simulink model "lagrange_model_v2"  (R2022a)
settings: Solver=VariableStepAuto  StartTime=0.0  StopTime=10.0  RelTol=1e-3
(part 2 of 3)

== matlab function lagrange_model_v2/MATLAB Function2 ==
  data: t input; q1 input; M_inverse output; q2 input; q3 input; q4 input; q5 input
function M_inverse = fcn(t, q1, q2, q3, q4, q5)

lb1 = 0.025; l1 = 0.110; l2 = 0.38; l3 = 0.38, l4 = 0.38; l5 = 0.04;
pi = 3.14159; beta1 = 0.3; beta2 = 0.1; beta3 = 0.1; beta4 = 0.1; beta5 = 0.1;
g = 9.81; 
m1 = 2.24036; m2 = 1.380584; m3 = 0.4927734;
m4 = 1.380584; m5 = 0.130378439395373;
% Inertia Tensor 1:
Ixx1 = 0.00602313752636761; Ixy1 = 2.1208125474502E-05; Ixz1 = 0;
Iyx1 = Ixy1; Iyy1 = 0.00579248437417585; Iyz1 = 0;
Izx1 = Ixz1; Izy1 = Iyz1; Izz1 = 0.0098329939500295;

% Inertia Tensor 2:
Ixx2 = 0.00248849839; Ixy2 = 0; Ixz2 = 0;
Iyx2 = Ixy2; Iyy2 = 0.043747624; Iyz2 = 0;
Izx2 = Ixz2; Izy2 = Iyz2; Izz = 0.0425687;

% Intertia Tensor 3:
Ixx3 = 0.000993126; Ixy3 = 0; Ixz3 = 0;
Iyx3 = Ixy3; Iyy3 = 0.0088282898; Iyz3 = 0;
Izx3 = Ixz3; Izy3 = Iyz3; Izz3 = 0.008576398866;

% Intertia Tensor 4:
Ixx4 = 0.00312638; Ixy4 = 0.00354785; Ixz4 = 0.0035964956;
Iyx4 = Ixy4; Iyy4 = 0.0434376808; Iyz4 = -0.00032350627;
Izx4 = Ixz4; Izy4 = Iyz4; Izz4 = 0.042240781;

% Intertia Tensor 5:
Ixx5 = 9.85693744749924E-05; Ixy5 = 0; Ixz5 = 0;
Iyx5 = Ixy5; Iyy5 = 0.00011697309; Iyz5 = 0;
Izx5 = Ixz5; Izy5 = Iyz5; Izz5 = 0.0001866513337855;

M11 = Izz2 + 0.49277*(5.0418e-7*cos(th1(t))*sin(th2(t)) - 0.19*cos(th3(t))*(cos(th2(t) - 1.5708)*(2.6536e-6*cos(th1(t)) + 1.0*sin(th1(t))) - 1.3268e-6*sin(th2(t) - 1.5708)*cos(th1(t))) - 0.38*cos(th2(t))*(2.6536e-6*cos(th1(t)) + 1.0*sin(th1(t))) + 0.19*sin(th3(t))*(sin(th2(t) - 1.5708)*(2.6536e-6*cos(th1(t)) + 1.0*sin(th1(t))) + 1.3268e-6*cos(th2(t) - 1.5708)*cos(th1(t))))^2 + 0.13038*(5.0418e-7*sin(th1(t))*sin(th2(t)) - 0.02*cos(th5(t))*(cos(th4(t) - 3.1416)*(cos(th3(t) - 1.5708)*(cos(th2(t) - 1.5708)*(1.0*cos(th1(t)) - 2.6536e-6*sin(th1(t))) + 1.3268e-6*sin(th2(t) - 1.5708)*sin(th1(t))) - sin(th3(t) - 1.5708)*(1.0*sin(th2(t) - 1.5708)*(1.0*cos(th1(t)) - 2.6536e-6*sin(th1(t))) - 1.3268e-6*cos(th2(t) - 1.5708)*sin(th1(t)))) + 1.0*sin(th4(t) - 3.1416)*(1.0*sin(th3(t) - 1.5708)*(cos(th2(t) - 1.5708)*(1.0*cos(th1(t)) - 2.6536e-6*sin(th1(t))) + 1.3268e-6*sin(th2(t) - 1.5708)*sin(th1(t))) + cos(th3(t) - 1.5708)*(1.0*sin(th2(t) - 1.5708)*(1.0*cos(th1(t)) - 2.6536e-6*sin(th1(t))) - 1.3268e-6*cos(th2(t) - 1.5708)*sin(th1(t))))) + 0.38*cos(th2(t))*(1.0*cos(th1(t)) - 2.6536e-6*sin(th1(t))) + 0.38*cos(th3(t))*(cos(th2(t) - 1.5708)*(1.0*cos(th1(t)) - 2.6536e-6*sin(th1(t))) + 1.3268e-6*sin(th2(t) - 1.5708)*sin(th1(t))) + 0.38*cos(th4(t))*(cos(th3(t) - 1.5708)*(cos(th2(t) - 1.5708)*(1.0*cos(th1(t)) - 2.6536e-6*sin(th1(t))) + 1.3268e-6*sin(th2(t) - 1.5708)*sin(th1(t))) - sin(th3(t) - 1.5708)*(1.0*sin(th2(t) - 1.5708)*(1.0*cos(th1(t)) - 2.6536e-6*sin(th1(t))) - 1.3268e-6*cos(th2(t) - 1.5708)*sin(th1(t)))) - 0.38*sin(th3(t))*(1.0*sin(th2(t) - 1.5708)*(1.0*cos(th1(t)) - 2.6536e-6*sin(th1(t))) - 1.3268e-6*cos(th2(t) - 1.5708)*sin(th1(t))) - 0.38*sin(th4(t))*(1.0*sin(th3(t) - 1.5708)*(cos(th2(t) - 1.5708)*(1.0*cos(th1(t)) - 2.6536e-6*sin(th1(t))) + 1.3268e-6*sin(th2(t) - 1.5708)*sin(th1(t))) + cos(th3(t) - 1.5708)*(1.0*sin(th2(t) - 1.5708)*(1.0*cos(th1(t)) - 2.6536e-6*sin(th1(t))) - 1.3268e-6*cos(th2(t) - 1.5708)*sin(th1(t)))) - 0.02*sin(th5(t))*(sin(th4(t) - 3.1416)*(cos(th3(t) - 1.5708)*(cos(th2(t) - 1.5708)*(1.0*cos(th1(t)) - 2.6536e-6*sin(th1(t))) + 1.3268e-6*sin(th2(t) - 1.5708)*sin(th1(t))) - sin(th3(t) - 1.5708)*(1.0*sin(th2(t) - 1.5708)*(1.0*cos(th1(t)) - 2.6536e-6*sin(th1(t))) - 1.3268e-6*cos(th2(t) - 1.5708)*sin(th1(t)))) - cos(th4(t) - 3.1416)*(1.0*sin(th3(t) - 1.5708)*(cos(th2(t) - 1.5708)*(1.0*cos(th1(t)) - 2.6536e-6*sin(th1(t))) + 1.3268e-6*sin(th2(t) - 1.5708)*sin(th1(t))) + cos(th3(t) - 1.5708)*(1.0*sin(th2(t) - 1.5708)*(1.0*cos(th1(t)) - 2.6536e-6*sin(th1(t))) - 1.3268e-6*cos(th2(t) - 1.5708)*sin(th1(t))))))^2 + 1.3806*(5.0418e-7*cos(th1(t))*sin(th2(t)) + 0.19*sin(th4(t))*(cos(th3(t) - 1.5708)*(sin(th2(t) - 1.5708)*(2.6536e-6*cos(th1(t)) + 1.0*sin(th1(t))) + 1.3268e-6*cos(th2(t) - 1.5708)*cos(th1(t))) + sin(th3(t) - 1.5708)*(cos(th2(t) - 1.5708)*(2.6536e-6*cos(th1(t)) + 1.0*sin(th1(t))) - 1.3268e-6*sin(th2(t) - 1.5708)*cos(th1(t)))) - 0.38*cos(th3(t))*(cos(th2(t) - 1.5708)*(2.6536e-6*cos(th1(t)) + 1.0*sin(th1(t))) - 1.3268e-6*sin(th2(t) - 1.5708)*cos(th1(t))) - 0.38*cos(th2(t))*(2.6536e-6*cos(th1(t)) + 1.0*sin(th1(t))) + 0.38*sin(th3(t))*(sin(th2(t) - 1.5708)*(2.6536e-6*cos(th1(t)) + 1.0*sin(th1(t))) + 1.3268e-6*cos(th2(t) - 1.5708)*cos(th1(t))) - 0.19*cos(th4(t))*(cos(th3(t) - 1.5708)*(cos(th2(t) - 1.5708)*(2.6536e-6*cos(th1(t)) + 1.0*sin(th1(t))) - 1.3268e-6*sin(th2(t) - 1.5708)*cos(th1(t))) - 1.0*sin(th3(t) - 1.5708)*(sin(th2(t) - 1.5708)*(2.6536e-6*cos(th1(t)) + 1.0*sin(th1(t))) + 1.3268e-6*cos(th2(t) - 1.5708)*cos(th1(t)))))^2 + 0.49277*(5.0418e-7*sin(th1(t))*sin(th2(t)) + 0.38*cos(th2(t))*(1.0*cos(th1(t)) - 2.6536e-6*sin(th1(t))) + 0.19*cos(th3(t))*(cos(th2(t) - 1.5708)*(1.0*cos(th1(t)) - 2.6536e-6*sin(th1(t))) + 1.3268e-6*sin(th2(t) - 1.5708)*sin(th1(t))) - 0.19*sin(th3(t))*(1.0*sin(th2(t) - 1.5708)*(1.0*cos(th1(t)) - 2.6536e-6*sin(th1(t))) - 1.3268e-6*cos(th2(t) - 1.5708)*sin(th1(t))))^2 + 0.13038*(5.0418e-7*cos(th1(t))*sin(th2(t)) + 0.02*cos(th5(t))*(cos(th4(t) - 3.1416)*(cos(th3(t) - 1.5708)*(cos(th2(t) - 1.5708)*(2.6536e-6*cos(th1(t)) + 1.0*sin(th1(t))) - 1.3268e-6*sin(th2(t) - 1.5708)*cos(th1(t))) - 1.0*sin(th3(t) - 1.5708)*(sin(th2(t) - 1.5708)*(2.6536e-6*cos(th1(t)) + 1.0*sin(th1(t))) + 1.3268e-6*cos(th2(t) - 1.5708)*cos(th1(t)))) + sin(th4(t) - 3.1416)*(cos(th3(t) - 1.5708)*(sin(th2(t) - 1.5708)*(2.6536e-6*cos(th1(t)) + 1.0*sin(th1(t))) + 1.3268e-6*cos(th2(t) - 1.5708)*cos(th1(t))) + sin(th3(t) - 1.5708)*(cos(th2(t) - 1.5708)*(2.6536e-6*cos(th1(t)) + 1.0*sin(th1(t))) - 1.3268e-6*sin(th2(t) - 1.5708)*cos(th1(t))))) + 0.38*sin(th4(t))*(cos(th3(t) - 1.5708)*(sin(th2(t) - 1.5708)*(2.6536e-6*cos(th1(t)) + 1.0*sin(th1(t))) + 1.3268e-6*cos(th2(t) - 1.5708)*cos(th1(t))) + sin(th3(t) - 1.5708)*(cos(th2(t) - 1.5708)*(2.6536e-6*cos(th1(t)) + 1.0*sin(th1(t))) - 1.3268e-6*sin(th2(t) - 1.5708)*cos(th1(t)))) - 0.38*cos(th3(t))*(cos(th2(t) - 1.5708)*(2.6536e-6*cos(th1(t)) + 1.0*sin(th1(t))) - 1.3268e-6*sin(th2(t) - 1.5708)*cos(th1(t))) - 0.38*cos(th2(t))*(2.6536e-6*cos(th1(t)) + 1.0*sin(th1(t))) + 0.38*sin(th3(t))*(sin(th2(t) - 1.5708)*(2.6536e-6*cos(th1(t)) + 1.0*sin(th1(t))) + 1.3268e-6*cos(th2(t) - 1.5708)*cos(th1(t))) - 0.38*cos(th4(t))*(cos(th3(t) - 1.5708)*(cos(th2(t) - 1.5708)*(2.6536e-6*cos(th1(t)) + 1.0*sin(th1(t))) - 1.3268e-6*sin(th2(t) - 1.5708)*cos(th1(t))) - 1.0*sin(th3(t) - 1.5708)*(sin(th2(t) - 1.5708)*(2.6536e-6*cos(th1(t)) + 1.0*sin(th1(t))) + 1.3268e-6*cos(th2(t) - 1.5708)*cos(th1(t)))) + 0.02*sin(th5(t))*(1.0*sin(th4(t) - 3.1416)*(cos(th3(t) - 1.5708)*(cos(th2(t) - 1.5708)*(2.6536e-6*cos(th1(t)) + 1.0*sin(th1(t))) - 1.3268e-6*sin(th2(t) - 1.5708)*cos(th1(t))) - 1.0*sin(th3(t) - 1.5708)*(sin(th2(t) - 1.5708)*(2.6536e-6*cos(th1(t)) + 1.0*sin(th1(t))) + 1.3268e-6*cos(th2(t) - 1.5708)*cos(th1(t)))) - cos(th4(t) - 3.1416)*(cos(th3(t) - 1.5708)*(sin(th2(t) - 1.5708)*(2.6536e-6*cos(th1(t)) + 1.0*sin(th1(t))) + 1.3268e-6*cos(th2(t) - 1.5708)*cos(th1(t))) + sin(th3(t) - 1.5708)*(cos(th2(t) - 1.5708)*(2.6536e-6*cos(th1(t)) + 1.0*sin(th1(t))) - 1.3268e-6*sin(th2(t) - 1.5708)*cos(th1(t))))))^2 + 1.3806*(5.0418e-7*sin(th1(t))*sin(th2(t)) + 0.38*cos(th2(t))*(1.0*cos(th1(t)) - 2.6536e-6*sin(th1(t))) + 0.38*cos(th3(t))*(cos(th2(t) - 1.5708)*(1.0*cos(th1(t)) - 2.6536e-6*sin(th1(t))) + 1.3268e-6*sin(th2(t) - 1.5708)*sin(th1(t))) + 0.19*cos(th4(t))*(cos(th3(t) - 1.5708)*(cos(th2(t) - 1.5708)*(1.0*cos(th1(t)) - 2.6536e-6*sin(th1(t))) + 1.3268e-6*sin(th2(t) - 1.5708)*sin(th1(t))) - sin(th3(t) - 1.5708)*(1.0*sin(th2(t) - 1.5708)*(1.0*cos(th1(t)) - 2.6536e-6*sin(th1(t))) - 1.3268e-6*cos(th2(t) - 1.5708)*sin(th1(t)))) - 0.38*sin(th3(t))*(1.0*sin(th2(t) - 1.5708)*(1.0*cos(th1(t)) - 2.6536e-6*sin(th1(t))) - 1.3268e-6*cos(th2(t) - 1.5708)*sin(th1(t))) - 0.19*sin(th4(t))*(1.0*sin(th3(t) - 1.5708)*(cos(th2(t) - 1.5708)*(1.0*cos(th1(t)) - 2.6536e-6*sin(th1(t))) + 1.3268e-6*sin(th2(t) - 1.5708)*sin(th1(t))) + cos(th3(t) - 1.5708)*(1.0*sin(th2(t) - 1.5708)*(1.0*cos(th1(t)) - 2.6536e-6*sin(th1(t))) - 1.3268e-6*cos(th2(t) - 1.5708)*sin(th1(t)))))^2 + 1.3806*(2.5209e-7*cos(th1(t))*sin(th2(t)) - 0.19*cos(th2(t))*(2.6536e-6*cos(th1(t)) + 1.0*sin(th1(t))))^2 + 1.3806*(2.5209e-7*sin(th1(t))*sin(th2(t)) + 0.19*cos(th2(t))*(1.0*cos(th1(t)) - 2.6536e-6*sin(th1(t))))^2 + 0.060837;
M12 = Izz2 - 0.13038*(5.0418e-7*sin(th1(t))*sin(th2(t)) - 0.02*cos(th5(t))*(cos(th4(t) - 3.1416)*(cos(th3(t) - 1.5708)*(cos(th2(t) - 1.5708)*(1.0*cos(th1(t)) - 2.6536e-6*sin(th1(t))) + 1.3268e-6*sin(th2(t) - 1.5708)*sin(th1(t))) - sin(th3(t) - 1.5708)*(1.0*sin(th2(t) - 1.5708)*(1.0*cos(th1(t)) - 2.6536e-6*sin(th1(t))) - 1.3268e-6*cos(th2(t) - 1.5708)*sin(th1(t)))) + 1.0*sin(th4(t) - 3.1416)*(1.0*sin(th3(t) - 1.5708)*(cos(th2(t) - 1.5708)*(1.0*cos(th1(t)) - 2.6536e-6*sin(th1(t))) + 1.3268e-6*sin(th2(t) - 1.5708)*sin(th1(t))) + cos(th3(t) - 1.5708)*(1.0*sin(th2(t) - 1.5708)*(1.0*cos(th1(t)) - 2.6536e-6*sin(th1(t))) - 1.3268e-6*cos(th2(t) - 1.5708)*sin(th1(t))))) + 0.38*cos(th2(t))*(1.0*cos(th1(t)) - 2.6536e-6*sin(th1(t))) + 0.38*cos(th3(t))*(cos(th2(t) - 1.5708)*(1.0*cos(th1(t)) - 2.6536e-6*sin(th1(t))) + 1.3268e-6*sin(th2(t) - 1.5708)*sin(th1(t))) + 0.38*cos(th4(t))*(cos(th3(t) - 1.5708)*(cos(th2(t) - 1.5708)*(1.0*cos(th1(t)) - 2.6536e-6*sin(th1(t))) + 1.3268e-6*sin(th2(t) - 1.5708)*sin(th1(t))) - sin(th3(t) - 1.5708)*(1.0*sin(th2(t) - 1.5708)*(1.0*cos(th1(t)) - 2.6536e-6*sin(th1(t))) - 1.3268e-6*cos(th2(t) - 1.5708)*sin(th1(t)))) - 0.38*sin(th3(t))*(1.0*sin(th2(t) - 1.5708)*(1.0*cos(th1(t)) - 2.6536e-6*sin(th1(t))) - 1.3268e-6*cos(th2(t) - 1.5708)*sin(th1(t))) - 0.38*sin(th4(t))*(1.0*sin(th3(t) - 1.5708)*(cos(th2(t) - 1.5708)*(1.0*cos(th1(t)) - 2.6536e-6*sin(th1(t))) + 1.3268e-6*sin(th2(t) - 1.5708)*sin(th1(t))) + cos(th3(t) - 1.5708)*(1.0*sin(th2(t) - 1.5708)*(1.0*cos(th1(t)) - 2.6536e-6*sin(th1(t))) - 1.3268e-6*cos(th2(t) - 1.5708)*sin(th1(t)))) - 0.02*sin(th5(t))*(sin(th4(t) - 3.1416)*(cos(th3(t) - 1.5708)*(cos(th2(t) - 1.5708)*(1.0*cos(th1(t)) - 2.6536e-6*sin(th1(t))) + 1.3268e-6*sin(th2(t) - 1.5708)*sin(th1(t))) - sin(th3(t) - 1.5708)*(1.0*sin(th2(t) - 1.5708)*(1.0*cos(th1(t)) - 2.6536e-6*sin(th1(t))) - 1.3268e-6*cos(th2(t) - 1.5708)*sin(th1(t)))) - cos(th4(t) - 3.1416)*(1.0*sin(th3(t) - 1.5708)*(cos(th2(t) - 1.5708)*(1.0*cos(th1(t)) - 2.6536e-6*sin(th1(t))) + 1.3268e-6*sin(th2(t) - 1.5708)*sin(th1(t))) + cos(th3(t) - 1.5708)*(1.0*sin(th2(t) - 1.5708)*(1.0*cos(th1(t)) - 2.6536e-6*sin(th1(t))) - 1.3268e-6*cos(th2(t) - 1.5708)*sin(th1(t))))))*(0.38*cos(th3(t))*(sin(th2(t) - 1.5708)*(2.6536e-6*cos(th1(t)) + 1.0*sin(th1(t))) + 1.3268e-6*cos(th2(t) - 1.5708)*cos(th1(t))) + 0.38*sin(th2(t))*(2.6536e-6*cos(th1(t)) + 1.0*sin(th1(t))) - 0.38*sin(th4(t))*(sin(th3(t) - 1.5708)*(sin(th2(t) - 1.5708)*(2.6536e-6*cos(th1(t)) + 1.0*sin(th1(t))) + 1.3268e-6*cos(th2(t) - 1.5708)*cos(th1(t))) - cos(th3(t) - 1.5708)*(1.0*cos(th2(t) - 1.5708)*(2.6536e-6*cos(th1(t)) + 1.0*sin(th1(t))) - 1.3268e-6*sin(th2(t) - 1.5708)*cos(th1(t)))) + 0.38*sin(th3(t))*(1.0*cos(th2(t) - 1.5708)*(2.6536e-6*cos(th1(t)) + 1.0*sin(th1(t))) - 1.3268e-6*sin(th2(t) - 1.5708)*cos(th1(t))) - 0.02*cos(th5(t))*(sin(th4(t) - 3.1416)*(sin(th3(t) - 1.5708)*(sin(th2(t) - 1.5708)*(2.6536e-6*cos(th1(t)) + 1.0*sin(th1(t))) + 1.3268e-6*cos(th2(t) - 1.5708)*cos(th1(t))) - cos(th3(t) - 1.5708)*(1.0*cos(th2(t) - 1.5708)*(2.6536e-6*cos(th1(t)) + 1.0*sin(th1(t))) - 1.3268e-6*sin(th2(t) - 1.5708)*cos(th1(t)))) + cos(th4(t) - 3.1416)*(cos(th3(t) - 1.5708)*(sin(th2(t) - 1.5708)*(2.6536e-6*cos(th1(t)) + 1.0*sin(th1(t))) + 1.3268e-6*cos(th2(t) - 1.5708)*cos(th1(t))) + 1.0*sin(th3(t) - 1.5708)*(1.0*cos(th2(t) - 1.5708)*(2.6536e-6*cos(th1(t)) + 1.0*sin(th1(t))) - 1.3268e-6*sin(th2(t) - 1.5708)*cos(th1(t))))) + 0.38*cos(th4(t))*(cos(th3(t) - 1.5708)*(sin(th2(t) - 1.5708)*(2.6536e-6*cos(th1(t)) + 1.0*sin(th1(t))) + 1.3268e-6*cos(th2(t) - 1.5708)*cos(th1(t))) + 1.0*sin(th3(t) - 1.5708)*(1.0*cos(th2(t) - 1.5708)*(2.6536e-6*cos(th1(t)) + 1.0*sin(th1(t))) - 1.3268e-6*sin(th2(t) - 1.5708)*cos(th1(t)))) + 0.02*sin(th5(t))*(cos(th4(t) - 3.1416)*(sin(th3(t) - 1.5708)*(sin(th2(t) - 1.5708)*(2.6536e-6*cos(th1(t)) + 1.0*sin(th1(t))) + 1.3268e-6*cos(th2(t) - 1.5708)*cos(th1(t))) - cos(th3(t) - 1.5708)*(1.0*cos(th2(t) - 1.5708)*(2.6536e-6*cos(th1(t)) + 1.0*sin(th1(t))) - 1.3268e-6*sin(th2(t) - 1.5708)*cos(th1(t)))) - 1.0*sin(th4(t) - 3.1416)*(cos(th3(t) - 1.5708)*(sin(th2(t) - 1.5708)*(2.6536e-6*cos(th1(t)) + 1.0*sin(th1(t))) + 1.3268e-6*cos(th2(t) - 1.5708)*cos(th1(t))) + 1.0*sin(th3(t) - 1.5708)*(1.0*cos(th2(t) - 1.5708)*(2.6536e-6*cos(th1(t)) + 1.0*sin(th1(t))) - 1.3268e-6*sin(th2(t) - 1.5708)*cos(th1(t))))) + 5.0418e-7*cos(th1(t))*cos(th2(t))) + 1.3806*(2.5209e-7*cos(th1(t))*sin(th2(t)) - 0.19*cos(th2(t))*(2.6536e-6*cos(th1(t)) + 1.0*sin(th1(t))))*(2.5209e-7*cos(th2(t))*sin(th1(t)) - 0.19*sin(th2(t))*(1.0*cos(th1(t)) - 2.6536e-6*sin(th1(t)))) - 1.3806*(0.19*sin(th2(t))*(2.6536e-6*cos(th1(t)) + 1.0*sin(th1(t))) + 2.5209e-7*cos(th1(t))*cos(th2(t)))*(2.5209e-7*sin(th1(t))*sin(th2(t)) + 0.19*cos(th2(t))*(1.0*cos(th1(t)) - 2.6536e-6*sin(th1(t)))) - 1.3806*(5.0418e-7*sin(th1(t))*sin(th2(t)) + 0.38*cos(th2(t))*(1.0*cos(th1(t)) - 2.6536e-6*sin(th1(t))) + 0.38*cos(th3(t))*(cos(th2(t) - 1.5708)*(1.0*cos(th1(t)) - 2.6536e-6*sin(th1(t))) + 1.3268e-6*sin(th2(t) - 1.5708)*sin(th1(t))) + 0.19*cos(th4(t))*(cos(th3(t) - 1.5708)*(cos(th2(t) - 1.5708)*(1.0*cos(th1(t)) - 2.6536e-6*sin(th1(t))) + 1.3268e-6*sin(th2(t) - 1.5708)*sin(th1(t))) - sin(th3(t) - 1.5708)*(1.0*sin(th2(t) - 1.5708)*(1.0*cos(th1(t)) - 2.6536e-6*sin(th1(t))) - 1.3268e-6*cos(th2(t) - 1.5708)*sin(th1(t)))) - 0.38*sin(th3(t))*(1.0*sin(th2(t) - 1.5708)*(1.0*cos(th1(t)) - 2.6536e-6*sin(th1(t))) - 1.3268e-6*cos(th2(t) - 1.5708)*sin(th1(t))) - 0.19*sin(th4(t))*(1.0*sin(th3(t) - 1.5708)*(cos(th2(t) - 1.5708)*(1.0*cos(th1(t)) - 2.6536e-6*sin(th1(t))) + 1.3268e-6*sin(th2(t) - 1.5708)*sin(th1(t))) + cos(th3(t) - 1.5708)*(1.0*sin(th2(t) - 1.5708)*(1.0*cos(th1(t)) - 2.6536e-6*sin(th1(t))) - 1.3268e-6*cos(th2(t) - 1.5708)*sin(th1(t)))))*(0.38*cos(th3(t))*(sin(th2(t) - 1.5708)*(2.6536e-6*cos(th1(t)) + 1.0*sin(th1(t))) + 1.3268e-6*cos(th2(t) - 1.5708)*cos(th1(t))) + 0.38*sin(th2(t))*(2.6536e-6*cos(th1(t)) + 1.0*sin(th1(t))) - 0.19*sin(th4(t))*(sin(th3(t) - 1.5708)*(sin(th2(t) - 1.5708)*(2.6536e-6*cos(th1(t)) + 1.0*sin(th1(t))) + 1.3268e-6*cos(th2(t) - 1.5708)*cos(th1(t))) - cos(th3(t) - 1.5708)*(1.0*cos(th2(t) - 1.5708)*(2.6536e-6*cos(th1(t)) + 1.0*sin(th1(t))) - 1.3268e-6*sin(th2(t) - 1.5708)*cos(th1(t)))) + 0.38*sin(th3(t))*(1.0*cos(th2(t) - 1.5708)*(2.6536e-6*cos(th1(t)) + 1.0*sin(th1(t))) - 1.3268e-6*sin(th2(t) - 1.5708)*cos(th1(t))) + 0.19*cos(th4(t))*(cos(th3(t) - 1.5708)*(sin(th2(t) - 1.5708)*(2.6536e-6*cos(th1(t)) + 1.0*sin(th1(t))) + 1.3268e-6*cos(th2(t) - 1.5708)*cos(th1(t))) + 1.0*sin(th3(t) - 1.5708)*(1.0*cos(th2(t) - 1.5708)*(2.6536e-6*cos(th1(t)) + 1.0*sin(th1(t))) - 1.3268e-6*sin(th2(t) - 1.5708)*cos(th1(t)))) + 5.0418e-7*cos(th1(t))*cos(th2(t))) - 0.49277*(5.0418e-7*sin(th1(t))*sin(th2(t)) + 0.38*cos(th2(t))*(1.0*cos(th1(t)) - 2.6536e-6*sin(th1(t))) + 0.19*cos(th3(t))*(cos(th2(t) - 1.5708)*(1.0*cos(th1(t)) - 2.6536e-6*sin(th1(t))) + 1.3268e-6*sin(th2(t) - 1.5708)*sin(th1(t))) - 0.19*sin(th3(t))*(1.0*sin(th2(t) - 1.5708)*(1.0*cos(th1(t)) - 2.6536e-6*sin(th1(t))) - 1.3268e-6*cos(th2(t) - 1.5708)*sin(th1(t))))*(0.19*cos(th3(t))*(sin(th2(t) - 1.5708)*(2.6536e-6*cos(th1(t)) + 1.0*sin(th1(t))) + 1.3268e-6*cos(th2(t) - 1.5708)*cos(th1(t))) + 0.38*sin(th2(t))*(2.6536e-6*cos(th1(t)) + 1.0*sin(th1(t))) + 0.19*sin(th3(t))*(1.0*cos(th2(t) - 1.5708)*(2.6536e-6*cos(th1(t)) + 1.0*sin(th1(t))) - 1.3268e-6*sin(th2(t) - 1.5708)*cos(th1(t))) + 5.0418e-7*cos(th1(t))*cos(th2(t))) - 0.13038*(0.38*cos(th4(t))*(cos(th3(t) - 1.5708)*(sin(th2(t) - 1.5708)*(1.0*cos(th1(t)) - 2.6536e-6*sin(th1(t))) - 1.3268e-6*cos(th2(t) - 1.5708)*sin(th1(t))) + sin(th3(t) - 1.5708)*(cos(th2(t) - 1.5708)*(1.0*cos(th1(t)) - 2.6536e-6*sin(th1(t))) + 1.3268e-6*sin(th2(t) - 1.5708)*sin(th1(t)))) - 5.0418e-7*cos(th2(t))*sin(th1(t)) + 0.38*cos(th3(t))*(sin(th2(t) - 1.5708)*(1.0*cos(th1(t)) - 2.6536e-6*sin(th1(t))) - 1.3268e-6*cos(th2(t) - 1.5708)*sin(th1(t))) + 0.38*sin(th2(t))*(1.0*cos(th1(t)) - 2.6536e-6*sin(th1(t))) + 0.38*sin(th3(t))*(cos(th2(t) - 1.5708)*(1.0*cos(th1(t)) - 2.6536e-6*sin(th1(t))) + 1.3268e-6*sin(th2(t) - 1.5708)*sin(th1(t))) - 0.02*sin(th5(t))*(sin(th4(t) - 3.1416)*(cos(th3(t) - 1.5708)*(sin(th2(t) - 1.5708)*(1.0*cos(th1(t)) - 2.6536e-6*sin(th1(t))) - 1.3268e-6*cos(th2(t) - 1.5708)*sin(th1(t))) + sin(th3(t) - 1.5708)*(cos(th2(t) - 1.5708)*(1.0*cos(th1(t)) - 2.6536e-6*sin(th1(t))) + 1.3268e-6*sin(th2(t) - 1.5708)*sin(th1(t)))) + cos(th4(t) - 3.1416)*(cos(th3(t) - 1.5708)*(cos(th2(t) - 1.5708)*(1.0*cos(th1(t)) - 2.6536e-6*sin(th1(t))) + 1.3268e-6*sin(th2(t) - 1.5708)*sin(th1(t))) - 1.0*sin(th3(t) - 1.5708)*(sin(th2(t) - 1.5708)*(1.0*cos(th1(t)) - 2.6536e-6*sin(th1(t))) - 1.3268e-6*cos(th2(t) - 1.5708)*sin(th1(t))))) + 0.38*sin(th4(t))*(cos(th3(t) - 1.5708)*(cos(th2(t) - 1.5708)*(1.0*cos(th1(t)) - 2.6536e-6*sin(th1(t))) + 1.3268e-6*sin(th2(t) - 1.5708)*sin(th1(t))) - 1.0*sin(th3(t) - 1.5708)*(sin(th2(t) - 1.5708)*(1.0*cos(th1(t)) - 2.6536e-6*sin(th1(t))) - 1.3268e-6*cos(th2(t) - 1.5708)*sin(th1(t)))) - 0.02*cos(th5(t))*(cos(th4(t) - 3.1416)*(cos(th3(t) - 1.5708)*(sin(th2(t) - 1.5708)*(1.0*cos(th1(t)) - 2.6536e-6*sin(th1(t))) - 1.3268e-6*cos(th2(t) - 1.5708)*sin(th1(t))) + sin(th3(t) - 1.5708)*(cos(th2(t) - 1.5708)*(1.0*cos(th1(t)) - 2.6536e-6*sin(th1(t))) + 1.3268e-6*sin(th2(t) - 1.5708)*sin(th1(t)))) - 1.0*sin(th4(t) - 3.1416)*(cos(th3(t) - 1.5708)*(cos(th2(t) - 1.5708)*(1.0*cos(th1(t)) - 2.6536e-6*sin(th1(t))) + 1.3268e-6*sin(th2(t) - 1.5708)*sin(th1(t))) - 1.0*sin(th3(t) - 1.5708)*(sin(th2(t) - 1.5708)*(1.0*cos(th1(t)) - 2.6536e-6*sin(th1(t))) - 1.3268e-6*cos(th2(t) - 1.5708)*sin(th1(t))))))*(5.0418e-7*cos(th1(t))*sin(th2(t)) + 0.02*cos(th5(t))*(cos(th4(t) - 3.1416)*(cos(th3(t) - 1.5708)*(cos(th2(t) - 1.5708)*(2.6536e-6*cos(th1(t)) + 1.0*sin(th1(t))) - 1.3268e-6*sin(th2(t) - 1.5708)*cos(th1(t))) - 1.0*sin(th3(t) - 1.5708)*(sin(th2(t) - 1.5708)*(2.6536e-6*cos(th1(t)) + 1.0*sin(th1(t))) + 1.3268e-6*cos(th2(t) - 1.5708)*cos(th1(t)))) + sin(th4(t) - 3.1416)*(cos(th3(t) - 1.5708)*(sin(th2(t) - 1.5708)*(2.6536e-6*cos(th1(t)) + 1.0*sin(th1(t))) + 1.3268e-6*cos(th2(t) - 1.5708)*cos(th1(t))) + sin(th3(t) - 1.5708)*(cos(th2(t) - 1.5708)*(2.6536e-6*cos(th1(t)) + 1.0*sin(th1(t))) - 1.3268e-6*sin(th2(t) - 1.5708)*cos(th1(t))))) + 0.38*sin(th4(t))*(cos(th3(t) - 1.5708)*(sin(th2(t) - 1.5708)*(2.6536e-6*cos(th1(t)) + 1.0*sin(th1(t))) + 1.3268e-6*cos(th2(t) - 1.5708)*cos(th1(t))) + sin(th3(t) - 1.5708)*(cos(th2(t) - 1.5708)*(2.6536e-6*cos(th1(t)) + 1.0*sin(th1(t))) - 1.3268e-6*sin(th2(t) - 1.5708)*cos(th1(t)))) - 0.38*cos(th3(t))*(cos(th2(t) - 1.5708)*(2.6536e-6*cos(th1(t)) + 1.0*sin(th1(t))) - 1.3268e-6*sin(th2(t) - 1.5708)*cos(th1(t))) - 0.38*cos(th2(t))*(2.6536e-6*cos(th1(t)) + 1.0*sin(th1(t))) + 0.38*sin(th3(t))*(sin(th2(t) - 1.5708)*(2.6536e-6*cos(th1(t)) + 1.0*sin(th1(t))) + 1.3268e-6*cos(th2(t) - 1.5708)*cos(th1(t))) - 0.38*cos(th4(t))*(cos(th3(t) - 1.5708)*(cos(th2(t) - 1.5708)*(2.6536e-6*cos(th1(t)) + 1.0*sin(th1(t))) - 1.3268e-6*sin(th2(t) - 1.5708)*cos(th1(t))) - 1.0*sin(th3(t) - 1.5708)*(sin(th2(t) - 1.5708)*(2.6536e-6*cos(th1(t)) + 1.0*sin(th1(t))) + 1.3268e-6*cos(th2(t) - 1.5708)*cos(th1(t)))) + 0.02*sin(th5(t))*(1.0*sin(th4(t) - 3.1416)*(cos(th3(t) - 1.5708)*(cos(th2(t) - 1.5708)*(2.6536e-6*cos(th1(t)) + 1.0*sin(th1(t))) - 1.3268e-6*sin(th2(t) - 1.5708)*cos(th1(t))) - 1.0*sin(th3(t) - 1.5708)*(sin(th2(t) - 1.5708)*(2.6536e-6*cos(th1(t)) + 1.0*sin(th1(t))) + 1.3268e-6*cos(th2(t) - 1.5708)*cos(th1(t)))) - cos(th4(t) - 3.1416)*(cos(th3(t) - 1.5708)*(sin(th2(t) - 1.5708)*(2.6536e-6*cos(th1(t)) + 1.0*sin(th1(t))) + 1.3268e-6*cos(th2(t) - 1.5708)*cos(th1(t))) + sin(th3(t) - 1.5708)*(cos(th2(t) - 1.5708)*(2.6536e-6*cos(th1(t)) + 1.0*sin(th1(t))) - 1.3268e-6*sin(th2(t) - 1.5708)*cos(th1(t)))))) - 1.3806*(0.19*cos(th4(t))*(cos(th3(t) - 1.5708)*(sin(th2(t) - 1.5708)*(1.0*cos(th1(t)) - 2.6536e-6*sin(th1(t))) - 1.3268e-6*cos(th2(t) - 1.5708)*sin(th1(t))) + sin(th3(t) - 1.5708)*(cos(th2(t) - 1.5708)*(1.0*cos(th1(t)) - 2.6536e-6*sin(th1(t))) + 1.3268e-6*sin(th2(t) - 1.5708)*sin(th1(t)))) - 5.0418e-7*cos(th2(t))*sin(th1(t)) + 0.38*cos(th3(t))*(sin(th2(t) - 1.5708)*(1.0*cos(th1(t)) - 2.6536e-6*sin(th1(t))) - 1.3268e-6*cos(th2(t) - 1.5708)*sin(th1(t))) + 0.38*sin(th2(t))*(1.0*cos(th1(t)) - 2.6536e-6*sin(th1(t))) + 0.38*sin(th3(t))*(cos(th2(t) - 1.5708)*(1.0*cos(th1(t)) - 2.6536e-6*sin(th1(t))) + 1.3268e-6*sin(th2(t) - 1.5708)*sin(th1(t))) + 0.19*sin(th4(t))*(cos(th3(t) - 1.5708)*(cos(th2(t) - 1.5708)*(1.0*cos(th1(t)) - 2.6536e-6*sin(th1(t))) + 1.3268e-6*sin(th2(t) - 1.5708)*sin(th1(t))) - 1.0*sin(th3(t) - 1.5708)*(sin(th2(t) - 1.5708)*(1.0*cos(th1(t)) - 2.6536e-6*sin(th1(t))) - 1.3268e-6*cos(th2(t) - 1.5708)*sin(th1(t)))))*(5.0418e-7*cos(th1(t))*sin(th2(t)) + 0.19*sin(th4(t))*(cos(th3(t) - 1.5708)*(sin(th2(t) - 1.5708)*(2.6536e-6*cos(th1(t)) + 1.0*sin(th1(t))) + 1.3268e-6*cos(th2(t) - 1.5708)*cos(th1(t))) + sin(th3(t) - 1.5708)*(cos(th2(t) - 1.5708)*(2.6536e-6*cos(th1(t)) + 1.0*sin(th1(t))) - 1.3268e-6*sin(th2(t) - 1.5708)*cos(th1(t)))) - 0.38*cos(th3(t))*(cos(th2(t) - 1.5708)*(2.6536e-6*cos(th1(t)) + 1.0*sin(th1(t))) - 1.3268e-6*sin(th2(t) - 1.5708)*cos(th1(t))) - 0.38*cos(th2(t))*(2.6536e-6*cos(th1(t)) + 1.0*sin(th1(t))) + 0.38*sin(th3(t))*(sin(th2(t) - 1.5708)*(2.6536e-6*cos(th1(t)) + 1.0*sin(th1(t))) + 1.3268e-6*cos(th2(t) - 1.5708)*cos(th1(t))) - 0.19*cos(th4(t))*(cos(th3(t) - 1.5708)*(cos(th2(t) - 1.5708)*(2.6536e-6*cos(th1(t)) + 1.0*sin(th1(t))) - 1.3268e-6*sin(th2(t) - 1.5708)*cos(th1(t))) - 1.0*sin(th3(t) - 1.5708)*(sin(th2(t) - 1.5708)*(2.6536e-6*cos(th1(t)) + 1.0*sin(th1(t))) + 1.3268e-6*cos(th2(t) - 1.5708)*cos(th1(t))))) - 0.49277*(5.0418e-7*cos(th1(t))*sin(th2(t)) - 0.19*cos(th3(t))*(cos(th2(t) - 1.5708)*(2.6536e-6*cos(th1(t)) + 1.0*sin(th1(t))) - 1.3268e-6*sin(th2(t) - 1.5708)*cos(th1(t))) - 0.38*cos(th2(t))*(2.6536e-6*cos(th1(t)) + 1.0*sin(th1(t))) + 0.19*sin(th3(t))*(sin(th2(t) - 1.5708)*(2.6536e-6*cos(th1(t)) + 1.0*sin(th1(t))) + 1.3268e-6*cos(th2(t) - 1.5708)*cos(th1(t))))*(0.19*cos(th3(t))*(sin(th2(t) - 1.5708)*(1.0*cos(th1(t)) - 2.6536e-6*sin(th1(t))) - 1.3268e-6*cos(th2(t) - 1.5708)*sin(th1(t))) - 5.0418e-7*cos(th2(t))*sin(th1(t)) + 0.38*sin(th2(t))*(1.0*cos(th1(t)) - 2.6536e-6*sin(th1(t))) + 0.19*sin(th3(t))*(cos(th2(t) - 1.5708)*(1.0*cos(th1(t)) - 2.6536e-6*sin(th1(t))) + 1.3268e-6*sin(th2(t) - 1.5708)*sin(th1(t)))) + 0.051004;
M13 = 0.051004 - 1.3806*(0.38*cos(th3(t))*(sin(th2(t) - 1.5708)*(2.6536e-6*cos(th1(t)) + 1.0*sin(th1(t))) + 1.3268e-6*cos(th2(t) - 1.5708)*cos(th1(t))) - 0.19*sin(th4(t))*(sin(th3(t) - 1.5708)*(sin(th2(t) - 1.5708)*(2.6536e-6*cos(th1(t)) + 1.0*sin(th1(t))) + 1.3268e-6*cos(th2(t) - 1.5708)*cos(th1(t))) - cos(th3(t) - 1.5708)*(1.0*cos(th2(t) - 1.5708)*(2.6536e-6*cos(th1(t)) + 1.0*sin(th1(t))) - 1.3268e-6*sin(th2(t) - 1.5708)*cos(th1(t)))) + 0.38*sin(th3(t))*(1.0*cos(th2(t) - 1.5708)*(2.6536e-6*cos(th1(t)) + 1.0*sin(th1(t))) - 1.3268e-6*sin(th2(t) - 1.5708)*cos(th1(t))) + 0.19*cos(th4(t))*(cos(th3(t) - 1.5708)*(sin(th2(t) - 1.5708)*(2.6536e-6*cos(th1(t)) + 1.0*sin(th1(t))) + 1.3268e-6*cos(th2(t) - 1.5708)*cos(th1(t))) + 1.0*sin(th3(t) - 1.5708)*(1.0*cos(th2(t) - 1.5708)*(2.6536e-6*cos(th1(t)) + 1.0*sin(th1(t))) - 1.3268e-6*sin(th2(t) - 1.5708)*cos(th1(t)))))*(5.0418e-7*sin(th1(t))*sin(th2(t)) + 0.38*cos(th2(t))*(1.0*cos(th1(t)) - 2.6536e-6*sin(th1(t))) + 0.38*cos(th3(t))*(cos(th2(t) - 1.5708)*(1.0*cos(th1(t)) - 2.6536e-6*sin(th1(t))) + 1.3268e-6*sin(th2(t) - 1.5708)*sin(th1(t))) + 0.19*cos(th4(t))*(cos(th3(t) - 1.5708)*(cos(th2(t) - 1.5708)*(1.0*cos(th1(t)) - 2.6536e-6*sin(th1(t))) + 1.3268e-6*sin(th2(t) - 1.5708)*sin(th1(t))) - sin(th3(t) - 1.5708)*(1.0*sin(th2(t) - 1.5708)*(1.0*cos(th1(t)) - 2.6536e-6*sin(th1(t))) - 1.3268e-6*cos(th2(t) - 1.5708)*sin(th1(t)))) - 0.38*sin(th3(t))*(1.0*sin(th2(t) - 1.5708)*(1.0*cos(th1(t)) - 2.6536e-6*sin(th1(t))) - 1.3268e-6*cos(th2(t) - 1.5708)*sin(th1(t))) - 0.19*sin(th4(t))*(1.0*sin(th3(t) - 1.5708)*(cos(th2(t) - 1.5708)*(1.0*cos(th1(t)) - 2.6536e-6*sin(th1(t))) + 1.3268e-6*sin(th2(t) - 1.5708)*sin(th1(t))) + cos(th3(t) - 1.5708)*(1.0*sin(th2(t) - 1.5708)*(1.0*cos(th1(t)) - 2.6536e-6*sin(th1(t))) - 1.3268e-6*cos(th2(t) - 1.5708)*sin(th1(t))))) - 0.49277*(0.19*cos(th3(t))*(sin(th2(t) - 1.5708)*(2.6536e-6*cos(th1(t)) + 1.0*sin(th1(t))) + 1.3268e-6*cos(th2(t) - 1.5708)*cos(th1(t))) + 0.19*sin(th3(t))*(1.0*cos(th2(t) - 1.5708)*(2.6536e-6*cos(th1(t)) + 1.0*sin(th1(t))) - 1.3268e-6*sin(th2(t) - 1.5708)*cos(th1(t))))*(5.0418e-7*sin(th1(t))*sin(th2(t)) + 0.38*cos(th2(t))*(1.0*cos(th1(t)) - 2.6536e-6*sin(th1(t))) + 0.19*cos(th3(t))*(cos(th2(t) - 1.5708)*(1.0*cos(th1(t)) - 2.6536e-6*sin(th1(t))) + 1.3268e-6*sin(th2(t) - 1.5708)*sin(th1(t))) - 0.19*sin(th3(t))*(1.0*sin(th2(t) - 1.5708)*(1.0*cos(th1(t)) - 2.6536e-6*sin(th1(t))) - 1.3268e-6*cos(th2(t) - 1.5708)*sin(th1(t)))) - 0.13038*(0.38*cos(th4(t))*(cos(th3(t) - 1.5708)*(sin(th2(t) - 1.5708)*(1.0*cos(th1(t)) - 2.6536e-6*sin(th1(t))) - 1.3268e-6*cos(th2(t) - 1.5708)*sin(th1(t))) + sin(th3(t) - 1.5708)*(cos(th2(t) - 1.5708)*(1.0*cos(th1(t)) - 2.6536e-6*sin(th1(t))) + 1.3268e-6*sin(th2(t) - 1.5708)*sin(th1(t)))) + 0.38*cos(th3(t))*(sin(th2(t) - 1.5708)*(1.0*cos(th1(t)) - 2.6536e-6*sin(th1(t))) - 1.3268e-6*cos(th2(t) - 1.5708)*sin(th1(t))) + 0.38*sin(th3(t))*(cos(th2(t) - 1.5708)*(1.0*cos(th1(t)) - 2.6536e-6*sin(th1(t))) + 1.3268e-6*sin(th2(t) - 1.5708)*sin(th1(t))) - 0.02*sin(th5(t))*(sin(th4(t) - 3.1416)*(cos(th3(t) - 1.5708)*(sin(th2(t) - 1.5708)*(1.0*cos(th1(t)) - 2.6536e-6*sin(th1(t))) - 1.3268e-6*cos(th2(t) - 1.5708)*sin(th1(t))) + sin(th3(t) - 1.5708)*(cos(th2(t) - 1.5708)*(1.0*cos(th1(t)) - 2.6536e-6*sin(th1(t))) + 1.3268e-6*sin(th2(t) - 1.5708)*sin(th1(t)))) + cos(th4(t) - 3.1416)*(cos(th3(t) - 1.5708)*(cos(th2(t) - 1.5708)*(1.0*cos(th1(t)) - 2.6536e-6*sin(th1(t))) + 1.3268e-6*sin(th2(t) - 1.5708)*sin(th1(t))) - 1.0*sin(th3(t) - 1.5708)*(sin(th2(t) - 1.5708)*(1.0*cos(th1(t)) - 2.6536e-6*sin(th1(t))) - 1.3268e-6*cos(th2(t) - 1.5708)*sin(th1(t))))) + 0.38*sin(th4(t))*(cos(th3(t) - 1.5708)*(cos(th2(t) - 1.5708)*(1.0*cos(th1(t)) - 2.6536e-6*sin(th1(t))) + 1.3268e-6*sin(th2(t) - 1.5708)*sin(th1(t))) - 1.0*sin(th3(t) - 1.5708)*(sin(th2(t) - 1.5708)*(1.0*cos(th1(t)) - 2.6536e-6*sin(th1(t))) - 1.3268e-6*cos(th2(t) - 1.5708)*sin(th1(t)))) - 0.02*cos(th5(t))*(cos(th4(t) - 3.1416)*(cos(th3(t) - 1.5708)*(sin(th2(t) - 1.5708)*(1.0*cos(th1(t)) - 2.6536e-6*sin(th1(t))) - 1.3268e-6*cos(th2(t) - 1.5708)*sin(th1(t))) + sin(th3(t) - 1.5708)*(cos(th2(t) - 1.5708)*(1.0*cos(th1(t)) - 2.6536e-6*sin(th1(t))) + 1.3268e-6*sin(th2(t) - 1.5708)*sin(th1(t)))) - 1.0*sin(th4(t) - 3.1416)*(cos(th3(t) - 1.5708)*(cos(th2(t) - 1.5708)*(1.0*cos(th1(t)) - 2.6536e-6*sin(th1(t))) + 1.3268e-6*sin(th2(t) - 1.5708)*sin(th1(t))) - 1.0*sin(th3(t) - 1.5708)*(sin(th2(t) - 1.5708)*(1.0*cos(th1(t)) - 2.6536e-6*sin(th1(t))) - 1.3268e-6*cos(th2(t) - 1.5708)*sin(th1(t))))))*(5.0418e-7*cos(th1(t))*sin(th2(t)) + 0.02*cos(th5(t))*(cos(th4(t) - 3.1416)*(cos(th3(t) - 1.5708)*(cos(th2(t) - 1.5708)*(2.6536e-6*cos(th1(t)) + 1.0*sin(th1(t))) - 1.3268e-6*sin(th2(t) - 1.5708)*cos(th1(t))) - 1.0*sin(th3(t) - 1.5708)*(sin(th2(t) - 1.5708)*(2.6536e-6*cos(th1(t)) + 1.0*sin(th1(t))) + 1.3268e-6*cos(th2(t) - 1.5708)*cos(th1(t)))) + sin(th4(t) - 3.1416)*(cos(th3(t) - 1.5708)*(sin(th2(t) - 1.5708)*(2.6536e-6*cos(th1(t)) + 1.0*sin(th1(t))) + 1.3268e-6*cos(th2(t) - 1.5708)*cos(th1(t))) + sin(th3(t) - 1.5708)*(cos(th2(t) - 1.5708)*(2.6536e-6*cos(th1(t)) + 1.0*sin(th1(t))) - 1.3268e-6*sin(th2(t) - 1.5708)*cos(th1(t))))) + 0.38*sin(th4(t))*(cos(th3(t) - 1.5708)*(sin(th2(t) - 1.5708)*(2.6536e-6*cos(th1(t)) + 1.0*sin(th1(t))) + 1.3268e-6*cos(th2(t) - 1.5708)*cos(th1(t))) + sin(th3(t) - 1.5708)*(cos(th2(t) - 1.5708)*(2.6536e-6*cos(th1(t)) + 1.0*sin(th1(t))) - 1.3268e-6*sin(th2(t) - 1.5708)*cos(th1(t)))) - 0.38*cos(th3(t))*(cos(th2(t) - 1.5708)*(2.6536e-6*cos(th1(t)) + 1.0*sin(th1(t))) - 1.3268e-6*sin(th2(t) - 1.5708)*cos(th1(t))) - 0.38*cos(th2(t))*(2.6536e-6*cos(th1(t)) + 1.0*sin(th1(t))) + 0.38*sin(th3(t))*(sin(th2(t) - 1.5708)*(2.6536e-6*cos(th1(t)) + 1.0*sin(th1(t))) + 1.3268e-6*cos(th2(t) - 1.5708)*cos(th1(t))) - 0.38*cos(th4(t))*(cos(th3(t) - 1.5708)*(cos(th2(t) - 1.5708)*(2.6536e-6*cos(th1(t)) + 1.0*sin(th1(t))) - 1.3268e-6*sin(th2(t) - 1.5708)*cos(th1(t))) - 1.0*sin(th3(t) - 1.5708)*(sin(th2(t) - 1.5708)*(2.6536e-6*cos(th1(t)) + 1.0*sin(th1(t))) + 1.3268e-6*cos(th2(t) - 1.5708)*cos(th1(t)))) + 0.02*sin(th5(t))*(1.0*sin(th4(t) - 3.1416)*(cos(th3(t) - 1.5708)*(cos(th2(t) - 1.5708)*(2.6536e-6*cos(th1(t)) + 1.0*sin(th1(t))) - 1.3268e-6*sin(th2(t) - 1.5708)*cos(th1(t))) - 1.0*sin(th3(t) - 1.5708)*(sin(th2(t) - 1.5708)*(2.6536e-6*cos(th1(t)) + 1.0*sin(th1(t))) + 1.3268e-6*cos(th2(t) - 1.5708)*cos(th1(t)))) - cos(th4(t) - 3.1416)*(cos(th3(t) - 1.5708)*(sin(th2(t) - 1.5708)*(2.6536e-6*cos(th1(t)) + 1.0*sin(th1(t))) + 1.3268e-6*cos(th2(t) - 1.5708)*cos(th1(t))) + sin(th3(t) - 1.5708)*(cos(th2(t) - 1.5708)*(2.6536e-6*cos(th1(t)) + 1.0*sin(th1(t))) - 1.3268e-6*sin(th2(t) - 1.5708)*cos(th1(t)))))) - 1.3806*(0.19*cos(th4(t))*(cos(th3(t) - 1.5708)*(sin(th2(t) - 1.5708)*(1.0*cos(th1(t)) - 2.6536e-6*sin(th1(t))) - 1.3268e-6*cos(th2(t) - 1.5708)*sin(th1(t))) + sin(th3(t) - 1.5708)*(cos(th2(t) - 1.5708)*(1.0*cos(th1(t)) - 2.6536e-6*sin(th1(t))) + 1.3268e-6*sin(th2(t) - 1.5708)*sin(th1(t)))) + 0.38*cos(th3(t))*(sin(th2(t) - 1.5708)*(1.0*cos(th1(t)) - 2.6536e-6*sin(th1(t))) - 1.3268e-6*cos(th2(t) - 1.5708)*sin(th1(t))) + 0.38*sin(th3(t))*(cos(th2(t) - 1.5708)*(1.0*cos(th1(t)) - 2.6536e-6*sin(th1(t))) + 1.3268e-6*sin(th2(t) - 1.5708)*sin(th1(t))) + 0.19*sin(th4(t))*(cos(th3(t) - 1.5708)*(cos(th2(t) - 1.5708)*(1.0*cos(th1(t)) - 2.6536e-6*sin(th1(t))) + 1.3268e-6*sin(th2(t) - 1.5708)*sin(th1(t))) - 1.0*sin(th3(t) - 1.5708)*(sin(th2(t) - 1.5708)*(1.0*cos(th1(t)) - 2.6536e-6*sin(th1(t))) - 1.3268e-6*cos(th2(t) - 1.5708)*sin(th1(t)))))*(5.0418e-7*cos(th1(t))*sin(th2(t)) + 0.19*sin(th4(t))*(cos(th3(t) - 1.5708)*(sin(th2(t) - 1.5708)*(2.6536e-6*cos(th1(t)) + 1.0*sin(th1(t))) + 1.3268e-6*cos(th2(t) - 1.5708)*cos(th1(t))) + sin(th3(t) - 1.5708)*(cos(th2(t) - 1.5708)*(2.6536e-6*cos(th1(t)) + 1.0*sin(th1(t))) - 1.3268e-6*sin(th2(t) - 1.5708)*cos(th1(t)))) - 0.38*cos(th3(t))*(cos(th2(t) - 1.5708)*(2.6536e-6*cos(th1(t)) + 1.0*sin(th1(t))) - 1.3268e-6*sin(th2(t) - 1.5708)*cos(th1(t))) - 0.38*cos(th2(t))*(2.6536e-6*cos(th1(t)) + 1.0*sin(th1(t))) + 0.38*sin(th3(t))*(sin(th2(t) - 1.5708)*(2.6536e-6*cos(th1(t)) + 1.0*sin(th1(t))) + 1.3268e-6*cos(th2(t) - 1.5708)*cos(th1(t))) - 0.19*cos(th4(t))*(cos(th3(t) - 1.5708)*(cos(th2(t) - 1.5708)*(2.6536e-6*cos(th1(t)) + 1.0*sin(th1(t))) - 1.3268e-6*sin(th2(t) - 1.5708)*cos(th1(t))) - 1.0*sin(th3(t) - 1.5708)*(sin(th2(t) - 1.5708)*(2.6536e-6*cos(th1(t)) + 1.0*sin(th1(t))) + 1.3268e-6*cos(th2(t) - 1.5708)*cos(th1(t))))) - 0.49277*(0.19*cos(th3(t))*(sin(th2(t) - 1.5708)*(1.0*cos(th1(t)) - 2.6536e-6*sin(th1(t))) - 1.3268e-6*cos(th2(t) - 1.5708)*sin(th1(t))) + 0.19*sin(th3(t))*(cos(th2(t) - 1.5708)*(1.0*cos(th1(t)) - 2.6536e-6*sin(th1(t))) + 1.3268e-6*sin(th2(t) - 1.5708)*sin(th1(t))))*(5.0418e-7*cos(th1(t))*sin(th2(t)) - 0.19*cos(th3(t))*(cos(th2(t) - 1.5708)*(2.6536e-6*cos(th1(t)) + 1.0*sin(th1(t))) - 1.3268e-6*sin(th2(t) - 1.5708)*cos(th1(t))) - 0.38*cos(th2(t))*(2.6536e-6*cos(th1(t)) + 1.0*sin(th1(t))) + 0.19*sin(th3(t))*(sin(th2(t) - 1.5708)*(2.6536e-6*cos(th1(t)) + 1.0*sin(th1(t))) + 1.3268e-6*cos(th2(t) - 1.5708)*cos(th1(t)))) - 0.13038*(0.38*cos(th3(t))*(sin(th2(t) - 1.5708)*(2.6536e-6*cos(th1(t)) + 1.0*sin(th1(t))) + 1.3268e-6*cos(th2(t) - 1.5708)*cos(th1(t))) - 0.38*sin(th4(t))*(sin(th3(t) - 1.5708)*(sin(th2(t) - 1.5708)*(2.6536e-6*cos(th1(t)) + 1.0*sin(th1(t))) + 1.3268e-6*cos(th2(t) - 1.5708)*cos(th1(t))) - cos(th3(t) - 1.5708)*(1.0*cos(th2(t) - 1.5708)*(2.6536e-6*cos(th1(t)) + 1.0*sin(th1(t))) - 1.3268e-6*sin(th2(t) - 1.5708)*cos(th1(t)))) + 0.38*sin(th3(t))*(1.0*cos(th2(t) - 1.5708)*(2.6536e-6*cos(th1(t)) + 1.0*sin(th1(t))) - 1.3268e-6*sin(th2(t) - 1.5708)*cos(th1(t))) - 0.02*cos(th5(t))*(sin(th4(t) - 3.1416)*(sin(th3(t) - 1.5708)*(sin(th2(t) - 1.5708)*(2.6536e-6*cos(th1(t)) + 1.0*sin(th1(t))) + 1.3268e-6*cos(th2(t) - 1.5708)*cos(th1(t))) - cos(th3(t) - 1.5708)*(1.0*cos(th2(t) - 1.5708)*(2.6536e-6*cos(th1(t)) + 1.0*sin(th1(t))) - 1.3268e-6*sin(th2(t) - 1.5708)*cos(th1(t)))) + cos(th4(t) - 3.1416)*(cos(th3(t) - 1.5708)*(sin(th2(t) - 1.5708)*(2.6536e-6*cos(th1(t)) + 1.0*sin(th1(t))) + 1.3268e-6*cos(th2(t) - 1.5708)*cos(th1(t))) + 1.0*sin(th3(t) - 1.5708)*(1.0*cos(th2(t) - 1.5708)*(2.6536e-6*cos(th1(t)) + 1.0*sin(th1(t))) - 1.3268e-6*sin(th2(t) - 1.5708)*cos(th1(t))))) + 0.38*cos(th4(t))*(cos(th3(t) - 1.5708)*(sin(th2(t) - 1.5708)*(2.6536e-6*cos(th1(t)) + 1.0*sin(th1(t))) + 1.3268e-6*cos(th2(t) - 1.5708)*cos(th1(t))) + 1.0*sin(th3(t) - 1.5708)*(1.0*cos(th2(t) - 1.5708)*(2.6536e-6*cos(th1(t)) + 1.0*sin(th1(t))) - 1.3268e-6*sin(th2(t) - 1.5708)*cos(th1(t)))) + 0.02*sin(th5(t))*(cos(th4(t) - 3.1416)*(sin(th3(t) - 1.5708)*(sin(th2(t) - 1.5708)*(2.6536e-6*cos(th1(t)) + 1.0*sin(th1(t))) + 1.3268e-6*cos(th2(t) - 1.5708)*cos(th1(t))) - cos(th3(t) - 1.5708)*(1.0*cos(th2(t) - 1.5708)*(2.6536e-6*cos(th1(t)) + 1.0*sin(th1(t))) - 1.3268e-6*sin(th2(t) - 1.5708)*cos(th1(t)))) - 1.0*sin(th4(t) - 3.1416)*(cos(th3(t) - 1.5708)*(sin(th2(t) - 1.5708)*(2.6536e-6*cos(th1(t)) + 1.0*sin(th1(t))) + 1.3268e-6*cos(th2(t) - 1.5708)*cos(th1(t))) + 1.0*sin(th3(t) - 1.5708)*(1.0*cos(th2(t) - 1.5708)*(2.6536e-6*cos(th1(t)) + 1.0*sin(th1(t))) - 1.3268e-6*sin(th2(t) - 1.5708)*cos(th1(t))))))*(5.0418e-7*sin(th1(t))*sin(th2(t)) - 0.02*cos(th5(t))*(cos(th4(t) - 3.1416)*(cos(th3(t) - 1.5708)*(cos(th2(t) - 1.5708)*(1.0*cos(th1(t)) - 2.6536e-6*sin(th1(t))) + 1.3268e-6*sin(th2(t) - 1.5708)*sin(th1(t))) - sin(th3(t) - 1.5708)*(1.0*sin(th2(t) - 1.5708)*(1.0*cos(th1(t)) - 2.6536e-6*sin(th1(t))) - 1.3268e-6*cos(th2(t) - 1.5708)*sin(th1(t)))) + 1.0*sin(th4(t) - 3.1416)*(1.0*sin(th3(t) - 1.5708)*(cos(th2(t) - 1.5708)*(1.0*cos(th1(t)) - 2.6536e-6*sin(th1(t))) + 1.3268e-6*sin(th2(t) - 1.5708)*sin(th1(t))) + cos(th3(t) - 1.5708)*(1.0*sin(th2(t) - 1.5708)*(1.0*cos(th1(t)) - 2.6536e-6*sin(th1(t))) - 1.3268e-6*cos(th2(t) - 1.5708)*sin(th1(t))))) + 0.38*cos(th2(t))*(1.0*cos(th1(t)) - 2.6536e-6*sin(th1(t))) + 0.38*cos(th3(t))*(cos(th2(t) - 1.5708)*(1.0*cos(th1(t)) - 2.6536e-6*sin(th1(t))) + 1.3268e-6*sin(th2(t) - 1.5708)*sin(th1(t))) + 0.38*cos(th4(t))*(cos(th3(t) - 1.5708)*(cos(th2(t) - 1.5708)*(1.0*cos(th1(t)) - 2.6536e-6*sin(th1(t))) + 1.3268e-6*sin(th2(t) - 1.5708)*sin(th1(t))) - sin(th3(t) - 1.5708)*(1.0*sin(th2(t) - 1.5708)*(1.0*cos(th1(t)) - 2.6536e-6*sin(th1(t))) - 1.3268e-6*cos(th2(t) - 1.5708)*sin(th1(t)))) - 0.38*sin(th3(t))*(1.0*sin(th2(t) - 1.5708)*(1.0*cos(th1(t)) - 2.6536e-6*sin(th1(t))) - 1.3268e-6*cos(th2(t) - 1.5708)*sin(th1(t))) - 0.38*sin(th4(t))*(1.0*sin(th3(t) - 1.5708)*(cos(th2(t) - 1.5708)*(1.0*cos(th1(t)) - 2.6536e-6*sin(th1(t))) + 1.3268e-6*sin(th2(t) - 1.5708)*sin(th1(t))) + cos(th3(t) - 1.5708)*(1.0*sin(th2(t) - 1.5708)*(1.0*cos(th1(t)) - 2.6536e-6*sin(th1(t))) - 1.3268e-6*cos(th2(t) - 1.5708)*sin(th1(t)))) - 0.02*sin(th5(t))*(sin(th4(t) - 3.1416)*(cos(th3(t) - 1.5708)*(cos(th2(t) - 1.5708)*(1.0*cos(th1(t)) - 2.6536e-6*sin(th1(t))) + 1.3268e-6*sin(th2(t) - 1.5708)*sin(th1(t))) - sin(th3(t) - 1.5708)*(1.0*sin(th2(t) - 1.5708)*(1.0*cos(th1(t)) - 2.6536e-6*sin(th1(t))) - 1.3268e-6*cos(th2(t) - 1.5708)*sin(th1(t)))) - cos(th4(t) - 3.1416)*(1.0*sin(th3(t) - 1.5708)*(cos(th2(t) - 1.5708)*(1.0*cos(th1(t)) - 2.6536e-6*sin(th1(t))) + 1.3268e-6*sin(th2(t) - 1.5708)*sin(th1(t))) + cos(th3(t) - 1.5708)*(1.0*sin(th2(t) - 1.5708)*(1.0*cos(th1(t)) - 2.6536e-6*sin(th1(t))) - 1.3268e-6*cos(th2(t) - 1.5708)*sin(th1(t))))));
M14 = 0.13038*(0.38*sin(th4(t))*(sin(th3(t) - 1.5708)*(sin(th2(t) - 1.5708)*(2.6536e-6*cos(th1(t)) + 1.0*sin(th1(t))) + 1.3268e-6*cos(th2(t) - 1.5708)*cos(th1(t))) - cos(th3(t) - 1.5708)*(1.0*cos(th2(t) - 1.5708)*(2.6536e-6*cos(th1(t)) + 1.0*sin(th1(t))) - 1.3268e-6*sin(th2(t) - 1.5708)*cos(th1(t)))) - 0.02*cos(th5(t))*(sin(th4(t) - 3.1416)*(sin(th3(t) - 1.5708)*(sin(th2(t) - 1.5708)*(2.6536e-6*cos(th1(t)) + 1.0*sin(th1(t))) + 1.3268e-6*cos(th2(t) - 1.5708)*cos(th1(t))) - cos(th3(t) - 1.5708)*(1.0*cos(th2(t) - 1.5708)*(2.6536e-6*cos(th1(t)) + 1.0*sin(th1(t))) - 1.3268e-6*sin(th2(t) - 1.5708)*cos(th1(t)))) + cos(th4(t) - 3.1416)*(cos(th3(t) - 1.5708)*(sin(th2(t) - 1.5708)*(2.6536e-6*cos(th1(t)) + 1.0*sin(th1(t))) + 1.3268e-6*cos(th2(t) - 1.5708)*cos(th1(t))) + 1.0*sin(th3(t) - 1.5708)*(1.0*cos(th2(t) - 1.5708)*(2.6536e-6*cos(th1(t)) + 1.0*sin(th1(t))) - 1.3268e-6*sin(th2(t) - 1.5708)*cos(th1(t))))) - 0.38*cos(th4(t))*(cos(th3(t) - 1.5708)*(sin(th2(t) - 1.5708)*(2.6536e-6*cos(th1(t)) + 1.0*sin(th1(t))) + 1.3268e-6*cos(th2(t) - 1.5708)*cos(th1(t))) + 1.0*sin(th3(t) - 1.5708)*(1.0*cos(th2(t) - 1.5708)*(2.6536e-6*cos(th1(t)) + 1.0*sin(th1(t))) - 1.3268e-6*sin(th2(t) - 1.5708)*cos(th1(t)))) + 0.02*sin(th5(t))*(cos(th4(t) - 3.1416)*(sin(th3(t) - 1.5708)*(sin(th2(t) - 1.5708)*(2.6536e-6*cos(th1(t)) + 1.0*sin(th1(t))) + 1.3268e-6*cos(th2(t) - 1.5708)*cos(th1(t))) - cos(th3(t) - 1.5708)*(1.0*cos(th2(t) - 1.5708)*(2.6536e-6*cos(th1(t)) + 1.0*sin(th1(t))) - 1.3268e-6*sin(th2(t) - 1.5708)*cos(th1(t)))) - 1.0*sin(th4(t) - 3.1416)*(cos(th3(t) - 1.5708)*(sin(th2(t) - 1.5708)*(2.6536e-6*cos(th1(t)) + 1.0*sin(th1(t))) + 1.3268e-6*cos(th2(t) - 1.5708)*cos(th1(t))) + 1.0*sin(th3(t) - 1.5708)*(1.0*cos(th2(t) - 1.5708)*(2.6536e-6*cos(th1(t)) + 1.0*sin(th1(t))) - 1.3268e-6*sin(th2(t) - 1.5708)*cos(th1(t))))))*(5.0418e-7*sin(th1(t))*sin(th2(t)) - 0.02*cos(th5(t))*(cos(th4(t) - 3.1416)*(cos(th3(t) - 1.5708)*(cos(th2(t) - 1.5708)*(1.0*cos(th1(t)) - 2.6536e-6*sin(th1(t))) + 1.3268e-6*sin(th2(t) - 1.5708)*sin(th1(t))) - sin(th3(t) - 1.5708)*(1.0*sin(th2(t) - 1.5708)*(1.0*cos(th1(t)) - 2.6536e-6*sin(th1(t))) - 1.3268e-6*cos(th2(t) - 1.5708)*sin(th1(t)))) + 1.0*sin(th4(t) - 3.1416)*(1.0*sin(th3(t) - 1.5708)*(cos(th2(t) - 1.5708)*(1.0*cos(th1(t)) - 2.6536e-6*sin(th1(t))) + 1.3268e-6*sin(th2(t) - 1.5708)*sin(th1(t))) + cos(th3(t) - 1.5708)*(1.0*sin(th2(t) - 1.5708)*(1.0*cos(th1(t)) - 2.6536e-6*sin(th1(t))) - 1.3268e-6*cos(th2(t) - 1.5708)*sin(th1(t))))) + 0.38*cos(th2(t))*(1.0*cos(th1(t)) - 2.6536e-6*sin(th1(t))) + 0.38*cos(th3(t))*(cos(th2(t) - 1.5708)*(1.0*cos(th1(t)) - 2.6536e-6*sin(th1(t))) + 1.3268e-6*sin(th2(t) - 1.5708)*sin(th1(t))) + 0.38*cos(th4(t))*(cos(th3(t) - 1.5708)*(cos(th2(t) - 1.5708)*(1.0*cos(th1(t)) - 2.6536e-6*sin(th1(t))) + 1.3268e-6*sin(th2(t) - 1.5708)*sin(th1(t))) - sin(th3(t) - 1.5708)*(1.0*sin(th2(t) - 1.5708)*(1.0*cos(th1(t)) - 2.6536e-6*sin(th1(t))) - 1.3268e-6*cos(th2(t) - 1.5708)*sin(th1(t)))) - 0.38*sin(th3(t))*(1.0*sin(th2(t) - 1.5708)*(1.0*cos(th1(t)) - 2.6536e-6*sin(th1(t))) - 1.3268e-6*cos(th2(t) - 1.5708)*sin(th1(t))) - 0.38*sin(th4(t))*(1.0*sin(th3(t) - 1.5708)*(cos(th2(t) - 1.5708)*(1.0*cos(th1(t)) - 2.6536e-6*sin(th1(t))) + 1.3268e-6*sin(th2(t) - 1.5708)*sin(th1(t))) + cos(th3(t) - 1.5708)*(1.0*sin(th2(t) - 1.5708)*(1.0*cos(th1(t)) - 2.6536e-6*sin(th1(t))) - 1.3268e-6*cos(th2(t) - 1.5708)*sin(th1(t)))) - 0.02*sin(th5(t))*(sin(th4(t) - 3.1416)*(cos(th3(t) - 1.5708)*(cos(th2(t) - 1.5708)*(1.0*cos(th1(t)) - 2.6536e-6*sin(th1(t))) + 1.3268e-6*sin(th2(t) - 1.5708)*sin(th1(t))) - sin(th3(t) - 1.5708)*(1.0*sin(th2(t) - 1.5708)*(1.0*cos(th1(t)) - 2.6536e-6*sin(th1(t))) - 1.3268e-6*cos(th2(t) - 1.5708)*sin(th1(t)))) - cos(th4(t) - 3.1416)*(1.0*sin(th3(t) - 1.5708)*(cos(th2(t) - 1.5708)*(1.0*cos(th1(t)) - 2.6536e-6*sin(th1(t))) + 1.3268e-6*sin(th2(t) - 1.5708)*sin(th1(t))) + cos(th3(t) - 1.5708)*(1.0*sin(th2(t) - 1.5708)*(1.0*cos(th1(t)) - 2.6536e-6*sin(th1(t))) - 1.3268e-6*cos(th2(t) - 1.5708)*sin(th1(t)))))) - 1.3806*(0.19*cos(th4(t))*(cos(th3(t) - 1.5708)*(sin(th2(t) - 1.5708)*(1.0*cos(th1(t)) - 2.6536e-6*sin(th1(t))) - 1.3268e-6*cos(th2(t) - 1.5708)*sin(th1(t))) + sin(th3(t) - 1.5708)*(cos(th2(t) - 1.5708)*(1.0*cos(th1(t)) - 2.6536e-6*sin(th1(t))) + 1.3268e-6*sin(th2(t) - 1.5708)*sin(th1(t)))) + 0.19*sin(th4(t))*(cos(th3(t) - 1.5708)*(cos(th2(t) - 1.5708)*(1.0*cos(th1(t)) - 2.6536e-6*sin(th1(t))) + 1.3268e-6*sin(th2(t) - 1.5708)*sin(th1(t))) - 1.0*sin(th3(t) - 1.5708)*(sin(th2(t) - 1.5708)*(1.0*cos(th1(t)) - 2.6536e-6*sin(th1(t))) - 1.3268e-6*cos(th2(t) - 1.5708)*sin(th1(t)))))*(5.0418e-7*cos(th1(t))*sin(th2(t)) + 0.19*sin(th4(t))*(cos(th3(t) - 1.5708)*(sin(th2(t) - 1.5708)*(2.6536e-6*cos(th1(t)) + 1.0*sin(th1(t))) + 1.3268e-6*cos(th2(t) - 1.5708)*cos(th1(t))) + sin(th3(t) - 1.5708)*(cos(th2(t) - 1.5708)*(2.6536e-6*cos(th1(t)) + 1.0*sin(th1(t))) - 1.3268e-6*sin(th2(t) - 1.5708)*cos(th1(t)))) - 0.38*cos(th3(t))*(cos(th2(t) - 1.5708)*(2.6536e-6*cos(th1(t)) + 1.0*sin(th1(t))) - 1.3268e-6*sin(th2(t) - 1.5708)*cos(th1(t))) - 0.38*cos(th2(t))*(2.6536e-6*cos(th1(t)) + 1.0*sin(th1(t))) + 0.38*sin(th3(t))*(sin(th2(t) - 1.5708)*(2.6536e-6*cos(th1(t)) + 1.0*sin(th1(t))) + 1.3268e-6*cos(th2(t) - 1.5708)*cos(th1(t))) - 0.19*cos(th4(t))*(cos(th3(t) - 1.5708)*(cos(th2(t) - 1.5708)*(2.6536e-6*cos(th1(t)) + 1.0*sin(th1(t))) - 1.3268e-6*sin(th2(t) - 1.5708)*cos(th1(t))) - 1.0*sin(th3(t) - 1.5708)*(sin(th2(t) - 1.5708)*(2.6536e-6*cos(th1(t)) + 1.0*sin(th1(t))) + 1.3268e-6*cos(th2(t) - 1.5708)*cos(th1(t))))) - 0.13038*(0.38*cos(th4(t))*(cos(th3(t) - 1.5708)*(sin(th2(t) - 1.5708)*(1.0*cos(th1(t)) - 2.6536e-6*sin(th1(t))) - 1.3268e-6*cos(th2(t) - 1.5708)*sin(th1(t))) + sin(th3(t) - 1.5708)*(cos(th2(t) - 1.5708)*(1.0*cos(th1(t)) - 2.6536e-6*sin(th1(t))) + 1.3268e-6*sin(th2(t) - 1.5708)*sin(th1(t)))) + 0.02*sin(th5(t))*(sin(th4(t) - 3.1416)*(cos(th3(t) - 1.5708)*(sin(th2(t) - 1.5708)*(1.0*cos(th1(t)) - 2.6536e-6*sin(th1(t))) - 1.3268e-6*cos(th2(t) - 1.5708)*sin(th1(t))) + sin(th3(t) - 1.5708)*(cos(th2(t) - 1.5708)*(1.0*cos(th1(t)) - 2.6536e-6*sin(th1(t))) + 1.3268e-6*sin(th2(t) - 1.5708)*sin(th1(t)))) + cos(th4(t) - 3.1416)*(cos(th3(t) - 1.5708)*(cos(th2(t) - 1.5708)*(1.0*cos(th1(t)) - 2.6536e-6*sin(th1(t))) + 1.3268e-6*sin(th2(t) - 1.5708)*sin(th1(t))) - 1.0*sin(th3(t) - 1.5708)*(sin(th2(t) - 1.5708)*(1.0*cos(th1(t)) - 2.6536e-6*sin(th1(t))) - 1.3268e-6*cos(th2(t) - 1.5708)*sin(th1(t))))) + 0.38*sin(th4(t))*(cos(th3(t) - 1.5708)*(cos(th2(t) - 1.5708)*(1.0*cos(th1(t)) - 2.6536e-6*sin(th1(t))) + 1.3268e-6*sin(th2(t) - 1.5708)*sin(th1(t))) - 1.0*sin(th3(t) - 1.5708)*(sin(th2(t) - 1.5708)*(1.0*cos(th1(t)) - 2.6536e-6*sin(th1(t))) - 1.3268e-6*cos(th2(t) - 1.5708)*sin(th1(t)))) + 0.02*cos(th5(t))*(cos(th4(t) - 3.1416)*(cos(th3(t) - 1.5708)*(sin(th2(t) - 1.5708)*(1.0*cos(th1(t)) - 2.6536e-6*sin(th1(t))) - 1.3268e-6*cos(th2(t) - 1.5708)*sin(th1(t))) + sin(th3(t) - 1.5708)*(cos(th2(t) - 1.5708)*(1.0*cos(th1(t)) - 2.6536e-6*sin(th1(t))) + 1.3268e-6*sin(th2(t) - 1.5708)*sin(th1(t)))) - 1.0*sin(th4(t) - 3.1416)*(cos(th3(t) - 1.5708)*(cos(th2(t) - 1.5708)*(1.0*cos(th1(t)) - 2.6536e-6*sin(th1(t))) + 1.3268e-6*sin(th2(t) - 1.5708)*sin(th1(t))) - 1.0*sin(th3(t) - 1.5708)*(sin(th2(t) - 1.5708)*(1.0*cos(th1(t)) - 2.6536e-6*sin(th1(t))) - 1.3268e-6*cos(th2(t) - 1.5708)*sin(th1(t))))))*(5.0418e-7*cos(th1(t))*sin(th2(t)) + 0.02*cos(th5(t))*(cos(th4(t) - 3.1416)*(cos(th3(t) - 1.5708)*(cos(th2(t) - 1.5708)*(2.6536e-6*cos(th1(t)) + 1.0*sin(th1(t))) - 1.3268e-6*sin(th2(t) - 1.5708)*cos(th1(t))) - 1.0*sin(th3(t) - 1.5708)*(sin(th2(t) - 1.5708)*(2.6536e-6*cos(th1(t)) + 1.0*sin(th1(t))) + 1.3268e-6*cos(th2(t) - 1.5708)*cos(th1(t)))) + sin(th4(t) - 3.1416)*(cos(th3(t) - 1.5708)*(sin(th2(t) - 1.5708)*(2.6536e-6*cos(th1(t)) + 1.0*sin(th1(t))) + 1.3268e-6*cos(th2(t) - 1.5708)*cos(th1(t))) + sin(th3(t) - 1.5708)*(cos(th2(t) - 1.5708)*(2.6536e-6*cos(th1(t)) + 1.0*sin(th1(t))) - 1.3268e-6*sin(th2(t) - 1.5708)*cos(th1(t))))) + 0.38*sin(th4(t))*(cos(th3(t) - 1.5708)*(sin(th2(t) - 1.5708)*(2.6536e-6*cos(th1(t)) + 1.0*sin(th1(t))) + 1.3268e-6*cos(th2(t) - 1.5708)*cos(th1(t))) + sin(th3(t) - 1.5708)*(cos(th2(t) - 1.5708)*(2.6536e-6*cos(th1(t)) + 1.0*sin(th1(t))) - 1.3268e-6*sin(th2(t) - 1.5708)*cos(th1(t)))) - 0.38*cos(th3(t))*(cos(th2(t) - 1.5708)*(2.6536e-6*cos(th1(t)) + 1.0*sin(th1(t))) - 1.3268e-6*sin(th2(t) - 1.5708)*cos(th1(t))) - 0.38*cos(th2(t))*(2.6536e-6*cos(th1(t)) + 1.0*sin(th1(t))) + 0.38*sin(th3(t))*(sin(th2(t) - 1.5708)*(2.6536e-6*cos(th1(t)) + 1.0*sin(th1(t))) + 1.3268e-6*cos(th2(t) - 1.5708)*cos(th1(t))) - 0.38*cos(th4(t))*(cos(th3(t) - 1.5708)*(cos(th2(t) - 1.5708)*(2.6536e-6*cos(th1(t)) + 1.0*sin(th1(t))) - 1.3268e-6*sin(th2(t) - 1.5708)*cos(th1(t))) - 1.0*sin(th3(t) - 1.5708)*(sin(th2(t) - 1.5708)*(2.6536e-6*cos(th1(t)) + 1.0*sin(th1(t))) + 1.3268e-6*cos(th2(t) - 1.5708)*cos(th1(t)))) + 0.02*sin(th5(t))*(1.0*sin(th4(t) - 3.1416)*(cos(th3(t) - 1.5708)*(cos(th2(t) - 1.5708)*(2.6536e-6*cos(th1(t)) + 1.0*sin(th1(t))) - 1.3268e-6*sin(th2(t) - 1.5708)*cos(th1(t))) - 1.0*sin(th3(t) - 1.5708)*(sin(th2(t) - 1.5708)*(2.6536e-6*cos(th1(t)) + 1.0*sin(th1(t))) + 1.3268e-6*cos(th2(t) - 1.5708)*cos(th1(t)))) - cos(th4(t) - 3.1416)*(cos(th3(t) - 1.5708)*(sin(th2(t) - 1.5708)*(2.6536e-6*cos(th1(t)) + 1.0*sin(th1(t))) + 1.3268e-6*cos(th2(t) - 1.5708)*cos(th1(t))) + sin(th3(t) - 1.5708)*(cos(th2(t) - 1.5708)*(2.6536e-6*cos(th1(t)) + 1.0*sin(th1(t))) - 1.3268e-6*sin(th2(t) - 1.5708)*cos(th1(t)))))) + 1.3806*(0.19*sin(th4(t))*(sin(th3(t) - 1.5708)*(sin(th2(t) - 1.5708)*(2.6536e-6*cos(th1(t)) + 1.0*sin(th1(t))) + 1.3268e-6*cos(th2(t) - 1.5708)*cos(th1(t))) - cos(th3(t) - 1.5708)*(1.0*cos(th2(t) - 1.5708)*(2.6536e-6*cos(th1(t)) + 1.0*sin(th1(t))) - 1.3268e-6*sin(th2(t) - 1.5708)*cos(th1(t)))) - 0.19*cos(th4(t))*(cos(th3(t) - 1.5708)*(sin(th2(t) - 1.5708)*(2.6536e-6*cos(th1(t)) + 1.0*sin(th1(t))) + 1.3268e-6*cos(th2(t) - 1.5708)*cos(th1(t))) + 1.0*sin(th3(t) - 1.5708)*(1.0*cos(th2(t) - 1.5708)*(2.6536e-6*cos(th1(t)) + 1.0*sin(th1(t))) - 1.3268e-6*sin(th2(t) - 1.5708)*cos(th1(t)))))*(5.0418e-7*sin(th1(t))*sin(th2(t)) + 0.38*cos(th2(t))*(1.0*cos(th1(t)) - 2.6536e-6*sin(th1(t))) + 0.38*cos(th3(t))*(cos(th2(t) - 1.5708)*(1.0*cos(th1(t)) - 2.6536e-6*sin(th1(t))) + 1.3268e-6*sin(th2(t) - 1.5708)*sin(th1(t))) + 0.19*cos(th4(t))*(cos(th3(t) - 1.5708)*(cos(th2(t) - 1.5708)*(1.0*cos(th1(t)) - 2.6536e-6*sin(th1(t))) + 1.3268e-6*sin(th2(t) - 1.5708)*sin(th1(t))) - sin(th3(t) - 1.5708)*(1.0*sin(th2(t) - 1.5708)*(1.0*cos(th1(t)) - 2.6536e-6*sin(th1(t))) - 1.3268e-6*cos(th2(t) - 1.5708)*sin(th1(t)))) - 0.38*sin(th3(t))*(1.0*sin(th2(t) - 1.5708)*(1.0*cos(th1(t)) - 2.6536e-6*sin(th1(t))) - 1.3268e-6*cos(th2(t) - 1.5708)*sin(th1(t))) - 0.19*sin(th4(t))*(1.0*sin(th3(t) - 1.5708)*(cos(th2(t) - 1.5708)*(1.0*cos(th1(t)) - 2.6536e-6*sin(th1(t))) + 1.3268e-6*sin(th2(t) - 1.5708)*sin(th1(t))) + cos(th3(t) - 1.5708)*(1.0*sin(th2(t) - 1.5708)*(1.0*cos(th1(t)) - 2.6536e-6*sin(th1(t))) - 1.3268e-6*cos(th2(t) - 1.5708)*sin(th1(t))))) + 0.042427;
M15 = 0.13038*(0.02*sin(th5(t))*(sin(th4(t) - 3.1416)*(cos(th3(t) - 1.5708)*(sin(th2(t) - 1.5708)*(1.0*cos(th1(t)) - 2.6536e-6*sin(th1(t))) - 1.3268e-6*cos(th2(t) - 1.5708)*sin(th1(t))) + sin(th3(t) - 1.5708)*(cos(th2(t) - 1.5708)*(1.0*cos(th1(t)) - 2.6536e-6*sin(th1(t))) + 1.3268e-6*sin(th2(t) - 1.5708)*sin(th1(t)))) + cos(th4(t) - 3.1416)*(cos(th3(t) - 1.5708)*(cos(th2(t) - 1.5708)*(1.0*cos(th1(t)) - 2.6536e-6*sin(th1(t))) + 1.3268e-6*sin(th2(t) - 1.5708)*sin(th1(t))) - 1.0*sin(th3(t) - 1.5708)*(sin(th2(t) - 1.5708)*(1.0*cos(th1(t)) - 2.6536e-6*sin(th1(t))) - 1.3268e-6*cos(th2(t) - 1.5708)*sin(th1(t))))) + 0.02*cos(th5(t))*(cos(th4(t) - 3.1416)*(cos(th3(t) - 1.5708)*(sin(th2(t) - 1.5708)*(1.0*cos(th1(t)) - 2.6536e-6*sin(th1(t))) - 1.3268e-6*cos(th2(t) - 1.5708)*sin(th1(t))) + sin(th3(t) - 1.5708)*(cos(th2(t) - 1.5708)*(1.0*cos(th1(t)) - 2.6536e-6*sin(th1(t))) + 1.3268e-6*sin(th2(t) - 1.5708)*sin(th1(t)))) - 1.0*sin(th4(t) - 3.1416)*(cos(th3(t) - 1.5708)*(cos(th2(t) - 1.5708)*(1.0*cos(th1(t)) - 2.6536e-6*sin(th1(t))) + 1.3268e-6*sin(th2(t) - 1.5708)*sin(th1(t))) - 1.0*sin(th3(t) - 1.5708)*(sin(th2(t) - 1.5708)*(1.0*cos(th1(t)) - 2.6536e-6*sin(th1(t))) - 1.3268e-6*cos(th2(t) - 1.5708)*sin(th1(t))))))*(5.0418e-7*cos(th1(t))*sin(th2(t)) + 0.02*cos(th5(t))*(cos(th4(t) - 3.1416)*(cos(th3(t) - 1.5708)*(cos(th2(t) - 1.5708)*(2.6536e-6*cos(th1(t)) + 1.0*sin(th1(t))) - 1.3268e-6*sin(th2(t) - 1.5708)*cos(th1(t))) - 1.0*sin(th3(t) - 1.5708)*(sin(th2(t) - 1.5708)*(2.6536e-6*cos(th1(t)) + 1.0*sin(th1(t))) + 1.3268e-6*cos(th2(t) - 1.5708)*cos(th1(t)))) + sin(th4(t) - 3.1416)*(cos(th3(t) - 1.5708)*(sin(th2(t) - 1.5708)*(2.6536e-6*cos(th1(t)) + 1.0*sin(th1(t))) + 1.3268e-6*cos(th2(t) - 1.5708)*cos(th1(t))) + sin(th3(t) - 1.5708)*(cos(th2(t) - 1.5708)*(2.6536e-6*cos(th1(t)) + 1.0*sin(th1(t))) - 1.3268e-6*sin(th2(t) - 1.5708)*cos(th1(t))))) + 0.38*sin(th4(t))*(cos(th3(t) - 1.5708)*(sin(th2(t) - 1.5708)*(2.6536e-6*cos(th1(t)) + 1.0*sin(th1(t))) + 1.3268e-6*cos(th2(t) - 1.5708)*cos(th1(t))) + sin(th3(t) - 1.5708)*(cos(th2(t) - 1.5708)*(2.6536e-6*cos(th1(t)) + 1.0*sin(th1(t))) - 1.3268e-6*sin(th2(t) - 1.5708)*cos(th1(t)))) - 0.38*cos(th3(t))*(cos(th2(t) - 1.5708)*(2.6536e-6*cos(th1(t)) + 1.0*sin(th1(t))) - 1.3268e-6*sin(th2(t) - 1.5708)*cos(th1(t))) - 0.38*cos(th2(t))*(2.6536e-6*cos(th1(t)) + 1.0*sin(th1(t))) + 0.38*sin(th3(t))*(sin(th2(t) - 1.5708)*(2.6536e-6*cos(th1(t)) + 1.0*sin(th1(t))) + 1.3268e-6*cos(th2(t) - 1.5708)*cos(th1(t))) - 0.38*cos(th4(t))*(cos(th3(t) - 1.5708)*(cos(th2(t) - 1.5708)*(2.6536e-6*cos(th1(t)) + 1.0*sin(th1(t))) - 1.3268e-6*sin(th2(t) - 1.5708)*cos(th1(t))) - 1.0*sin(th3(t) - 1.5708)*(sin(th2(t) - 1.5708)*(2.6536e-6*cos(th1(t)) + 1.0*sin(th1(t))) + 1.3268e-6*cos(th2(t) - 1.5708)*cos(th1(t)))) + 0.02*sin(th5(t))*(1.0*sin(th4(t) - 3.1416)*(cos(th3(t) - 1.5708)*(cos(th2(t) - 1.5708)*(2.6536e-6*cos(th1(t)) + 1.0*sin(th1(t))) - 1.3268e-6*sin(th2(t) - 1.5708)*cos(th1(t))) - 1.0*sin(th3(t) - 1.5708)*(sin(th2(t) - 1.5708)*(2.6536e-6*cos(th1(t)) + 1.0*sin(th1(t))) + 1.3268e-6*cos(th2(t) - 1.5708)*cos(th1(t)))) - cos(th4(t) - 3.1416)*(cos(th3(t) - 1.5708)*(sin(th2(t) - 1.5708)*(2.6536e-6*cos(th1(t)) + 1.0*sin(th1(t))) + 1.3268e-6*cos(th2(t) - 1.5708)*cos(th1(t))) + sin(th3(t) - 1.5708)*(cos(th2(t) - 1.5708)*(2.6536e-6*cos(th1(t)) + 1.0*sin(th1(t))) - 1.3268e-6*sin(th2(t) - 1.5708)*cos(th1(t)))))) + 0.13038*(0.02*cos(th5(t))*(sin(th4(t) - 3.1416)*(sin(th3(t) - 1.5708)*(sin(th2(t) - 1.5708)*(2.6536e-6*cos(th1(t)) + 1.0*sin(th1(t))) + 1.3268e-6*cos(th2(t) - 1.5708)*cos(th1(t))) - cos(th3(t) - 1.5708)*(1.0*cos(th2(t) - 1.5708)*(2.6536e-6*cos(th1(t)) + 1.0*sin(th1(t))) - 1.3268e-6*sin(th2(t) - 1.5708)*cos(th1(t)))) + cos(th4(t) - 3.1416)*(cos(th3(t) - 1.5708)*(sin(th2(t) - 1.5708)*(2.6536e-6*cos(th1(t)) + 1.0*sin(th1(t))) + 1.3268e-6*cos(th2(t) - 1.5708)*cos(th1(t))) + 1.0*sin(th3(t) - 1.5708)*(1.0*cos(th2(t) - 1.5708)*(2.6536e-6*cos(th1(t)) + 1.0*sin(th1(t))) - 1.3268e-6*sin(th2(t) - 1.5708)*cos(th1(t))))) - 0.02*sin(th5(t))*(cos(th4(t) - 3.1416)*(sin(th3(t) - 1.5708)*(sin(th2(t) - 1.5708)*(2.6536e-6*cos(th1(t)) + 1.0*sin(th1(t))) + 1.3268e-6*cos(th2(t) - 1.5708)*cos(th1(t))) - cos(th3(t) - 1.5708)*(1.0*cos(th2(t) - 1.5708)*(2.6536e-6*cos(th1(t)) + 1.0*sin(th1(t))) - 1.3268e-6*sin(th2(t) - 1.5708)*cos(th1(t)))) - 1.0*sin(th4(t) - 3.1416)*(cos(th3(t) - 1.5708)*(sin(th2(t) - 1.5708)*(2.6536e-6*cos(th1(t)) + 1.0*sin(th1(t))) + 1.3268e-6*cos(th2(t) - 1.5708)*cos(th1(t))) + 1.0*sin(th3(t) - 1.5708)*(1.0*cos(th2(t) - 1.5708)*(2.6536e-6*cos(th1(t)) + 1.0*sin(th1(t))) - 1.3268e-6*sin(th2(t) - 1.5708)*cos(th1(t))))))*(5.0418e-7*sin(th1(t))*sin(th2(t)) - 0.02*cos(th5(t))*(cos(th4(t) - 3.1416)*(cos(th3(t) - 1.5708)*(cos(th2(t) - 1.5708)*(1.0*cos(th1(t)) - 2.6536e-6*sin(th1(t))) + 1.3268e-6*sin(th2(t) - 1.5708)*sin(th1(t))) - sin(th3(t) - 1.5708)*(1.0*sin(th2(t) - 1.5708)*(1.0*cos(th1(t)) - 2.6536e-6*sin(th1(t))) - 1.3268e-6*cos(th2(t) - 1.5708)*sin(th1(t)))) + 1.0*sin(th4(t) - 3.1416)*(1.0*sin(th3(t) - 1.5708)*(cos(th2(t) - 1.5708)*(1.0*cos(th1(t)) - 2.6536e-6*sin(th1(t))) + 1.3268e-6*sin(th2(t) - 1.5708)*sin(th1(t))) + cos(th3(t) - 1.5708)*(1.0*sin(th2(t) - 1.5708)*(1.0*cos(th1(t)) - 2.6536e-6*sin(th1(t))) - 1.3268e-6*cos(th2(t) - 1.5708)*sin(th1(t))))) + 0.38*cos(th2(t))*(1.0*cos(th1(t)) - 2.6536e-6*sin(th1(t))) + 0.38*cos(th3(t))*(cos(th2(t) - 1.5708)*(1.0*cos(th1(t)) - 2.6536e-6*sin(th1(t))) + 1.3268e-6*sin(th2(t) - 1.5708)*sin(th1(t))) + 0.38*cos(th4(t))*(cos(th3(t) - 1.5708)*(cos(th2(t) - 1.5708)*(1.0*cos(th1(t)) - 2.6536e-6*sin(th1(t))) + 1.3268e-6*sin(th2(t) - 1.5708)*sin(th1(t))) - sin(th3(t) - 1.5708)*(1.0*sin(th2(t) - 1.5708)*(1.0*cos(th1(t)) - 2.6536e-6*sin(th1(t))) - 1.3268e-6*cos(th2(t) - 1.5708)*sin(th1(t)))) - 0.38*sin(th3(t))*(1.0*sin(th2(t) - 1.5708)*(1.0*cos(th1(t)) - 2.6536e-6*sin(th1(t))) - 1.3268e-6*cos(th2(t) - 1.5708)*sin(th1(t))) - 0.38*sin(th4(t))*(1.0*sin(th3(t) - 1.5708)*(cos(th2(t) - 1.5708)*(1.0*cos(th1(t)) - 2.6536e-6*sin(th1(t))) + 1.3268e-6*sin(th2(t) - 1.5708)*sin(th1(t))) + cos(th3(t) - 1.5708)*(1.0*sin(th2(t) - 1.5708)*(1.0*cos(th1(t)) - 2.6536e-6*sin(th1(t))) - 1.3268e-6*cos(th2(t) - 1.5708)*sin(th1(t)))) - 0.02*sin(th5(t))*(sin(th4(t) - 3.1416)*(cos(th3(t) - 1.5708)*(cos(th2(t) - 1.5708)*(1.0*cos(th1(t)) - 2.6536e-6*sin(th1(t))) + 1.3268e-6*sin(th2(t) - 1.5708)*sin(th1(t))) - sin(th3(t) - 1.5708)*(1.0*sin(th2(t) - 1.5708)*(1.0*cos(th1(t)) - 2.6536e-6*sin(th1(t))) - 1.3268e-6*cos(th2(t) - 1.5708)*sin(th1(t)))) - cos(th4(t) - 3.1416)*(1.0*sin(th3(t) - 1.5708)*(cos(th2(t) - 1.5708)*(1.0*cos(th1(t)) - 2.6536e-6*sin(th1(t))) + 1.3268e-6*sin(th2(t) - 1.5708)*sin(th1(t))) + cos(th3(t) - 1.5708)*(1.0*sin(th2(t) - 1.5708)*(1.0*cos(th1(t)) - 2.6536e-6*sin(th1(t))) - 1.3268e-6*cos(th2(t) - 1.5708)*sin(th1(t)))))) + 0.00018665;

M21 = Izz2 - 0.13038*(5.0418e-7*sin(th1(t))*sin(th2(t)) - 0.02*cos(th5(t))*(cos(th4(t) - 3.1416)*(cos(th3(t) - 1.5708)*(cos(th2(t) - 1.5708)*(1.0*cos(th1(t)) - 2.6536e-6*sin(th1(t))) + 1.3268e-6*sin(th2(t) - 1.5708)*sin(th1(t))) - sin(th3(t) - 1.5708)*(1.0*sin(th2(t) - 1.5708)*(1.0*cos(th1(t)) - 2.6536e-6*sin(th1(t))) - 1.3268e-6*cos(th2(t) - 1.5708)*sin(th1(t)))) + 1.0*sin(th4(t) - 3.1416)*(1.0*sin(th3(t) - 1.5708)*(cos(th2(t) - 1.5708)*(1.0*cos(th1(t)) - 2.6536e-6*sin(th1(t))) + 1.3268e-6*sin(th2(t) - 1.5708)*sin(th1(t))) + cos(th3(t) - 1.5708)*(1.0*sin(th2(t) - 1.5708)*(1.0*cos(th1(t)) - 2.6536e-6*sin(th1(t))) - 1.3268e-6*cos(th2(t) - 1.5708)*sin(th1(t))))) + 0.38*cos(th2(t))*(1.0*cos(th1(t)) - 2.6536e-6*sin(th1(t))) + 0.38*cos(th3(t))*(cos(th2(t) - 1.5708)*(1.0*cos(th1(t)) - 2.6536e-6*sin(th1(t))) + 1.3268e-6*sin(th2(t) - 1.5708)*sin(th1(t))) + 0.38*cos(th4(t))*(cos(th3(t) - 1.5708)*(cos(th2(t) - 1.5708)*(1.0*cos(th1(t)) - 2.6536e-6*sin(th1(t))) + 1.3268e-6*sin(th2(t) - 1.5708)*sin(th1(t))) - sin(th3(t) - 1.5708)*(1.0*sin(th2(t) - 1.5708)*(1.0*cos(th1(t)) - 2.6536e-6*sin(th1(t))) - 1.3268e-6*cos(th2(t) - 1.5708)*sin(th1(t)))) - 0.38*sin(th3(t))*(1.0*sin(th2(t) - 1.5708)*(1.0*cos(th1(t)) - 2.6536e-6*sin(th1(t))) - 1.3268e-6*cos(th2(t) - 1.5708)*sin(th1(t))) - 0.38*sin(th4(t))*(1.0*sin(th3(t) - 1.5708)*(cos(th2(t) - 1.5708)*(1.0*cos(th1(t)) - 2.6536e-6*sin(th1(t))) + 1.3268e-6*sin(th2(t) - 1.5708)*sin(th1(t))) + cos(th3(t) - 1.5708)*(1.0*sin(th2(t) - 1.5708)*(1.0*cos(th1(t)) - 2.6536e-6*sin(th1(t))) - 1.3268e-6*cos(th2(t) - 1.5708)*sin(th1(t)))) - 0.02*sin(th5(t))*(sin(th4(t) - 3.1416)*(cos(th3(t) - 1.5708)*(cos(th2(t) - 1.5708)*(1.0*cos(th1(t)) - 2.6536e-6*sin(th1(t))) + 1.3268e-6*sin(th2(t) - 1.5708)*sin(th1(t))) - sin(th3(t) - 1.5708)*(1.0*sin(th2(t) - 1.5708)*(1.0*cos(th1(t)) - 2.6536e-6*sin(th1(t))) - 1.3268e-6*cos(th2(t) - 1.5708)*sin(th1(t)))) - cos(th4(t) - 3.1416)*(1.0*sin(th3(t) - 1.5708)*(cos(th2(t) - 1.5708)*(1.0*cos(th1(t)) - 2.6536e-6*sin(th1(t))) + 1.3268e-6*sin(th2(t) - 1.5708)*sin(th1(t))) + cos(th3(t) - 1.5708)*(1.0*sin(th2(t) - 1.5708)*(1.0*cos(th1(t)) - 2.6536e-6*sin(th1(t))) - 1.3268e-6*cos(th2(t) - 1.5708)*sin(th1(t))))))*(0.38*cos(th3(t))*(sin(th2(t) - 1.5708)*(2.6536e-6*cos(th1(t)) + 1.0*sin(th1(t))) + 1.3268e-6*cos(th2(t) - 1.5708)*cos(th1(t))) + 0.38*sin(th2(t))*(2.6536e-6*cos(th1(t)) + 1.0*sin(th1(t))) - 0.38*sin(th4(t))*(sin(th3(t) - 1.5708)*(sin(th2(t) - 1.5708)*(2.6536e-6*cos(th1(t)) + 1.0*sin(th1(t))) + 1.3268e-6*cos(th2(t) - 1.5708)*cos(th1(t))) - cos(th3(t) - 1.5708)*(1.0*cos(th2(t) - 1.5708)*(2.6536e-6*cos(th1(t)) + 1.0*sin(th1(t))) - 1.3268e-6*sin(th2(t) - 1.5708)*cos(th1(t)))) + 0.38*sin(th3(t))*(1.0*cos(th2(t) - 1.5708)*(2.6536e-6*cos(th1(t)) + 1.0*sin(th1(t))) - 1.3268e-6*sin(th2(t) - 1.5708)*cos(th1(t))) - 0.02*cos(th5(t))*(sin(th4(t) - 3.1416)*(sin(th3(t) - 1.5708)*(sin(th2(t) - 1.5708)*(2.6536e-6*cos(th1(t)) + 1.0*sin(th1(t))) + 1.3268e-6*cos(th2(t) - 1.5708)*cos(th1(t))) - cos(th3(t) - 1.5708)*(1.0*cos(th2(t) - 1.5708)*(2.6536e-6*cos(th1(t)) + 1.0*sin(th1(t))) - 1.3268e-6*sin(th2(t) - 1.5708)*cos(th1(t)))) + cos(th4(t) - 3.1416)*(cos(th3(t) - 1.5708)*(sin(th2(t) - 1.5708)*(2.6536e-6*cos(th1(t)) + 1.0*sin(th1(t))) + 1.3268e-6*cos(th2(t) - 1.5708)*cos(th1(t))) + 1.0*sin(th3(t) - 1.5708)*(1.0*cos(th2(t) - 1.5708)*(2.6536e-6*cos(th1(t)) + 1.0*sin(th1(t))) - 1.3268e-6*sin(th2(t) - 1.5708)*cos(th1(t))))) + 0.38*cos(th4(t))*(cos(th3(t) - 1.5708)*(sin(th2(t) - 1.5708)*(2.6536e-6*cos(th1(t)) + 1.0*sin(th1(t))) + 1.3268e-6*cos(th2(t) - 1.5708)*cos(th1(t))) + 1.0*sin(th3(t) - 1.5708)*(1.0*cos(th2(t) - 1.5708)*(2.6536e-6*cos(th1(t)) + 1.0*sin(th1(t))) - 1.3268e-6*sin(th2(t) - 1.5708)*cos(th1(t)))) + 0.02*sin(th5(t))*(cos(th4(t) - 3.1416)*(sin(th3(t) - 1.5708)*(sin(th2(t) - 1.5708)*(2.6536e-6*cos(th1(t)) + 1.0*sin(th1(t))) + 1.3268e-6*cos(th2(t) - 1.5708)*cos(th1(t))) - cos(th3(t) - 1.5708)*(1.0*cos(th2(t) - 1.5708)*(2.6536e-6*cos(th1(t)) + 1.0*sin(th1(t))) - 1.3268e-6*sin(th2(t) - 1.5708)*cos(th1(t)))) - 1.0*sin(th4(t) - 3.1416)*(cos(th3(t) - 1.5708)*(sin(th2(t) - 1.5708)*(2.6536e-6*cos(th1(t)) + 1.0*sin(th1(t))) + 1.3268e-6*cos(th2(t) - 1.5708)*cos(th1(t))) + 1.0*sin(th3(t) - 1.5708)*(1.0*cos(th2(t) - 1.5708)*(2.6536e-6*cos(th1(t)) + 1.0*sin(th1(t))) - 1.3268e-6*sin(th2(t) - 1.5708)*cos(th1(t))))) + 5.0418e-7*cos(th1(t))*cos(th2(t))) + 1.3806*(2.5209e-7*cos(th1(t))*sin(th2(t)) - 0.19*cos(th2(t))*(2.6536e-6*cos(th1(t)) + 1.0*sin(th1(t))))*(2.5209e-7*cos(th2(t))*sin(th1(t)) - 0.19*sin(th2(t))*(1.0*cos(th1(t)) - 2.6536e-6*sin(th1(t)))) - 1.3806*(0.19*sin(th2(t))*(2.6536e-6*cos(th1(t)) + 1.0*sin(th1(t))) + 2.5209e-7*cos(th1(t))*cos(th2(t)))*(2.5209e-7*sin(th1(t))*sin(th2(t)) + 0.19*cos(th2(t))*(1.0*cos(th1(t)) - 2.6536e-6*sin(th1(t)))) - 1.3806*(5.0418e-7*sin(th1(t))*sin(th2(t)) + 0.38*cos(th2(t))*(1.0*cos(th1(t)) - 2.6536e-6*sin(th1(t))) + 0.38*cos(th3(t))*(cos(th2(t) - 1.5708)*(1.0*cos(th1(t)) - 2.6536e-6*sin(th1(t))) + 1.3268e-6*sin(th2(t) - 1.5708)*sin(th1(t))) + 0.19*cos(th4(t))*(cos(th3(t) - 1.5708)*(cos(th2(t) - 1.5708)*(1.0*cos(th1(t)) - 2.6536e-6*sin(th1(t))) + 1.3268e-6*sin(th2(t) - 1.5708)*sin(th1(t))) - sin(th3(t) - 1.5708)*(1.0*sin(th2(t) - 1.5708)*(1.0*cos(th1(t)) - 2.6536e-6*sin(th1(t))) - 1.3268e-6*cos(th2(t) - 1.5708)*sin(th1(t)))) - 0.38*sin(th3(t))*(1.0*sin(th2(t) - 1.5708)*(1.0*cos(th1(t)) - 2.6536e-6*sin(th1(t))) - 1.3268e-6*cos(th2(t) - 1.5708)*sin(th1(t))) - 0.19*sin(th4(t))*(1.0*sin(th3(t) - 1.5708)*(cos(th2(t) - 1.5708)*(1.0*cos(th1(t)) - 2.6536e-6*sin(th1(t))) + 1.3268e-6*sin(th2(t) - 1.5708)*sin(th1(t))) + cos(th3(t) - 1.5708)*(1.0*sin(th2(t) - 1.5708)*(1.0*cos(th1(t)) - 2.6536e-6*sin(th1(t))) - 1.3268e-6*cos(th2(t) - 1.5708)*sin(th1(t)))))*(0.38*cos(th3(t))*(sin(th2(t) - 1.5708)*(2.6536e-6*cos(th1(t)) + 1.0*sin(th1(t))) + 1.3268e-6*cos(th2(t) - 1.5708)*cos(th1(t))) + 0.38*sin(th2(t))*(2.6536e-6*cos(th1(t)) + 1.0*sin(th1(t))) - 0.19*sin(th4(t))*(sin(th3(t) - 1.5708)*(sin(th2(t) - 1.5708)*(2.6536e-6*cos(th1(t)) + 1.0*sin(th1(t))) + 1.3268e-6*cos(th2(t) - 1.5708)*cos(th1(t))) - cos(th3(t) - 1.5708)*(1.0*cos(th2(t) - 1.5708)*(2.6536e-6*cos(th1(t)) + 1.0*sin(th1(t))) - 1.3268e-6*sin(th2(t) - 1.5708)*cos(th1(t)))) + 0.38*sin(th3(t))*(1.0*cos(th2(t) - 1.5708)*(2.6536e-6*cos(th1(t)) + 1.0*sin(th1(t))) - 1.3268e-6*sin(th2(t) - 1.5708)*cos(th1(t))) + 0.19*cos(th4(t))*(cos(th3(t) - 1.5708)*(sin(th2(t) - 1.5708)*(2.6536e-6*cos(th1(t)) + 1.0*sin(th1(t))) + 1.3268e-6*cos(th2(t) - 1.5708)*cos(th1(t))) + 1.0*sin(th3(t) - 1.5708)*(1.0*cos(th2(t) - 1.5708)*(2.6536e-6*cos(th1(t)) + 1.0*sin(th1(t))) - 1.3268e-6*sin(th2(t) - 1.5708)*cos(th1(t)))) + 5.0418e-7*cos(th1(t))*cos(th2(t))) - 0.49277*(5.0418e-7*sin(th1(t))*sin(th2(t)) + 0.38*cos(th2(t))*(1.0*cos(th1(t)) - 2.6536e-6*sin(th1(t))) + 0.19*cos(th3(t))*(cos(th2(t) - 1.5708)*(1.0*cos(th1(t)) - 2.6536e-6*sin(th1(t))) + 1.3268e-6*sin(th2(t) - 1.5708)*sin(th1(t))) - 0.19*sin(th3(t))*(1.0*sin(th2(t) - 1.5708)*(1.0*cos(th1(t)) - 2.6536e-6*sin(th1(t))) - 1.3268e-6*cos(th2(t) - 1.5708)*sin(th1(t))))*(0.19*cos(th3(t))*(sin(th2(t) - 1.5708)*(2.6536e-6*cos(th1(t)) + 1.0*sin(th1(t))) + 1.3268e-6*cos(th2(t) - 1.5708)*cos(th1(t))) + 0.38*sin(th2(t))*(2.6536e-6*cos(th1(t)) + 1.0*sin(th1(t))) + 0.19*sin(th3(t))*(1.0*cos(th2(t) - 1.5708)*(2.6536e-6*cos(th1(t)) + 1.0*sin(th1(t))) - 1.3268e-6*sin(th2(t) - 1.5708)*cos(th1(t))) + 5.0418e-7*cos(th1(t))*cos(th2(t))) - 0.13038*(0.38*cos(th4(t))*(cos(th3(t) - 1.5708)*(sin(th2(t) - 1.5708)*(1.0*cos(th1(t)) - 2.6536e-6*sin(th1(t))) - 1.3268e-6*cos(th2(t) - 1.5708)*sin(th1(t))) + sin(th3(t) - 1.5708)*(cos(th2(t) - 1.5708)*(1.0*cos(th1(t)) - 2.6536e-6*sin(th1(t))) + 1.3268e-6*sin(th2(t) - 1.5708)*sin(th1(t)))) - 5.0418e-7*cos(th2(t))*sin(th1(t)) + 0.38*cos(th3(t))*(sin(th2(t) - 1.5708)*(1.0*cos(th1(t)) - 2.6536e-6*sin(th1(t))) - 1.3268e-6*cos(th2(t) - 1.5708)*sin(th1(t))) + 0.38*sin(th2(t))*(1.0*cos(th1(t)) - 2.6536e-6*sin(th1(t))) + 0.38*sin(th3(t))*(cos(th2(t) - 1.5708)*(1.0*cos(th1(t)) - 2.6536e-6*sin(th1(t))) + 1.3268e-6*sin(th2(t) - 1.5708)*sin(th1(t))) - 0.02*sin(th5(t))*(sin(th4(t) - 3.1416)*(cos(th3(t) - 1.5708)*(sin(th2(t) - 1.5708)*(1.0*cos(th1(t)) - 2.6536e-6*sin(th1(t))) - 1.3268e-6*cos(th2(t) - 1.5708)*sin(th1(t))) + sin(th3(t) - 1.5708)*(cos(th2(t) - 1.5708)*(1.0*cos(th1(t)) - 2.6536e-6*sin(th1(t))) + 1.3268e-6*sin(th2(t) - 1.5708)*sin(th1(t)))) + cos(th4(t) - 3.1416)*(cos(th3(t) - 1.5708)*(cos(th2(t) - 1.5708)*(1.0*cos(th1(t)) - 2.6536e-6*sin(th1(t))) + 1.3268e-6*sin(th2(t) - 1.5708)*sin(th1(t))) - 1.0*sin(th3(t) - 1.5708)*(sin(th2(t) - 1.5708)*(1.0*cos(th1(t)) - 2.6536e-6*sin(th1(t))) - 1.3268e-6*cos(th2(t) - 1.5708)*sin(th1(t))))) + 0.38*sin(th4(t))*(cos(th3(t) - 1.5708)*(cos(th2(t) - 1.5708)*(1.0*cos(th1(t)) - 2.6536e-6*sin(th1(t))) + 1.3268e-6*sin(th2(t) - 1.5708)*sin(th1(t))) - 1.0*sin(th3(t) - 1.5708)*(sin(th2(t) - 1.5708)*(1.0*cos(th1(t)) - 2.6536e-6*sin(th1(t))) - 1.3268e-6*cos(th2(t) - 1.5708)*sin(th1(t)))) - 0.02*cos(th5(t))*(cos(th4(t) - 3.1416)*(cos(th3(t) - 1.5708)*(sin(th2(t) - 1.5708)*(1.0*cos(th1(t)) - 2.6536e-6*sin(th1(t))) - 1.3268e-6*cos(th2(t) - 1.5708)*sin(th1(t))) + sin(th3(t) - 1.5708)*(cos(th2(t) - 1.5708)*(1.0*cos(th1(t)) - 2.6536e-6*sin(th1(t))) + 1.3268e-6*sin(th2(t) - 1.5708)*sin(th1(t)))) - 1.0*sin(th4(t) - 3.1416)*(cos(th3(t) - 1.5708)*(cos(th2(t) - 1.5708)*(1.0*cos(th1(t)) - 2.6536e-6*sin(th1(t))) + 1.3268e-6*sin(th2(t) - 1.5708)*sin(th1(t))) - 1.0*sin(th3(t) - 1.5708)*(sin(th2(t) - 1.5708)*(1.0*cos(th1(t)) - 2.6536e-6*sin(th1(t))) - 1.3268e-6*cos(th2(t) - 1.5708)*sin(th1(t))))))*(5.0418e-7*cos(th1(t))*sin(th2(t)) + 0.02*cos(th5(t))*(cos(th4(t) - 3.1416)*(cos(th3(t) - 1.5708)*(cos(th2(t) - 1.5708)*(2.6536e-6*cos(th1(t)) + 1.0*sin(th1(t))) - 1.3268e-6*sin(th2(t) - 1.5708)*cos(th1(t))) - 1.0*sin(th3(t) - 1.5708)*(sin(th2(t) - 1.5708)*(2.6536e-6*cos(th1(t)) + 1.0*sin(th1(t))) + 1.3268e-6*cos(th2(t) - 1.5708)*cos(th1(t)))) + sin(th4(t) - 3.1416)*(cos(th3(t) - 1.5708)*(sin(th2(t) - 1.5708)*(2.6536e-6*cos(th1(t)) + 1.0*sin(th1(t))) + 1.3268e-6*cos(th2(t) - 1.5708)*cos(th1(t))) + sin(th3(t) - 1.5708)*(cos(th2(t) - 1.5708)*(2.6536e-6*cos(th1(t)) + 1.0*sin(th1(t))) - 1.3268e-6*sin(th2(t) - 1.5708)*cos(th1(t))))) + 0.38*sin(th4(t))*(cos(th3(t) - 1.5708)*(sin(th2(t) - 1.5708)*(2.6536e-6*cos(th1(t)) + 1.0*sin(th1(t))) + 1.3268e-6*cos(th2(t) - 1.5708)*cos(th1(t))) + sin(th3(t) - 1.5708)*(cos(th2(t) - 1.5708)*(2.6536e-6*cos(th1(t)) + 1.0*sin(th1(t))) - 1.3268e-6*sin(th2(t) - 1.5708)*cos(th1(t)))) - 0.38*cos(th3(t))*(cos(th2(t) - 1.5708)*(2.6536e-6*cos(th1(t)) + 1.0*sin(th1(t))) - 1.3268e-6*sin(th2(t) - 1.5708)*cos(th1(t))) - 0.38*cos(th2(t))*(2.6536e-6*cos(th1(t)) + 1.0*sin(th1(t))) + 0.38*sin(th3(t))*(sin(th2(t) - 1.5708)*(2.6536e-6*cos(th1(t)) + 1.0*sin(th1(t))) + 1.3268e-6*cos(th2(t) - 1.5708)*cos(th1(t))) - 0.38*cos(th4(t))*(cos(th3(t) - 1.5708)*(cos(th2(t) - 1.5708)*(2.6536e-6*cos(th1(t)) + 1.0*sin(th1(t))) - 1.3268e-6*sin(th2(t) - 1.5708)*cos(th1(t))) - 1.0*sin(th3(t) - 1.5708)*(sin(th2(t) - 1.5708)*(2.6536e-6*cos(th1(t)) + 1.0*sin(th1(t))) + 1.3268e-6*cos(th2(t) - 1.5708)*cos(th1(t)))) + 0.02*sin(th5(t))*(1.0*sin(th4(t) - 3.1416)*(cos(th3(t) - 1.5708)*(cos(th2(t) - 1.5708)*(2.6536e-6*cos(th1(t)) + 1.0*sin(th1(t))) - 1.3268e-6*sin(th2(t) - 1.5708)*cos(th1(t))) - 1.0*sin(th3(t) - 1.5708)*(sin(th2(t) - 1.5708)*(2.6536e-6*cos(th1(t)) + 1.0*sin(th1(t))) + 1.3268e-6*cos(th2(t) - 1.5708)*cos(th1(t)))) - cos(th4(t) - 3.1416)*(cos(th3(t) - 1.5708)*(sin(th2(t) - 1.5708)*(2.6536e-6*cos(th1(t)) + 1.0*sin(th1(t))) + 1.3268e-6*cos(th2(t) - 1.5708)*cos(th1(t))) + sin(th3(t) - 1.5708)*(cos(th2(t) - 1.5708)*(2.6536e-6*cos(th1(t)) + 1.0*sin(th1(t))) - 1.3268e-6*sin(th2(t) - 1.5708)*cos(th1(t)))))) - 1.3806*(0.19*cos(th4(t))*(cos(th3(t) - 1.5708)*(sin(th2(t) - 1.5708)*(1.0*cos(th1(t)) - 2.6536e-6*sin(th1(t))) - 1.3268e-6*cos(th2(t) - 1.5708)*sin(th1(t))) + sin(th3(t) - 1.5708)*(cos(th2(t) - 1.5708)*(1.0*cos(th1(t)) - 2.6536e-6*sin(th1(t))) + 1.3268e-6*sin(th2(t) - 1.5708)*sin(th1(t)))) - 5.0418e-7*cos(th2(t))*sin(th1(t)) + 0.38*cos(th3(t))*(sin(th2(t) - 1.5708)*(1.0*cos(th1(t)) - 2.6536e-6*sin(th1(t))) - 1.3268e-6*cos(th2(t) - 1.5708)*sin(th1(t))) + 0.38*sin(th2(t))*(1.0*cos(th1(t)) - 2.6536e-6*sin(th1(t))) + 0.38*sin(th3(t))*(cos(th2(t) - 1.5708)*(1.0*cos(th1(t)) - 2.6536e-6*sin(th1(t))) + 1.3268e-6*sin(th2(t) - 1.5708)*sin(th1(t))) + 0.19*sin(th4(t))*(cos(th3(t) - 1.5708)*(cos(th2(t) - 1.5708)*(1.0*cos(th1(t)) - 2.6536e-6*sin(th1(t))) + 1.3268e-6*sin(th2(t) - 1.5708)*sin(th1(t))) - 1.0*sin(th3(t) - 1.5708)*(sin(th2(t) - 1.5708)*(1.0*cos(th1(t)) - 2.6536e-6*sin(th1(t))) - 1.3268e-6*cos(th2(t) - 1.5708)*sin(th1(t)))))*(5.0418e-7*cos(th1(t))*sin(th2(t)) + 0.19*sin(th4(t))*(cos(th3(t) - 1.5708)*(sin(th2(t) - 1.5708)*(2.6536e-6*cos(th1(t)) + 1.0*sin(th1(t))) + 1.3268e-6*cos(th2(t) - 1.5708)*cos(th1(t))) + sin(th3(t) - 1.5708)*(cos(th2(t) - 1.5708)*(2.6536e-6*cos(th1(t)) + 1.0*sin(th1(t))) - 1.3268e-6*sin(th2(t) - 1.5708)*cos(th1(t)))) - 0.38*cos(th3(t))*(cos(th2(t) - 1.5708)*(2.6536e-6*cos(th1(t)) + 1.0*sin(th1(t))) - 1.3268e-6*sin(th2(t) - 1.5708)*cos(th1(t))) - 0.38*cos(th2(t))*(2.6536e-6*cos(th1(t)) + 1.0*sin(th1(t))) + 0.38*sin(th3(t))*(sin(th2(t) - 1.5708)*(2.6536e-6*cos(th1(t)) + 1.0*sin(th1(t))) + 1.3268e-6*cos(th2(t) - 1.5708)*cos(th1(t))) - 0.19*cos(th4(t))*(cos(th3(t) - 1.5708)*(cos(th2(t) - 1.5708)*(2.6536e-6*cos(th1(t)) + 1.0*sin(th1(t))) - 1.3268e-6*sin(th2(t) - 1.5708)*cos(th1(t))) - 1.0*sin(th3(t) - 1.5708)*(sin(th2(t) - 1.5708)*(2.6536e-6*cos(th1(t)) + 1.0*sin(th1(t))) + 1.3268e-6*cos(th2(t) - 1.5708)*cos(th1(t))))) - 0.49277*(5.0418e-7*cos(th1(t))*sin(th2(t)) - 0.19*cos(th3(t))*(cos(th2(t) - 1.5708)*(2.6536e-6*cos(th1(t)) + 1.0*sin(th1(t))) - 1.3268e-6*sin(th2(t) - 1.5708)*cos(th1(t))) - 0.38*cos(th2(t))*(2.6536e-6*cos(th1(t)) + 1.0*sin(th1(t))) + 0.19*sin(th3(t))*(sin(th2(t) - 1.5708)*(2.6536e-6*cos(th1(t)) + 1.0*sin(th1(t))) + 1.3268e-6*cos(th2(t) - 1.5708)*cos(th1(t))))*(0.19*cos(th3(t))*(sin(th2(t) - 1.5708)*(1.0*cos(th1(t)) - 2.6536e-6*sin(th1(t))) - 1.3268e-6*cos(th2(t) - 1.5708)*sin(th1(t))) - 5.0418e-7*cos(th2(t))*sin(th1(t)) + 0.38*sin(th2(t))*(1.0*cos(th1(t)) - 2.6536e-6*sin(th1(t))) + 0.19*sin(th3(t))*(cos(th2(t) - 1.5708)*(1.0*cos(th1(t)) - 2.6536e-6*sin(th1(t))) + 1.3268e-6*sin(th2(t) - 1.5708)*sin(th1(t)))) + 0.051004;
M22 = Izz2 + 1.3806*(0.38*cos(th3(t))*(sin(th2(t) - 1.5708)*(2.6536e-6*cos(th1(t)) + 1.0*sin(th1(t))) + 1.3268e-6*cos(th2(t) - 1.5708)*cos(th1(t))) + 0.38*sin(th2(t))*(2.6536e-6*cos(th1(t)) + 1.0*sin(th1(t))) - 0.19*sin(th4(t))*(sin(th3(t) - 1.5708)*(sin(th2(t) - 1.5708)*(2.6536e-6*cos(th1(t)) + 1.0*sin(th1(t))) + 1.3268e-6*cos(th2(t) - 1.5708)*cos(th1(t))) - cos(th3(t) - 1.5708)*(1.0*cos(th2(t) - 1.5708)*(2.6536e-6*cos(th1(t)) + 1.0*sin(th1(t))) - 1.3268e-6*sin(th2(t) - 1.5708)*cos(th1(t)))) + 0.38*sin(th3(t))*(1.0*cos(th2(t) - 1.5708)*(2.6536e-6*cos(th1(t)) + 1.0*sin(th1(t))) - 1.3268e-6*sin(th2(t) - 1.5708)*cos(th1(t))) + 0.19*cos(th4(t))*(cos(th3(t) - 1.5708)*(sin(th2(t) - 1.5708)*(2.6536e-6*cos(th1(t)) + 1.0*sin(th1(t))) + 1.3268e-6*cos(th2(t) - 1.5708)*cos(th1(t))) + 1.0*sin(th3(t) - 1.5708)*(1.0*cos(th2(t) - 1.5708)*(2.6536e-6*cos(th1(t)) + 1.0*sin(th1(t))) - 1.3268e-6*sin(th2(t) - 1.5708)*cos(th1(t)))) + 5.0418e-7*cos(th1(t))*cos(th2(t)))^2 + 0.49277*(0.19*cos(th3(t))*(sin(th2(t) - 1.5708)*(1.0*cos(th1(t)) - 2.6536e-6*sin(th1(t))) - 1.3268e-6*cos(th2(t) - 1.5708)*sin(th1(t))) - 5.0418e-7*cos(th2(t))*sin(th1(t)) + 0.38*sin(th2(t))*(1.0*cos(th1(t)) - 2.6536e-6*sin(th1(t))) + 0.19*sin(th3(t))*(cos(th2(t) - 1.5708)*(1.0*cos(th1(t)) - 2.6536e-6*sin(th1(t))) + 1.3268e-6*sin(th2(t) - 1.5708)*sin(th1(t))))^2 + 0.13038*(0.38*cos(th3(t))*(sin(th2(t) - 1.5708)*(2.6536e-6*cos(th1(t)) + 1.0*sin(th1(t))) + 1.3268e-6*cos(th2(t) - 1.5708)*cos(th1(t))) + 0.38*sin(th2(t))*(2.6536e-6*cos(th1(t)) + 1.0*sin(th1(t))) - 0.38*sin(th4(t))*(sin(th3(t) - 1.5708)*(sin(th2(t) - 1.5708)*(2.6536e-6*cos(th1(t)) + 1.0*sin(th1(t))) + 1.3268e-6*cos(th2(t) - 1.5708)*cos(th1(t))) - cos(th3(t) - 1.5708)*(1.0*cos(th2(t) - 1.5708)*(2.6536e-6*cos(th1(t)) + 1.0*sin(th1(t))) - 1.3268e-6*sin(th2(t) - 1.5708)*cos(th1(t)))) + 0.38*sin(th3(t))*(1.0*cos(th2(t) - 1.5708)*(2.6536e-6*cos(th1(t)) + 1.0*sin(th1(t))) - 1.3268e-6*sin(th2(t) - 1.5708)*cos(th1(t))) - 0.02*cos(th5(t))*(sin(th4(t) - 3.1416)*(sin(th3(t) - 1.5708)*(sin(th2(t) - 1.5708)*(2.6536e-6*cos(th1(t)) + 1.0*sin(th1(t))) + 1.3268e-6*cos(th2(t) - 1.5708)*cos(th1(t))) - cos(th3(t) - 1.5708)*(1.0*cos(th2(t) - 1.5708)*(2.6536e-6*cos(th1(t)) + 1.0*sin(th1(t))) - 1.3268e-6*sin(th2(t) - 1.5708)*cos(th1(t)))) + cos(th4(t) - 3.1416)*(cos(th3(t) - 1.5708)*(sin(th2(t) - 1.5708)*(2.6536e-6*cos(th1(t)) + 1.0*sin(th1(t))) + 1.3268e-6*cos(th2(t) - 1.5708)*cos(th1(t))) + 1.0*sin(th3(t) - 1.5708)*(1.0*cos(th2(t) - 1.5708)*(2.6536e-6*cos(th1(t)) + 1.0*sin(th1(t))) - 1.3268e-6*sin(th2(t) - 1.5708)*cos(th1(t))))) + 0.38*cos(th4(t))*(cos(th3(t) - 1.5708)*(sin(th2(t) - 1.5708)*(2.6536e-6*cos(th1(t)) + 1.0*sin(th1(t))) + 1.3268e-6*cos(th2(t) - 1.5708)*cos(th1(t))) + 1.0*sin(th3(t) - 1.5708)*(1.0*cos(th2(t) - 1.5708)*(2.6536e-6*cos(th1(t)) + 1.0*sin(th1(t))) - 1.3268e-6*sin(th2(t) - 1.5708)*cos(th1(t)))) + 0.02*sin(th5(t))*(cos(th4(t) - 3.1416)*(sin(th3(t) - 1.5708)*(sin(th2(t) - 1.5708)*(2.6536e-6*cos(th1(t)) + 1.0*sin(th1(t))) + 1.3268e-6*cos(th2(t) - 1.5708)*cos(th1(t))) - cos(th3(t) - 1.5708)*(1.0*cos(th2(t) - 1.5708)*(2.6536e-6*cos(th1(t)) + 1.0*sin(th1(t))) - 1.3268e-6*sin(th2(t) - 1.5708)*cos(th1(t)))) - 1.0*sin(th4(t) - 3.1416)*(cos(th3(t) - 1.5708)*(sin(th2(t) - 1.5708)*(2.6536e-6*cos(th1(t)) + 1.0*sin(th1(t))) + 1.3268e-6*cos(th2(t) - 1.5708)*cos(th1(t))) + 1.0*sin(th3(t) - 1.5708)*(1.0*cos(th2(t) - 1.5708)*(2.6536e-6*cos(th1(t)) + 1.0*sin(th1(t))) - 1.3268e-6*sin(th2(t) - 1.5708)*cos(th1(t))))) + 5.0418e-7*cos(th1(t))*cos(th2(t)))^2 + 0.49277*(0.19*cos(th3(t))*(sin(th2(t) - 1.5708)*(2.6536e-6*cos(th1(t)) + 1.0*sin(th1(t))) + 1.3268e-6*cos(th2(t) - 1.5708)*cos(th1(t))) + 0.38*sin(th2(t))*(2.6536e-6*cos(th1(t)) + 1.0*sin(th1(t))) + 0.19*sin(th3(t))*(1.0*cos(th2(t) - 1.5708)*(2.6536e-6*cos(th1(t)) + 1.0*sin(th1(t))) - 1.3268e-6*sin(th2(t) - 1.5708)*cos(th1(t))) + 5.0418e-7*cos(th1(t))*cos(th2(t)))^2 + 0.13038*(0.38*cos(th4(t))*(cos(th3(t) - 1.5708)*(sin(th2(t) - 1.5708)*(1.0*cos(th1(t)) - 2.6536e-6*sin(th1(t))) - 1.3268e-6*cos(th2(t) - 1.5708)*sin(th1(t))) + sin(th3(t) - 1.5708)*(cos(th2(t) - 1.5708)*(1.0*cos(th1(t)) - 2.6536e-6*sin(th1(t))) + 1.3268e-6*sin(th2(t) - 1.5708)*sin(th1(t)))) - 5.0418e-7*cos(th2(t))*sin(th1(t)) + 0.38*cos(th3(t))*(sin(th2(t) - 1.5708)*(1.0*cos(th1(t)) - 2.6536e-6*sin(th1(t))) - 1.3268e-6*cos(th2(t) - 1.5708)*sin(th1(t))) + 0.38*sin(th2(t))*(1.0*cos(th1(t)) - 2.6536e-6*sin(th1(t))) + 0.38*sin(th3(t))*(cos(th2(t) - 1.5708)*(1.0*cos(th1(t)) - 2.6536e-6*sin(th1(t))) + 1.3268e-6*sin(th2(t) - 1.5708)*sin(th1(t))) - 0.02*sin(th5(t))*(sin(th4(t) - 3.1416)*(cos(th3(t) - 1.5708)*(sin(th2(t) - 1.5708)*(1.0*cos(th1(t)) - 2.6536e-6*sin(th1(t))) - 1.3268e-6*cos(th2(t) - 1.5708)*sin(th1(t))) + sin(th3(t) - 1.5708)*(cos(th2(t) - 1.5708)*(1.0*cos(th1(t)) - 2.6536e-6*sin(th1(t))) + 1.3268e-6*sin(th2(t) - 1.5708)*sin(th1(t)))) + cos(th4(t) - 3.1416)*(cos(th3(t) - 1.5708)*(cos(th2(t) - 1.5708)*(1.0*cos(th1(t)) - 2.6536e-6*sin(th1(t))) + 1.3268e-6*sin(th2(t) - 1.5708)*sin(th1(t))) - 1.0*sin(th3(t) - 1.5708)*(sin(th2(t) - 1.5708)*(1.0*cos(th1(t)) - 2.6536e-6*sin(th1(t))) - 1.3268e-6*cos(th2(t) - 1.5708)*sin(th1(t))))) + 0.38*sin(th4(t))*(cos(th3(t) - 1.5708)*(cos(th2(t) - 1.5708)*(1.0*cos(th1(t)) - 2.6536e-6*sin(th1(t))) + 1.3268e-6*sin(th2(t) - 1.5708)*sin(th1(t))) - 1.0*sin(th3(t) - 1.5708)*(sin(th2(t) - 1.5708)*(1.0*cos(th1(t)) - 2.6536e-6*sin(th1(t))) - 1.3268e-6*cos(th2(t) - 1.5708)*sin(th1(t)))) - 0.02*cos(th5(t))*(cos(th4(t) - 3.1416)*(cos(th3(t) - 1.5708)*(sin(th2(t) - 1.5708)*(1.0*cos(th1(t)) - 2.6536e-6*sin(th1(t))) - 1.3268e-6*cos(th2(t) - 1.5708)*sin(th1(t))) + sin(th3(t) - 1.5708)*(cos(th2(t) - 1.5708)*(1.0*cos(th1(t)) - 2.6536e-6*sin(th1(t))) + 1.3268e-6*sin(th2(t) - 1.5708)*sin(th1(t)))) - 1.0*sin(th4(t) - 3.1416)*(cos(th3(t) - 1.5708)*(cos(th2(t) - 1.5708)*(1.0*cos(th1(t)) - 2.6536e-6*sin(th1(t))) + 1.3268e-6*sin(th2(t) - 1.5708)*sin(th1(t))) - 1.0*sin(th3(t) - 1.5708)*(sin(th2(t) - 1.5708)*(1.0*cos(th1(t)) - 2.6536e-6*sin(th1(t))) - 1.3268e-6*cos(th2(t) - 1.5708)*sin(th1(t))))))^2 + 0.49277*(0.38*cos(th2(t)) - 1.3379e-12*sin(th2(t)) - 0.19*sin(th3(t))*(3.5208e-12*cos(th2(t) - 1.5708) + 1.0*sin(th2(t) - 1.5708)) + 0.19*cos(th3(t))*(1.0*cos(th2(t) - 1.5708) - 3.5208e-12*sin(th2(t) - 1.5708)))^2 + 1.3806*(0.19*sin(th2(t))*(2.6536e-6*cos(th1(t)) + 1.0*sin(th1(t))) + 2.5209e-7*cos(th1(t))*cos(th2(t)))^2 + 0.13038*(0.38*cos(th2(t)) - 1.3379e-12*sin(th2(t)) - 0.38*sin(th3(t))*(3.5208e-12*cos(th2(t) - 1.5708) + 1.0*sin(th2(t) - 1.5708)) + 0.02*sin(th5(t))*(cos(th4(t) - 3.1416)*(cos(th3(t) - 1.5708)*(3.5208e-12*cos(th2(t) - 1.5708) + 1.0*sin(th2(t) - 1.5708)) + sin(th3(t) - 1.5708)*(1.0*cos(th2(t) - 1.5708) - 3.5208e-12*sin(th2(t) - 1.5708))) - 1.0*sin(th4(t) - 3.1416)*(cos(th3(t) - 1.5708)*(1.0*cos(th2(t) - 1.5708) - 3.5208e-12*sin(th2(t) - 1.5708)) - 1.0*sin(th3(t) - 1.5708)*(3.5208e-12*cos(th2(t) - 1.5708) + 1.0*sin(th2(t) - 1.5708)))) - 0.38*sin(th4(t))*(cos(th3(t) - 1.5708)*(3.5208e-12*cos(th2(t) - 1.5708) + 1.0*sin(th2(t) - 1.5708)) + sin(th3(t) - 1.5708)*(1.0*cos(th2(t) - 1.5708) - 3.5208e-12*sin(th2(t) - 1.5708))) + 0.38*cos(th4(t))*(cos(th3(t) - 1.5708)*(1.0*cos(th2(t) - 1.5708) - 3.5208e-12*sin(th2(t) - 1.5708)) - 1.0*sin(th3(t) - 1.5708)*(3.5208e-12*cos(th2(t) - 1.5708) + 1.0*sin(th2(t) - 1.5708))) + 0.38*cos(th3(t))*(1.0*cos(th2(t) - 1.5708) - 3.5208e-12*sin(th2(t) - 1.5708)) - 0.02*cos(th5(t))*(sin(th4(t) - 3.1416)*(cos(th3(t) - 1.5708)*(3.5208e-12*cos(th2(t) - 1.5708) + 1.0*sin(th2(t) - 1.5708)) + sin(th3(t) - 1.5708)*(1.0*cos(th2(t) - 1.5708) - 3.5208e-12*sin(th2(t) - 1.5708))) + cos(th4(t) - 3.1416)*(cos(th3(t) - 1.5708)*(1.0*cos(th2(t) - 1.5708) - 3.5208e-12*sin(th2(t) - 1.5708)) - 1.0*sin(th3(t) - 1.5708)*(3.5208e-12*cos(th2(t) - 1.5708) + 1.0*sin(th2(t) - 1.5708)))))^2 + 1.3806*(0.19*cos(th4(t))*(cos(th3(t) - 1.5708)*(sin(th2(t) - 1.5708)*(1.0*cos(th1(t)) - 2.6536e-6*sin(th1(t))) - 1.3268e-6*cos(th2(t) - 1.5708)*sin(th1(t))) + sin(th3(t) - 1.5708)*(cos(th2(t) - 1.5708)*(1.0*cos(th1(t)) - 2.6536e-6*sin(th1(t))) + 1.3268e-6*sin(th2(t) - 1.5708)*sin(th1(t)))) - 5.0418e-7*cos(th2(t))*sin(th1(t)) + 0.38*cos(th3(t))*(sin(th2(t) - 1.5708)*(1.0*cos(th1(t)) - 2.6536e-6*sin(th1(t))) - 1.3268e-6*cos(th2(t) - 1.5708)*sin(th1(t))) + 0.38*sin(th2(t))*(1.0*cos(th1(t)) - 2.6536e-6*sin(th1(t))) + 0.38*sin(th3(t))*(cos(th2(t) - 1.5708)*(1.0*cos(th1(t)) - 2.6536e-6*sin(th1(t))) + 1.3268e-6*sin(th2(t) - 1.5708)*sin(th1(t))) + 0.19*sin(th4(t))*(cos(th3(t) - 1.5708)*(cos(th2(t) - 1.5708)*(1.0*cos(th1(t)) - 2.6536e-6*sin(th1(t))) + 1.3268e-6*sin(th2(t) - 1.5708)*sin(th1(t))) - 1.0*sin(th3(t) - 1.5708)*(sin(th2(t) - 1.5708)*(1.0*cos(th1(t)) - 2.6536e-6*sin(th1(t))) - 1.3268e-6*cos(th2(t) - 1.5708)*sin(th1(t)))))^2 + 1.3806*(2.5209e-7*cos(th2(t))*sin(th1(t)) - 0.19*sin(th2(t))*(1.0*cos(th1(t)) - 2.6536e-6*sin(th1(t))))^2 + 1.3806*(0.38*cos(th2(t)) - 1.3379e-12*sin(th2(t)) - 0.38*sin(th3(t))*(3.5208e-12*cos(th2(t) - 1.5708) + 1.0*sin(th2(t) - 1.5708)) - 0.19*sin(th4(t))*(cos(th3(t) - 1.5708)*(3.5208e-12*cos(th2(t) - 1.5708) + 1.0*sin(th2(t) - 1.5708)) + sin(th3(t) - 1.5708)*(1.0*cos(th2(t) - 1.5708) - 3.5208e-12*sin(th2(t) - 1.5708))) + 0.19*cos(th4(t))*(cos(th3(t) - 1.5708)*(1.0*cos(th2(t) - 1.5708) - 3.5208e-12*sin(th2(t) - 1.5708)) - 1.0*sin(th3(t) - 1.5708)*(3.5208e-12*cos(th2(t) - 1.5708) + 1.0*sin(th2(t) - 1.5708))) + 0.38*cos(th3(t))*(1.0*cos(th2(t) - 1.5708) - 3.5208e-12*sin(th2(t) - 1.5708)))^2 + 1.3806*(0.19*cos(th2(t)) - 6.6895e-13*sin(th2(t)))^2 + 0.051004;
M23 = 1.3806*(0.19*cos(th4(t))*(cos(th3(t) - 1.5708)*(sin(th2(t) - 1.5708)*(1.0*cos(th1(t)) - 2.6536e-6*sin(th1(t))) - 1.3268e-6*cos(th2(t) - 1.5708)*sin(th1(t))) + sin(th3(t) - 1.5708)*(cos(th2(t) - 1.5708)*(1.0*cos(th1(t)) - 2.6536e-6*sin(th1(t))) + 1.3268e-6*sin(th2(t) - 1.5708)*sin(th1(t)))) + 0.38*cos(th3(t))*(sin(th2(t) - 1.5708)*(1.0*cos(th1(t)) - 2.6536e-6*sin(th1(t))) - 1.3268e-6*cos(th2(t) - 1.5708)*sin(th1(t))) + 0.38*sin(th3(t))*(cos(th2(t) - 1.5708)*(1.0*cos(th1(t)) - 2.6536e-6*sin(th1(t))) + 1.3268e-6*sin(th2(t) - 1.5708)*sin(th1(t))) + 0.19*sin(th4(t))*(cos(th3(t) - 1.5708)*(cos(th2(t) - 1.5708)*(1.0*cos(th1(t)) - 2.6536e-6*sin(th1(t))) + 1.3268e-6*sin(th2(t) - 1.5708)*sin(th1(t))) - 1.0*sin(th3(t) - 1.5708)*(sin(th2(t) - 1.5708)*(1.0*cos(th1(t)) - 2.6536e-6*sin(th1(t))) - 1.3268e-6*cos(th2(t) - 1.5708)*sin(th1(t)))))*(0.19*cos(th4(t))*(cos(th3(t) - 1.5708)*(sin(th2(t) - 1.5708)*(1.0*cos(th1(t)) - 2.6536e-6*sin(th1(t))) - 1.3268e-6*cos(th2(t) - 1.5708)*sin(th1(t))) + sin(th3(t) - 1.5708)*(cos(th2(t) - 1.5708)*(1.0*cos(th1(t)) - 2.6536e-6*sin(th1(t))) + 1.3268e-6*sin(th2(t) - 1.5708)*sin(th1(t)))) - 5.0418e-7*cos(th2(t))*sin(th1(t)) + 0.38*cos(th3(t))*(sin(th2(t) - 1.5708)*(1.0*cos(th1(t)) - 2.6536e-6*sin(th1(t))) - 1.3268e-6*cos(th2(t) - 1.5708)*sin(th1(t))) + 0.38*sin(th2(t))*(1.0*cos(th1(t)) - 2.6536e-6*sin(th1(t))) + 0.38*sin(th3(t))*(cos(th2(t) - 1.5708)*(1.0*cos(th1(t)) - 2.6536e-6*sin(th1(t))) + 1.3268e-6*sin(th2(t) - 1.5708)*sin(th1(t))) + 0.19*sin(th4(t))*(cos(th3(t) - 1.5708)*(cos(th2(t) - 1.5708)*(1.0*cos(th1(t)) - 2.6536e-6*sin(th1(t))) + 1.3268e-6*sin(th2(t) - 1.5708)*sin(th1(t))) - 1.0*sin(th3(t) - 1.5708)*(sin(th2(t) - 1.5708)*(1.0*cos(th1(t)) - 2.6536e-6*sin(th1(t))) - 1.3268e-6*cos(th2(t) - 1.5708)*sin(th1(t))))) - 1.3806*(0.38*sin(th3(t))*(3.5208e-12*cos(th2(t) - 1.5708) + 1.0*sin(th2(t) - 1.5708)) + 0.19*sin(th4(t))*(cos(th3(t) - 1.5708)*(3.5208e-12*cos(th2(t) - 1.5708) + 1.0*sin(th2(t) - 1.5708)) + sin(th3(t) - 1.5708)*(1.0*cos(th2(t) - 1.5708) - 3.5208e-12*sin(th2(t) - 1.5708))) - 0.19*cos(th4(t))*(cos(th3(t) - 1.5708)*(1.0*cos(th2(t) - 1.5708) - 3.5208e-12*sin(th2(t) - 1.5708)) - 1.0*sin(th3(t) - 1.5708)*(3.5208e-12*cos(th2(t) - 1.5708) + 1.0*sin(th2(t) - 1.5708))) - 0.38*cos(th3(t))*(1.0*cos(th2(t) - 1.5708) - 3.5208e-12*sin(th2(t) - 1.5708)))*(0.38*cos(th2(t)) - 1.3379e-12*sin(th2(t)) - 0.38*sin(th3(t))*(3.5208e-12*cos(th2(t) - 1.5708) + 1.0*sin(th2(t) - 1.5708)) - 0.19*sin(th4(t))*(cos(th3(t) - 1.5708)*(3.5208e-12*cos(th2(t) - 1.5708) + 1.0*sin(th2(t) - 1.5708)) + sin(th3(t) - 1.5708)*(1.0*cos(th2(t) - 1.5708) - 3.5208e-12*sin(th2(t) - 1.5708))) + 0.19*cos(th4(t))*(cos(th3(t) - 1.5708)*(1.0*cos(th2(t) - 1.5708) - 3.5208e-12*sin(th2(t) - 1.5708)) - 1.0*sin(th3(t) - 1.5708)*(3.5208e-12*cos(th2(t) - 1.5708) + 1.0*sin(th2(t) - 1.5708))) + 0.38*cos(th3(t))*(1.0*cos(th2(t) - 1.5708) - 3.5208e-12*sin(th2(t) - 1.5708))) + 0.13038*(0.38*cos(th3(t))*(sin(th2(t) - 1.5708)*(2.6536e-6*cos(th1(t)) + 1.0*sin(th1(t))) + 1.3268e-6*cos(th2(t) - 1.5708)*cos(th1(t))) - 0.38*sin(th4(t))*(sin(th3(t) - 1.5708)*(sin(th2(t) - 1.5708)*(2.6536e-6*cos(th1(t)) + 1.0*sin(th1(t))) + 1.3268e-6*cos(th2(t) - 1.5708)*cos(th1(t))) - cos(th3(t) - 1.5708)*(1.0*cos(th2(t) - 1.5708)*(2.6536e-6*cos(th1(t)) + 1.0*sin(th1(t))) - 1.3268e-6*sin(th2(t) - 1.5708)*cos(th1(t)))) + 0.38*sin(th3(t))*(1.0*cos(th2(t) - 1.5708)*(2.6536e-6*cos(th1(t)) + 1.0*sin(th1(t))) - 1.3268e-6*sin(th2(t) - 1.5708)*cos(th1(t))) - 0.02*cos(th5(t))*(sin(th4(t) - 3.1416)*(sin(th3(t) - 1.5708)*(sin(th2(t) - 1.5708)*(2.6536e-6*cos(th1(t)) + 1.0*sin(th1(t))) + 1.3268e-6*cos(th2(t) - 1.5708)*cos(th1(t))) - cos(th3(t) - 1.5708)*(1.0*cos(th2(t) - 1.5708)*(2.6536e-6*cos(th1(t)) + 1.0*sin(th1(t))) - 1.3268e-6*sin(th2(t) - 1.5708)*cos(th1(t)))) + cos(th4(t) - 3.1416)*(cos(th3(t) - 1.5708)*(sin(th2(t) - 1.5708)*(2.6536e-6*cos(th1(t)) + 1.0*sin(th1(t))) + 1.3268e-6*cos(th2(t) - 1.5708)*cos(th1(t))) + 1.0*sin(th3(t) - 1.5708)*(1.0*cos(th2(t) - 1.5708)*(2.6536e-6*cos(th1(t)) + 1.0*sin(th1(t))) - 1.3268e-6*sin(th2(t) - 1.5708)*cos(th1(t))))) + 0.38*cos(th4(t))*(cos(th3(t) - 1.5708)*(sin(th2(t) - 1.5708)*(2.6536e-6*cos(th1(t)) + 1.0*sin(th1(t))) + 1.3268e-6*cos(th2(t) - 1.5708)*cos(th1(t))) + 1.0*sin(th3(t) - 1.5708)*(1.0*cos(th2(t) - 1.5708)*(2.6536e-6*cos(th1(t)) + 1.0*sin(th1(t))) - 1.3268e-6*sin(th2(t) - 1.5708)*cos(th1(t)))) + 0.02*sin(th5(t))*(cos(th4(t) - 3.1416)*(sin(th3(t) - 1.5708)*(sin(th2(t) - 1.5708)*(2.6536e-6*cos(th1(t)) + 1.0*sin(th1(t))) + 1.3268e-6*cos(th2(t) - 1.5708)*cos(th1(t))) - cos(th3(t) - 1.5708)*(1.0*cos(th2(t) - 1.5708)*(2.6536e-6*cos(th1(t)) + 1.0*sin(th1(t))) - 1.3268e-6*sin(th2(t) - 1.5708)*cos(th1(t)))) - 1.0*sin(th4(t) - 3.1416)*(cos(th3(t) - 1.5708)*(sin(th2(t) - 1.5708)*(2.6536e-6*cos(th1(t)) + 1.0*sin(th1(t))) + 1.3268e-6*cos(th2(t) - 1.5708)*cos(th1(t))) + 1.0*sin(th3(t) - 1.5708)*(1.0*cos(th2(t) - 1.5708)*(2.6536e-6*cos(th1(t)) + 1.0*sin(th1(t))) - 1.3268e-6*sin(th2(t) - 1.5708)*cos(th1(t))))))*(0.38*cos(th3(t))*(sin(th2(t) - 1.5708)*(2.6536e-6*cos(th1(t)) + 1.0*sin(th1(t))) + 1.3268e-6*cos(th2(t) - 1.5708)*cos(th1(t))) + 0.38*sin(th2(t))*(2.6536e-6*cos(th1(t)) + 1.0*sin(th1(t))) - 0.38*sin(th4(t))*(sin(th3(t) - 1.5708)*(sin(th2(t) - 1.5708)*(2.6536e-6*cos(th1(t)) + 1.0*sin(th1(t))) + 1.3268e-6*cos(th2(t) - 1.5708)*cos(th1(t))) - cos(th3(t) - 1.5708)*(1.0*cos(th2(t) - 1.5708)*(2.6536e-6*cos(th1(t)) + 1.0*sin(th1(t))) - 1.3268e-6*sin(th2(t) - 1.5708)*cos(th1(t)))) + 0.38*sin(th3(t))*(1.0*cos(th2(t) - 1.5708)*(2.6536e-6*cos(th1(t)) + 1.0*sin(th1(t))) - 1.3268e-6*sin(th2(t) - 1.5708)*cos(th1(t))) - 0.02*cos(th5(t))*(sin(th4(t) - 3.1416)*(sin(th3(t) - 1.5708)*(sin(th2(t) - 1.5708)*(2.6536e-6*cos(th1(t)) + 1.0*sin(th1(t))) + 1.3268e-6*cos(th2(t) - 1.5708)*cos(th1(t))) - cos(th3(t) - 1.5708)*(1.0*cos(th2(t) - 1.5708)*(2.6536e-6*cos(th1(t)) + 1.0*sin(th1(t))) - 1.3268e-6*sin(th2(t) - 1.5708)*cos(th1(t)))) + cos(th4(t) - 3.1416)*(cos(th3(t) - 1.5708)*(sin(th2(t) - 1.5708)*(2.6536e-6*cos(th1(t)) + 1.0*sin(th1(t))) + 1.3268e-6*cos(th2(t) - 1.5708)*cos(th1(t))) + 1.0*sin(th3(t) - 1.5708)*(1.0*cos(th2(t) - 1.5708)*(2.6536e-6*cos(th1(t)) + 1.0*sin(th1(t))) - 1.3268e-6*sin(th2(t) - 1.5708)*cos(th1(t))))) + 0.38*cos(th4(t))*(cos(th3(t) - 1.5708)*(sin(th2(t) - 1.5708)*(2.6536e-6*cos(th1(t)) + 1.0*sin(th1(t))) + 1.3268e-6*cos(th2(t) - 1.5708)*cos(th1(t))) + 1.0*sin(th3(t) - 1.5708)*(1.0*cos(th2(t) - 1.5708)*(2.6536e-6*cos(th1(t)) + 1.0*sin(th1(t))) - 1.3268e-6*sin(th2(t) - 1.5708)*cos(th1(t)))) + 0.02*sin(th5(t))*(cos(th4(t) - 3.1416)*(sin(th3(t) - 1.5708)*(sin(th2(t) - 1.5708)*(2.6536e-6*cos(th1(t)) + 1.0*sin(th1(t))) + 1.3268e-6*cos(th2(t) - 1.5708)*cos(th1(t))) - cos(th3(t) - 1.5708)*(1.0*cos(th2(t) - 1.5708)*(2.6536e-6*cos(th1(t)) + 1.0*sin(th1(t))) - 1.3268e-6*sin(th2(t) - 1.5708)*cos(th1(t)))) - 1.0*sin(th4(t) - 3.1416)*(cos(th3(t) - 1.5708)*(sin(th2(t) - 1.5708)*(2.6536e-6*cos(th1(t)) + 1.0*sin(th1(t))) + 1.3268e-6*cos(th2(t) - 1.5708)*cos(th1(t))) + 1.0*sin(th3(t) - 1.5708)*(1.0*cos(th2(t) - 1.5708)*(2.6536e-6*cos(th1(t)) + 1.0*sin(th1(t))) - 1.3268e-6*sin(th2(t) - 1.5708)*cos(th1(t))))) + 5.0418e-7*cos(th1(t))*cos(th2(t))) + 0.49277*(0.19*cos(th3(t))*(sin(th2(t) - 1.5708)*(2.6536e-6*cos(th1(t)) + 1.0*sin(th1(t))) + 1.3268e-6*cos(th2(t) - 1.5708)*cos(th1(t))) + 0.19*sin(th3(t))*(1.0*cos(th2(t) - 1.5708)*(2.6536e-6*cos(th1(t)) + 1.0*sin(th1(t))) - 1.3268e-6*sin(th2(t) - 1.5708)*cos(th1(t))))*(0.19*cos(th3(t))*(sin(th2(t) - 1.5708)*(2.6536e-6*cos(th1(t)) + 1.0*sin(th1(t))) + 1.3268e-6*cos(th2(t) - 1.5708)*cos(th1(t))) + 0.38*sin(th2(t))*(2.6536e-6*cos(th1(t)) + 1.0*sin(th1(t))) + 0.19*sin(th3(t))*(1.0*cos(th2(t) - 1.5708)*(2.6536e-6*cos(th1(t)) + 1.0*sin(th1(t))) - 1.3268e-6*sin(th2(t) - 1.5708)*cos(th1(t))) + 5.0418e-7*cos(th1(t))*cos(th2(t))) + 0.13038*(0.38*cos(th4(t))*(cos(th3(t) - 1.5708)*(sin(th2(t) - 1.5708)*(1.0*cos(th1(t)) - 2.6536e-6*sin(th1(t))) - 1.3268e-6*cos(th2(t) - 1.5708)*sin(th1(t))) + sin(th3(t) - 1.5708)*(cos(th2(t) - 1.5708)*(1.0*cos(th1(t)) - 2.6536e-6*sin(th1(t))) + 1.3268e-6*sin(th2(t) - 1.5708)*sin(th1(t)))) + 0.38*cos(th3(t))*(sin(th2(t) - 1.5708)*(1.0*cos(th1(t)) - 2.6536e-6*sin(th1(t))) - 1.3268e-6*cos(th2(t) - 1.5708)*sin(th1(t))) + 0.38*sin(th3(t))*(cos(th2(t) - 1.5708)*(1.0*cos(th1(t)) - 2.6536e-6*sin(th1(t))) + 1.3268e-6*sin(th2(t) - 1.5708)*sin(th1(t))) - 0.02*sin(th5(t))*(sin(th4(t) - 3.1416)*(cos(th3(t) - 1.5708)*(sin(th2(t) - 1.5708)*(1.0*cos(th1(t)) - 2.6536e-6*sin(th1(t))) - 1.3268e-6*cos(th2(t) - 1.5708)*sin(th1(t))) + sin(th3(t) - 1.5708)*(cos(th2(t) - 1.5708)*(1.0*cos(th1(t)) - 2.6536e-6*sin(th1(t))) + 1.3268e-6*sin(th2(t) - 1.5708)*sin(th1(t)))) + cos(th4(t) - 3.1416)*(cos(th3(t) - 1.5708)*(cos(th2(t) - 1.5708)*(1.0*cos(th1(t)) - 2.6536e-6*sin(th1(t))) + 1.3268e-6*sin(th2(t) - 1.5708)*sin(th1(t))) - 1.0*sin(th3(t) - 1.5708)*(sin(th2(t) - 1.5708)*(1.0*cos(th1(t)) - 2.6536e-6*sin(th1(t))) - 1.3268e-6*cos(th2(t) - 1.5708)*sin(th1(t))))) + 0.38*sin(th4(t))*(cos(th3(t) - 1.5708)*(cos(th2(t) - 1.5708)*(1.0*cos(th1(t)) - 2.6536e-6*sin(th1(t))) + 1.3268e-6*sin(th2(t) - 1.5708)*sin(th1(t))) - 1.0*sin(th3(t) - 1.5708)*(sin(th2(t) - 1.5708)*(1.0*cos(th1(t)) - 2.6536e-6*sin(th1(t))) - 1.3268e-6*cos(th2(t) - 1.5708)*sin(th1(t)))) - 0.02*cos(th5(t))*(cos(th4(t) - 3.1416)*(cos(th3(t) - 1.5708)*(sin(th2(t) - 1.5708)*(1.0*cos(th1(t)) - 2.6536e-6*sin(th1(t))) - 1.3268e-6*cos(th2(t) - 1.5708)*sin(th1(t))) + sin(th3(t) - 1.5708)*(cos(th2(t) - 1.5708)*(1.0*cos(th1(t)) - 2.6536e-6*sin(th1(t))) + 1.3268e-6*sin(th2(t) - 1.5708)*sin(th1(t)))) - 1.0*sin(th4(t) - 3.1416)*(cos(th3(t) - 1.5708)*(cos(th2(t) - 1.5708)*(1.0*cos(th1(t)) - 2.6536e-6*sin(th1(t))) + 1.3268e-6*sin(th2(t) - 1.5708)*sin(th1(t))) - 1.0*sin(th3(t) - 1.5708)*(sin(th2(t) - 1.5708)*(1.0*cos(th1(t)) - 2.6536e-6*sin(th1(t))) - 1.3268e-6*cos(th2(t) - 1.5708)*sin(th1(t))))))*(0.38*cos(th4(t))*(cos(th3(t) - 1.5708)*(sin(th2(t) - 1.5708)*(1.0*cos(th1(t)) - 2.6536e-6*sin(th1(t))) - 1.3268e-6*cos(th2(t) - 1.5708)*sin(th1(t))) + sin(th3(t) - 1.5708)*(cos(th2(t) - 1.5708)*(1.0*cos(th1(t)) - 2.6536e-6*sin(th1(t))) + 1.3268e-6*sin(th2(t) - 1.5708)*sin(th1(t)))) - 5.0418e-7*cos(th2(t))*sin(th1(t)) + 0.38*cos(th3(t))*(sin(th2(t) - 1.5708)*(1.0*cos(th1(t)) - 2.6536e-6*sin(th1(t))) - 1.3268e-6*cos(th2(t) - 1.5708)*sin(th1(t))) + 0.38*sin(th2(t))*(1.0*cos(th1(t)) - 2.6536e-6*sin(th1(t))) + 0.38*sin(th3(t))*(cos(th2(t) - 1.5708)*(1.0*cos(th1(t)) - 2.6536e-6*sin(th1(t))) + 1.3268e-6*sin(th2(t) - 1.5708)*sin(th1(t))) - 0.02*sin(th5(t))*(sin(th4(t) - 3.1416)*(cos(th3(t) - 1.5708)*(sin(th2(t) - 1.5708)*(1.0*cos(th1(t)) - 2.6536e-6*sin(th1(t))) - 1.3268e-6*cos(th2(t) - 1.5708)*sin(th1(t))) + sin(th3(t) - 1.5708)*(cos(th2(t) - 1.5708)*(1.0*cos(th1(t)) - 2.6536e-6*sin(th1(t))) + 1.3268e-6*sin(th2(t) - 1.5708)*sin(th1(t)))) + cos(th4(t) - 3.1416)*(cos(th3(t) - 1.5708)*(cos(th2(t) - 1.5708)*(1.0*cos(th1(t)) - 2.6536e-6*sin(th1(t))) + 1.3268e-6*sin(th2(t) - 1.5708)*sin(th1(t))) - 1.0*sin(th3(t) - 1.5708)*(sin(th2(t) - 1.5708)*(1.0*cos(th1(t)) - 2.6536e-6*sin(th1(t))) - 1.3268e-6*cos(th2(t) - 1.5708)*sin(th1(t))))) + 0.38*sin(th4(t))*(cos(th3(t) - 1.5708)*(cos(th2(t) - 1.5708)*(1.0*cos(th1(t)) - 2.6536e-6*sin(th1(t))) + 1.3268e-6*sin(th2(t) - 1.5708)*sin(th1(t))) - 1.0*sin(th3(t) - 1.5708)*(sin(th2(t) - 1.5708)*(1.0*cos(th1(t)) - 2.6536e-6*sin(th1(t))) - 1.3268e-6*cos(th2(t) - 1.5708)*sin(th1(t)))) - 0.02*cos(th5(t))*(cos(th4(t) - 3.1416)*(cos(th3(t) - 1.5708)*(sin(th2(t) - 1.5708)*(1.0*cos(th1(t)) - 2.6536e-6*sin(th1(t))) - 1.3268e-6*cos(th2(t) - 1.5708)*sin(th1(t))) + sin(th3(t) - 1.5708)*(cos(th2(t) - 1.5708)*(1.0*cos(th1(t)) - 2.6536e-6*sin(th1(t))) + 1.3268e-6*sin(th2(t) - 1.5708)*sin(th1(t)))) - 1.0*sin(th4(t) - 3.1416)*(cos(th3(t) - 1.5708)*(cos(th2(t) - 1.5708)*(1.0*cos(th1(t)) - 2.6536e-6*sin(th1(t))) + 1.3268e-6*sin(th2(t) - 1.5708)*sin(th1(t))) - 1.0*sin(th3(t) - 1.5708)*(sin(th2(t) - 1.5708)*(1.0*cos(th1(t)) - 2.6536e-6*sin(th1(t))) - 1.3268e-6*cos(th2(t) - 1.5708)*sin(th1(t)))))) - 0.49277*(0.19*sin(th3(t))*(3.5208e-12*cos(th2(t) - 1.5708) + 1.0*sin(th2(t) - 1.5708)) - 0.19*cos(th3(t))*(1.0*cos(th2(t) - 1.5708) - 3.5208e-12*sin(th2(t) - 1.5708)))*(0.38*cos(th2(t)) - 1.3379e-12*sin(th2(t)) - 0.19*sin(th3(t))*(3.5208e-12*cos(th2(t) - 1.5708) + 1.0*sin(th2(t) - 1.5708)) + 0.19*cos(th3(t))*(1.0*cos(th2(t) - 1.5708) - 3.5208e-12*sin(th2(t) - 1.5708))) + 1.3806*(0.38*cos(th3(t))*(sin(th2(t) - 1.5708)*(2.6536e-6*cos(th1(t)) + 1.0*sin(th1(t))) + 1.3268e-6*cos(th2(t) - 1.5708)*cos(th1(t))) - 0.19*sin(th4(t))*(sin(th3(t) - 1.5708)*(sin(th2(t) - 1.5708)*(2.6536e-6*cos(th1(t)) + 1.0*sin(th1(t))) + 1.3268e-6*cos(th2(t) - 1.5708)*cos(th1(t))) - cos(th3(t) - 1.5708)*(1.0*cos(th2(t) - 1.5708)*(2.6536e-6*cos(th1(t)) + 1.0*sin(th1(t))) - 1.3268e-6*sin(th2(t) - 1.5708)*cos(th1(t)))) + 0.38*sin(th3(t))*(1.0*cos(th2(t) - 1.5708)*(2.6536e-6*cos(th1(t)) + 1.0*sin(th1(t))) - 1.3268e-6*sin(th2(t) - 1.5708)*cos(th1(t))) + 0.19*cos(th4(t))*(cos(th3(t) - 1.5708)*(sin(th2(t) - 1.5708)*(2.6536e-6*cos(th1(t)) + 1.0*sin(th1(t))) + 1.3268e-6*cos(th2(t) - 1.5708)*cos(th1(t))) + 1.0*sin(th3(t) - 1.5708)*(1.0*cos(th2(t) - 1.5708)*(2.6536e-6*cos(th1(t)) + 1.0*sin(th1(t))) - 1.3268e-6*sin(th2(t) - 1.5708)*cos(th1(t)))))*(0.38*cos(th3(t))*(sin(th2(t) - 1.5708)*(2.6536e-6*cos(th1(t)) + 1.0*sin(th1(t))) + 1.3268e-6*cos(th2(t) - 1.5708)*cos(th1(t))) + 0.38*sin(th2(t))*(2.6536e-6*cos(th1(t)) + 1.0*sin(th1(t))) - 0.19*sin(th4(t))*(sin(th3(t) - 1.5708)*(sin(th2(t) - 1.5708)*(2.6536e-6*cos(th1(t)) + 1.0*sin(th1(t))) + 1.3268e-6*cos(th2(t) - 1.5708)*cos(th1(t))) - cos(th3(t) - 1.5708)*(1.0*cos(th2(t) - 1.5708)*(2.6536e-6*cos(th1(t)) + 1.0*sin(th1(t))) - 1.3268e-6*sin(th2(t) - 1.5708)*cos(th1(t)))) + 0.38*sin(th3(t))*(1.0*cos(th2(t) - 1.5708)*(2.6536e-6*cos(th1(t)) + 1.0*sin(th1(t))) - 1.3268e-6*sin(th2(t) - 1.5708)*cos(th1(t))) + 0.19*cos(th4(t))*(cos(th3(t) - 1.5708)*(sin(th2(t) - 1.5708)*(2.6536e-6*cos(th1(t)) + 1.0*sin(th1(t))) + 1.3268e-6*cos(th2(t) - 1.5708)*cos(th1(t))) + 1.0*sin(th3(t) - 1.5708)*(1.0*cos(th2(t) - 1.5708)*(2.6536e-6*cos(th1(t)) + 1.0*sin(th1(t))) - 1.3268e-6*sin(th2(t) - 1.5708)*cos(th1(t)))) + 5.0418e-7*cos(th1(t))*cos(th2(t))) - 0.13038*(0.38*sin(th3(t))*(3.5208e-12*cos(th2(t) - 1.5708) + 1.0*sin(th2(t) - 1.5708)) - 0.02*sin(th5(t))*(cos(th4(t) - 3.1416)*(cos(th3(t) - 1.5708)*(3.5208e-12*cos(th2(t) - 1.5708) + 1.0*sin(th2(t) - 1.5708)) + sin(th3(t) - 1.5708)*(1.0*cos(th2(t) - 1.5708) - 3.5208e-12*sin(th2(t) - 1.5708))) - 1.0*sin(th4(t) - 3.1416)*(cos(th3(t) - 1.5708)*(1.0*cos(th2(t) - 1.5708) - 3.5208e-12*sin(th2(t) - 1.5708)) - 1.0*sin(th3(t) - 1.5708)*(3.5208e-12*cos(th2(t) - 1.5708) + 1.0*sin(th2(t) - 1.5708)))) + 0.38*sin(th4(t))*(cos(th3(t) - 1.5708)*(3.5208e-12*cos(th2(t) - 1.5708) + 1.0*sin(th2(t) - 1.5708)) + sin(th3(t) - 1.5708)*(1.0*cos(th2(t) - 1.5708) - 3.5208e-12*sin(th2(t) - 1.5708))) - 0.38*cos(th4(t))*(cos(th3(t) - 1.5708)*(1.0*cos(th2(t) - 1.5708) - 3.5208e-12*sin(th2(t) - 1.5708)) - 1.0*sin(th3(t) - 1.5708)*(3.5208e-12*cos(th2(t) - 1.5708) + 1.0*sin(th2(t) - 1.5708))) - 0.38*cos(th3(t))*(1.0*cos(th2(t) - 1.5708) - 3.5208e-12*sin(th2(t) - 1.5708)) + 0.02*cos(th5(t))*(sin(th4(t) - 3.1416)*(cos(th3(t) - 1.5708)*(3.5208e-12*cos(th2(t) - 1.5708) + 1.0*sin(th2(t) - 1.5708)) + sin(th3(t) - 1.5708)*(1.0*cos(th2(t) - 1.5708) - 3.5208e-12*sin(th2(t) - 1.5708))) + cos(th4(t) - 3.1416)*(cos(th3(t) - 1.5708)*(1.0*cos(th2(t) - 1.5708) - 3.5208e-12*sin(th2(t) - 1.5708)) - 1.0*sin(th3(t) - 1.5708)*(3.5208e-12*cos(th2(t) - 1.5708) + 1.0*sin(th2(t) - 1.5708)))))*(0.38*cos(th2(t)) - 1.3379e-12*sin(th2(t)) - 0.38*sin(th3(t))*(3.5208e-12*cos(th2(t) - 1.5708) + 1.0*sin(th2(t) - 1.5708)) + 0.02*sin(th5(t))*(cos(th4(t) - 3.1416)*(cos(th3(t) - 1.5708)*(3.5208e-12*cos(th2(t) - 1.5708) + 1.0*sin(th2(t) - 1.5708)) + sin(th3(t) - 1.5708)*(1.0*cos(th2(t) - 1.5708) - 3.5208e-12*sin(th2(t) - 1.5708))) - 1.0*sin(th4(t) - 3.1416)*(cos(th3(t) - 1.5708)*(1.0*cos(th2(t) - 1.5708) - 3.5208e-12*sin(th2(t) - 1.5708)) - 1.0*sin(th3(t) - 1.5708)*(3.5208e-12*cos(th2(t) - 1.5708) + 1.0*sin(th2(t) - 1.5708)))) - 0.38*sin(th4(t))*(cos(th3(t) - 1.5708)*(3.5208e-12*cos(th2(t) - 1.5708) + 1.0*sin(th2(t) - 1.5708)) + sin(th3(t) - 1.5708)*(1.0*cos(th2(t) - 1.5708) - 3.5208e-12*sin(th2(t) - 1.5708))) + 0.38*cos(th4(t))*(cos(th3(t) - 1.5708)*(1.0*cos(th2(t) - 1.5708) - 3.5208e-12*sin(th2(t) - 1.5708)) - 1.0*sin(th3(t) - 1.5708)*(3.5208e-12*cos(th2(t) - 1.5708) + 1.0*sin(th2(t) - 1.5708))) + 0.38*cos(th3(t))*(1.0*cos(th2(t) - 1.5708) - 3.5208e-12*sin(th2(t) - 1.5708)) - 0.02*cos(th5(t))*(sin(th4(t) - 3.1416)*(cos(th3(t) - 1.5708)*(3.5208e-12*cos(th2(t) - 1.5708) + 1.0*sin(th2(t) - 1.5708)) + sin(th3(t) - 1.5708)*(1.0*cos(th2(t) - 1.5708) - 3.5208e-12*sin(th2(t) - 1.5708))) + cos(th4(t) - 3.1416)*(cos(th3(t) - 1.5708)*(1.0*cos(th2(t) - 1.5708) - 3.5208e-12*sin(th2(t) - 1.5708)) - 1.0*sin(th3(t) - 1.5708)*(3.5208e-12*cos(th2(t) - 1.5708) + 1.0*sin(th2(t) - 1.5708))))) + 0.49277*(0.19*cos(th3(t))*(sin(th2(t) - 1.5708)*(1.0*cos(th1(t)) - 2.6536e-6*sin(th1(t))) - 1.3268e-6*cos(th2(t) - 1.5708)*sin(th1(t))) + 0.19*sin(th3(t))*(cos(th2(t) - 1.5708)*(1.0*cos(th1(t)) - 2.6536e-6*sin(th1(t))) + 1.3268e-6*sin(th2(t) - 1.5708)*sin(th1(t))))*(0.19*cos(th3(t))*(sin(th2(t) - 1.5708)*(1.0*cos(th1(t)) - 2.6536e-6*sin(th1(t))) - 1.3268e-6*cos(th2(t) - 1.5708)*sin(th1(t))) - 5.0418e-7*cos(th2(t))*sin(th1(t)) + 0.38*sin(th2(t))*(1.0*cos(th1(t)) - 2.6536e-6*sin(th1(t))) + 0.19*sin(th3(t))*(cos(th2(t) - 1.5708)*(1.0*cos(th1(t)) - 2.6536e-6*sin(th1(t))) + 1.3268e-6*sin(th2(t) - 1.5708)*sin(th1(t)))) + 0.051004;
M24 = 0.13038*(0.38*cos(th4(t))*(cos(th3(t) - 1.5708)*(sin(th2(t) - 1.5708)*(1.0*cos(th1(t)) - 2.6536e-6*sin(th1(t))) - 1.3268e-6*cos(th2(t) - 1.5708)*sin(th1(t))) + sin(th3(t) - 1.5708)*(cos(th2(t) - 1.5708)*(1.0*cos(th1(t)) - 2.6536e-6*sin(th1(t))) + 1.3268e-6*sin(th2(t) - 1.5708)*sin(th1(t)))) + 0.02*sin(th5(t))*(sin(th4(t) - 3.1416)*(cos(th3(t) - 1.5708)*(sin(th2(t) - 1.5708)*(1.0*cos(th1(t)) - 2.6536e-6*sin(th1(t))) - 1.3268e-6*cos(th2(t) - 1.5708)*sin(th1(t))) + sin(th3(t) - 1.5708)*(cos(th2(t) - 1.5708)*(1.0*cos(th1(t)) - 2.6536e-6*sin(th1(t))) + 1.3268e-6*sin(th2(t) - 1.5708)*sin(th1(t)))) + cos(th4(t) - 3.1416)*(cos(th3(t) - 1.5708)*(cos(th2(t) - 1.5708)*(1.0*cos(th1(t)) - 2.6536e-6*sin(th1(t))) + 1.3268e-6*sin(th2(t) - 1.5708)*sin(th1(t))) - 1.0*sin(th3(t) - 1.5708)*(sin(th2(t) - 1.5708)*(1.0*cos(th1(t)) - 2.6536e-6*sin(th1(t))) - 1.3268e-6*cos(th2(t) - 1.5708)*sin(th1(t))))) + 0.38*sin(th4(t))*(cos(th3(t) - 1.5708)*(cos(th2(t) - 1.5708)*(1.0*cos(th1(t)) - 2.6536e-6*sin(th1(t))) + 1.3268e-6*sin(th2(t) - 1.5708)*sin(th1(t))) - 1.0*sin(th3(t) - 1.5708)*(sin(th2(t) - 1.5708)*(1.0*cos(th1(t)) - 2.6536e-6*sin(th1(t))) - 1.3268e-6*cos(th2(t) - 1.5708)*sin(th1(t)))) + 0.02*cos(th5(t))*(cos(th4(t) - 3.1416)*(cos(th3(t) - 1.5708)*(sin(th2(t) - 1.5708)*(1.0*cos(th1(t)) - 2.6536e-6*sin(th1(t))) - 1.3268e-6*cos(th2(t) - 1.5708)*sin(th1(t))) + sin(th3(t) - 1.5708)*(cos(th2(t) - 1.5708)*(1.0*cos(th1(t)) - 2.6536e-6*sin(th1(t))) + 1.3268e-6*sin(th2(t) - 1.5708)*sin(th1(t)))) - 1.0*sin(th4(t) - 3.1416)*(cos(th3(t) - 1.5708)*(cos(th2(t) - 1.5708)*(1.0*cos(th1(t)) - 2.6536e-6*sin(th1(t))) + 1.3268e-6*sin(th2(t) - 1.5708)*sin(th1(t))) - 1.0*sin(th3(t) - 1.5708)*(sin(th2(t) - 1.5708)*(1.0*cos(th1(t)) - 2.6536e-6*sin(th1(t))) - 1.3268e-6*cos(th2(t) - 1.5708)*sin(th1(t))))))*(0.38*cos(th4(t))*(cos(th3(t) - 1.5708)*(sin(th2(t) - 1.5708)*(1.0*cos(th1(t)) - 2.6536e-6*sin(th1(t))) - 1.3268e-6*cos(th2(t) - 1.5708)*sin(th1(t))) + sin(th3(t) - 1.5708)*(cos(th2(t) - 1.5708)*(1.0*cos(th1(t)) - 2.6536e-6*sin(th1(t))) + 1.3268e-6*sin(th2(t) - 1.5708)*sin(th1(t)))) - 5.0418e-7*cos(th2(t))*sin(th1(t)) + 0.38*cos(th3(t))*(sin(th2(t) - 1.5708)*(1.0*cos(th1(t)) - 2.6536e-6*sin(th1(t))) - 1.3268e-6*cos(th2(t) - 1.5708)*sin(th1(t))) + 0.38*sin(th2(t))*(1.0*cos(th1(t)) - 2.6536e-6*sin(th1(t))) + 0.38*sin(th3(t))*(cos(th2(t) - 1.5708)*(1.0*cos(th1(t)) - 2.6536e-6*sin(th1(t))) + 1.3268e-6*sin(th2(t) - 1.5708)*sin(th1(t))) - 0.02*sin(th5(t))*(sin(th4(t) - 3.1416)*(cos(th3(t) - 1.5708)*(sin(th2(t) - 1.5708)*(1.0*cos(th1(t)) - 2.6536e-6*sin(th1(t))) - 1.3268e-6*cos(th2(t) - 1.5708)*sin(th1(t))) + sin(th3(t) - 1.5708)*(cos(th2(t) - 1.5708)*(1.0*cos(th1(t)) - 2.6536e-6*sin(th1(t))) + 1.3268e-6*sin(th2(t) - 1.5708)*sin(th1(t)))) + cos(th4(t) - 3.1416)*(cos(th3(t) - 1.5708)*(cos(th2(t) - 1.5708)*(1.0*cos(th1(t)) - 2.6536e-6*sin(th1(t))) + 1.3268e-6*sin(th2(t) - 1.5708)*sin(th1(t))) - 1.0*sin(th3(t) - 1.5708)*(sin(th2(t) - 1.5708)*(1.0*cos(th1(t)) - 2.6536e-6*sin(th1(t))) - 1.3268e-6*cos(th2(t) - 1.5708)*sin(th1(t))))) + 0.38*sin(th4(t))*(cos(th3(t) - 1.5708)*(cos(th2(t) - 1.5708)*(1.0*cos(th1(t)) - 2.6536e-6*sin(th1(t))) + 1.3268e-6*sin(th2(t) - 1.5708)*sin(th1(t))) - 1.0*sin(th3(t) - 1.5708)*(sin(th2(t) - 1.5708)*(1.0*cos(th1(t)) - 2.6536e-6*sin(th1(t))) - 1.3268e-6*cos(th2(t) - 1.5708)*sin(th1(t)))) - 0.02*cos(th5(t))*(cos(th4(t) - 3.1416)*(cos(th3(t) - 1.5708)*(sin(th2(t) - 1.5708)*(1.0*cos(th1(t)) - 2.6536e-6*sin(th1(t))) - 1.3268e-6*cos(th2(t) - 1.5708)*sin(th1(t))) + sin(th3(t) - 1.5708)*(cos(th2(t) - 1.5708)*(1.0*cos(th1(t)) - 2.6536e-6*sin(th1(t))) + 1.3268e-6*sin(th2(t) - 1.5708)*sin(th1(t)))) - 1.0*sin(th4(t) - 3.1416)*(cos(th3(t) - 1.5708)*(cos(th2(t) - 1.5708)*(1.0*cos(th1(t)) - 2.6536e-6*sin(th1(t))) + 1.3268e-6*sin(th2(t) - 1.5708)*sin(th1(t))) - 1.0*sin(th3(t) - 1.5708)*(sin(th2(t) - 1.5708)*(1.0*cos(th1(t)) - 2.6536e-6*sin(th1(t))) - 1.3268e-6*cos(th2(t) - 1.5708)*sin(th1(t)))))) - 0.13038*(0.02*sin(th5(t))*(cos(th4(t) - 3.1416)*(cos(th3(t) - 1.5708)*(3.5208e-12*cos(th2(t) - 1.5708) + 1.0*sin(th2(t) - 1.5708)) + sin(th3(t) - 1.5708)*(1.0*cos(th2(t) - 1.5708) - 3.5208e-12*sin(th2(t) - 1.5708))) - 1.0*sin(th4(t) - 3.1416)*(cos(th3(t) - 1.5708)*(1.0*cos(th2(t) - 1.5708) - 3.5208e-12*sin(th2(t) - 1.5708)) - 1.0*sin(th3(t) - 1.5708)*(3.5208e-12*cos(th2(t) - 1.5708) + 1.0*sin(th2(t) - 1.5708)))) + 0.38*sin(th4(t))*(cos(th3(t) - 1.5708)*(3.5208e-12*cos(th2(t) - 1.5708) + 1.0*sin(th2(t) - 1.5708)) + sin(th3(t) - 1.5708)*(1.0*cos(th2(t) - 1.5708) - 3.5208e-12*sin(th2(t) - 1.5708))) - 0.38*cos(th4(t))*(cos(th3(t) - 1.5708)*(1.0*cos(th2(t) - 1.5708) - 3.5208e-12*sin(th2(t) - 1.5708)) - 1.0*sin(th3(t) - 1.5708)*(3.5208e-12*cos(th2(t) - 1.5708) + 1.0*sin(th2(t) - 1.5708))) - 0.02*cos(th5(t))*(sin(th4(t) - 3.1416)*(cos(th3(t) - 1.5708)*(3.5208e-12*cos(th2(t) - 1.5708) + 1.0*sin(th2(t) - 1.5708)) + sin(th3(t) - 1.5708)*(1.0*cos(th2(t) - 1.5708) - 3.5208e-12*sin(th2(t) - 1.5708))) + cos(th4(t) - 3.1416)*(cos(th3(t) - 1.5708)*(1.0*cos(th2(t) - 1.5708) - 3.5208e-12*sin(th2(t) - 1.5708)) - 1.0*sin(th3(t) - 1.5708)*(3.5208e-12*cos(th2(t) - 1.5708) + 1.0*sin(th2(t) - 1.5708)))))*(0.38*cos(th2(t)) - 1.3379e-12*sin(th2(t)) - 0.38*sin(th3(t))*(3.5208e-12*cos(th2(t) - 1.5708) + 1.0*sin(th2(t) - 1.5708)) + 0.02*sin(th5(t))*(cos(th4(t) - 3.1416)*(cos(th3(t) - 1.5708)*(3.5208e-12*cos(th2(t) - 1.5708) + 1.0*sin(th2(t) - 1.5708)) + sin(th3(t) - 1.5708)*(1.0*cos(th2(t) - 1.5708) - 3.5208e-12*sin(th2(t) - 1.5708))) - 1.0*sin(th4(t) - 3.1416)*(cos(th3(t) - 1.5708)*(1.0*cos(th2(t) - 1.5708) - 3.5208e-12*sin(th2(t) - 1.5708)) - 1.0*sin(th3(t) - 1.5708)*(3.5208e-12*cos(th2(t) - 1.5708) + 1.0*sin(th2(t) - 1.5708)))) - 0.38*sin(th4(t))*(cos(th3(t) - 1.5708)*(3.5208e-12*cos(th2(t) - 1.5708) + 1.0*sin(th2(t) - 1.5708)) + sin(th3(t) - 1.5708)*(1.0*cos(th2(t) - 1.5708) - 3.5208e-12*sin(th2(t) - 1.5708))) + 0.38*cos(th4(t))*(cos(th3(t) - 1.5708)*(1.0*cos(th2(t) - 1.5708) - 3.5208e-12*sin(th2(t) - 1.5708)) - 1.0*sin(th3(t) - 1.5708)*(3.5208e-12*cos(th2(t) - 1.5708) + 1.0*sin(th2(t) - 1.5708))) + 0.38*cos(th3(t))*(1.0*cos(th2(t) - 1.5708) - 3.5208e-12*sin(th2(t) - 1.5708)) - 0.02*cos(th5(t))*(sin(th4(t) - 3.1416)*(cos(th3(t) - 1.5708)*(3.5208e-12*cos(th2(t) - 1.5708) + 1.0*sin(th2(t) - 1.5708)) + sin(th3(t) - 1.5708)*(1.0*cos(th2(t) - 1.5708) - 3.5208e-12*sin(th2(t) - 1.5708))) + cos(th4(t) - 3.1416)*(cos(th3(t) - 1.5708)*(1.0*cos(th2(t) - 1.5708) - 3.5208e-12*sin(th2(t) - 1.5708)) - 1.0*sin(th3(t) - 1.5708)*(3.5208e-12*cos(th2(t) - 1.5708) + 1.0*sin(th2(t) - 1.5708))))) - 1.3806*(0.19*sin(th4(t))*(sin(th3(t) - 1.5708)*(sin(th2(t) - 1.5708)*(2.6536e-6*cos(th1(t)) + 1.0*sin(th1(t))) + 1.3268e-6*cos(th2(t) - 1.5708)*cos(th1(t))) - cos(th3(t) - 1.5708)*(1.0*cos(th2(t) - 1.5708)*(2.6536e-6*cos(th1(t)) + 1.0*sin(th1(t))) - 1.3268e-6*sin(th2(t) - 1.5708)*cos(th1(t)))) - 0.19*cos(th4(t))*(cos(th3(t) - 1.5708)*(sin(th2(t) - 1.5708)*(2.6536e-6*cos(th1(t)) + 1.0*sin(th1(t))) + 1.3268e-6*cos(th2(t) - 1.5708)*cos(th1(t))) + 1.0*sin(th3(t) - 1.5708)*(1.0*cos(th2(t) - 1.5708)*(2.6536e-6*cos(th1(t)) + 1.0*sin(th1(t))) - 1.3268e-6*sin(th2(t) - 1.5708)*cos(th1(t)))))*(0.38*cos(th3(t))*(sin(th2(t) - 1.5708)*(2.6536e-6*cos(th1(t)) + 1.0*sin(th1(t))) + 1.3268e-6*cos(th2(t) - 1.5708)*cos(th1(t))) + 0.38*sin(th2(t))*(2.6536e-6*cos(th1(t)) + 1.0*sin(th1(t))) - 0.19*sin(th4(t))*(sin(th3(t) - 1.5708)*(sin(th2(t) - 1.5708)*(2.6536e-6*cos(th1(t)) + 1.0*sin(th1(t))) + 1.3268e-6*cos(th2(t) - 1.5708)*cos(th1(t))) - cos(th3(t) - 1.5708)*(1.0*cos(th2(t) - 1.5708)*(2.6536e-6*cos(th1(t)) + 1.0*sin(th1(t))) - 1.3268e-6*sin(th2(t) - 1.5708)*cos(th1(t)))) + 0.38*sin(th3(t))*(1.0*cos(th2(t) - 1.5708)*(2.6536e-6*cos(th1(t)) + 1.0*sin(th1(t))) - 1.3268e-6*sin(th2(t) - 1.5708)*cos(th1(t))) + 0.19*cos(th4(t))*(cos(th3(t) - 1.5708)*(sin(th2(t) - 1.5708)*(2.6536e-6*cos(th1(t)) + 1.0*sin(th1(t))) + 1.3268e-6*cos(th2(t) - 1.5708)*cos(th1(t))) + 1.0*sin(th3(t) - 1.5708)*(1.0*cos(th2(t) - 1.5708)*(2.6536e-6*cos(th1(t)) + 1.0*sin(th1(t))) - 1.3268e-6*sin(th2(t) - 1.5708)*cos(th1(t)))) + 5.0418e-7*cos(th1(t))*cos(th2(t))) - 1.3806*(0.19*sin(th4(t))*(cos(th3(t) - 1.5708)*(3.5208e-12*cos(th2(t) - 1.5708) + 1.0*sin(th2(t) - 1.5708)) + sin(th3(t) - 1.5708)*(1.0*cos(th2(t) - 1.5708) - 3.5208e-12*sin(th2(t) - 1.5708))) - 0.19*cos(th4(t))*(cos(th3(t) - 1.5708)*(1.0*cos(th2(t) - 1.5708) - 3.5208e-12*sin(th2(t) - 1.5708)) - 1.0*sin(th3(t) - 1.5708)*(3.5208e-12*cos(th2(t) - 1.5708) + 1.0*sin(th2(t) - 1.5708))))*(0.38*cos(th2(t)) - 1.3379e-12*sin(th2(t)) - 0.38*sin(th3(t))*(3.5208e-12*cos(th2(t) - 1.5708) + 1.0*sin(th2(t) - 1.5708)) - 0.19*sin(th4(t))*(cos(th3(t) - 1.5708)*(3.5208e-12*cos(th2(t) - 1.5708) + 1.0*sin(th2(t) - 1.5708)) + sin(th3(t) - 1.5708)*(1.0*cos(th2(t) - 1.5708) - 3.5208e-12*sin(th2(t) - 1.5708))) + 0.19*cos(th4(t))*(cos(th3(t) - 1.5708)*(1.0*cos(th2(t) - 1.5708) - 3.5208e-12*sin(th2(t) - 1.5708)) - 1.0*sin(th3(t) - 1.5708)*(3.5208e-12*cos(th2(t) - 1.5708) + 1.0*sin(th2(t) - 1.5708))) + 0.38*cos(th3(t))*(1.0*cos(th2(t) - 1.5708) - 3.5208e-12*sin(th2(t) - 1.5708))) - 0.13038*(0.38*sin(th4(t))*(sin(th3(t) - 1.5708)*(sin(th2(t) - 1.5708)*(2.6536e-6*cos(th1(t)) + 1.0*sin(th1(t))) + 1.3268e-6*cos(th2(t) - 1.5708)*cos(th1(t))) - cos(th3(t) - 1.5708)*(1.0*cos(th2(t) - 1.5708)*(2.6536e-6*cos(th1(t)) + 1.0*sin(th1(t))) - 1.3268e-6*sin(th2(t) - 1.5708)*cos(th1(t)))) - 0.02*cos(th5(t))*(sin(th4(t) - 3.1416)*(sin(th3(t) - 1.5708)*(sin(th2(t) - 1.5708)*(2.6536e-6*cos(th1(t)) + 1.0*sin(th1(t))) + 1.3268e-6*cos(th2(t) - 1.5708)*cos(th1(t))) - cos(th3(t) - 1.5708)*(1.0*cos(th2(t) - 1.5708)*(2.6536e-6*cos(th1(t)) + 1.0*sin(th1(t))) - 1.3268e-6*sin(th2(t) - 1.5708)*cos(th1(t)))) + cos(th4(t) - 3.1416)*(cos(th3(t) - 1.5708)*(sin(th2(t) - 1.5708)*(2.6536e-6*cos(th1(t)) + 1.0*sin(th1(t))) + 1.3268e-6*cos(th2(t) - 1.5708)*cos(th1(t))) + 1.0*sin(th3(t) - 1.5708)*(1.0*cos(th2(t) - 1.5708)*(2.6536e-6*cos(th1(t)) + 1.0*sin(th1(t))) - 1.3268e-6*sin(th2(t) - 1.5708)*cos(th1(t))))) - 0.38*cos(th4(t))*(cos(th3(t) - 1.5708)*(sin(th2(t) - 1.5708)*(2.6536e-6*cos(th1(t)) + 1.0*sin(th1(t))) + 1.3268e-6*cos(th2(t) - 1.5708)*cos(th1(t))) + 1.0*sin(th3(t) - 1.5708)*(1.0*cos(th2(t) - 1.5708)*(2.6536e-6*cos(th1(t)) + 1.0*sin(th1(t))) - 1.3268e-6*sin(th2(t) - 1.5708)*cos(th1(t)))) + 0.02*sin(th5(t))*(cos(th4(t) - 3.1416)*(sin(th3(t) - 1.5708)*(sin(th2(t) - 1.5708)*(2.6536e-6*cos(th1(t)) + 1.0*sin(th1(t))) + 1.3268e-6*cos(th2(t) - 1.5708)*cos(th1(t))) - cos(th3(t) - 1.5708)*(1.0*cos(th2(t) - 1.5708)*(2.6536e-6*cos(th1(t)) + 1.0*sin(th1(t))) - 1.3268e-6*sin(th2(t) - 1.5708)*cos(th1(t)))) - 1.0*sin(th4(t) - 3.1416)*(cos(th3(t) - 1.5708)*(sin(th2(t) - 1.5708)*(2.6536e-6*cos(th1(t)) + 1.0*sin(th1(t))) + 1.3268e-6*cos(th2(t) - 1.5708)*cos(th1(t))) + 1.0*sin(th3(t) - 1.5708)*(1.0*cos(th2(t) - 1.5708)*(2.6536e-6*cos(th1(t)) + 1.0*sin(th1(t))) - 1.3268e-6*sin(th2(t) - 1.5708)*cos(th1(t))))))*(0.38*cos(th3(t))*(sin(th2(t) - 1.5708)*(2.6536e-6*cos(th1(t)) + 1.0*sin(th1(t))) + 1.3268e-6*cos(th2(t) - 1.5708)*cos(th1(t))) + 0.38*sin(th2(t))*(2.6536e-6*cos(th1(t)) + 1.0*sin(th1(t))) - 0.38*sin(th4(t))*(sin(th3(t) - 1.5708)*(sin(th2(t) - 1.5708)*(2.6536e-6*cos(th1(t)) + 1.0*sin(th1(t))) + 1.3268e-6*cos(th2(t) - 1.5708)*cos(th1(t))) - cos(th3(t) - 1.5708)*(1.0*cos(th2(t) - 1.5708)*(2.6536e-6*cos(th1(t)) + 1.0*sin(th1(t))) - 1.3268e-6*sin(th2(t) - 1.5708)*cos(th1(t)))) + 0.38*sin(th3(t))*(1.0*cos(th2(t) - 1.5708)*(2.6536e-6*cos(th1(t)) + 1.0*sin(th1(t))) - 1.3268e-6*sin(th2(t) - 1.5708)*cos(th1(t))) - 0.02*cos(th5(t))*(sin(th4(t) - 3.1416)*(sin(th3(t) - 1.5708)*(sin(th2(t) - 1.5708)*(2.6536e-6*cos(th1(t)) + 1.0*sin(th1(t))) + 1.3268e-6*cos(th2(t) - 1.5708)*cos(th1(t))) - cos(th3(t) - 1.5708)*(1.0*cos(th2(t) - 1.5708)*(2.6536e-6*cos(th1(t)) + 1.0*sin(th1(t))) - 1.3268e-6*sin(th2(t) - 1.5708)*cos(th1(t)))) + cos(th4(t) - 3.1416)*(cos(th3(t) - 1.5708)*(sin(th2(t) - 1.5708)*(2.6536e-6*cos(th1(t)) + 1.0*sin(th1(t))) + 1.3268e-6*cos(th2(t) - 1.5708)*cos(th1(t))) + 1.0*sin(th3(t) - 1.5708)*(1.0*cos(th2(t) - 1.5708)*(2.6536e-6*cos(th1(t)) + 1.0*sin(th1(t))) - 1.3268e-6*sin(th2(t) - 1.5708)*cos(th1(t))))) + 0.38*cos(th4(t))*(cos(th3(t) - 1.5708)*(sin(th2(t) - 1.5708)*(2.6536e-6*cos(th1(t)) + 1.0*sin(th1(t))) + 1.3268e-6*cos(th2(t) - 1.5708)*cos(th1(t))) + 1.0*sin(th3(t) - 1.5708)*(1.0*cos(th2(t) - 1.5708)*(2.6536e-6*cos(th1(t)) + 1.0*sin(th1(t))) - 1.3268e-6*sin(th2(t) - 1.5708)*cos(th1(t)))) + 0.02*sin(th5(t))*(cos(th4(t) - 3.1416)*(sin(th3(t) - 1.5708)*(sin(th2(t) - 1.5708)*(2.6536e-6*cos(th1(t)) + 1.0*sin(th1(t))) + 1.3268e-6*cos(th2(t) - 1.5708)*cos(th1(t))) - cos(th3(t) - 1.5708)*(1.0*cos(th2(t) - 1.5708)*(2.6536e-6*cos(th1(t)) + 1.0*sin(th1(t))) - 1.3268e-6*sin(th2(t) - 1.5708)*cos(th1(t)))) - 1.0*sin(th4(t) - 3.1416)*(cos(th3(t) - 1.5708)*(sin(th2(t) - 1.5708)*(2.6536e-6*cos(th1(t)) + 1.0*sin(th1(t))) + 1.3268e-6*cos(th2(t) - 1.5708)*cos(th1(t))) + 1.0*sin(th3(t) - 1.5708)*(1.0*cos(th2(t) - 1.5708)*(2.6536e-6*cos(th1(t)) + 1.0*sin(th1(t))) - 1.3268e-6*sin(th2(t) - 1.5708)*cos(th1(t))))) + 5.0418e-7*cos(th1(t))*cos(th2(t))) + 1.3806*(0.19*cos(th4(t))*(cos(th3(t) - 1.5708)*(sin(th2(t) - 1.5708)*(1.0*cos(th1(t)) - 2.6536e-6*sin(th1(t))) - 1.3268e-6*cos(th2(t) - 1.5708)*sin(th1(t))) + sin(th3(t) - 1.5708)*(cos(th2(t) - 1.5708)*(1.0*cos(th1(t)) - 2.6536e-6*sin(th1(t))) + 1.3268e-6*sin(th2(t) - 1.5708)*sin(th1(t)))) + 0.19*sin(th4(t))*(cos(th3(t) - 1.5708)*(cos(th2(t) - 1.5708)*(1.0*cos(th1(t)) - 2.6536e-6*sin(th1(t))) + 1.3268e-6*sin(th2(t) - 1.5708)*sin(th1(t))) - 1.0*sin(th3(t) - 1.5708)*(sin(th2(t) - 1.5708)*(1.0*cos(th1(t)) - 2.6536e-6*sin(th1(t))) - 1.3268e-6*cos(th2(t) - 1.5708)*sin(th1(t)))))*(0.19*cos(th4(t))*(cos(th3(t) - 1.5708)*(sin(th2(t) - 1.5708)*(1.0*cos(th1(t)) - 2.6536e-6*sin(th1(t))) - 1.3268e-6*cos(th2(t) - 1.5708)*sin(th1(t))) + sin(th3(t) - 1.5708)*(cos(th2(t) - 1.5708)*(1.0*cos(th1(t)) - 2.6536e-6*sin(th1(t))) + 1.3268e-6*sin(th2(t) - 1.5708)*sin(th1(t)))) - 5.0418e-7*cos(th2(t))*sin(th1(t)) + 0.38*cos(th3(t))*(sin(th2(t) - 1.5708)*(1.0*cos(th1(t)) - 2.6536e-6*sin(th1(t))) - 1.3268e-6*cos(th2(t) - 1.5708)*sin(th1(t))) + 0.38*sin(th2(t))*(1.0*cos(th1(t)) - 2.6536e-6*sin(th1(t))) + 0.38*sin(th3(t))*(cos(th2(t) - 1.5708)*(1.0*cos(th1(t)) - 2.6536e-6*sin(th1(t))) + 1.3268e-6*sin(th2(t) - 1.5708)*sin(th1(t))) + 0.19*sin(th4(t))*(cos(th3(t) - 1.5708)*(cos(th2(t) - 1.5708)*(1.0*cos(th1(t)) - 2.6536e-6*sin(th1(t))) + 1.3268e-6*sin(th2(t) - 1.5708)*sin(th1(t))) - 1.0*sin(th3(t) - 1.5708)*(sin(th2(t) - 1.5708)*(1.0*cos(th1(t)) - 2.6536e-6*sin(th1(t))) - 1.3268e-6*cos(th2(t) - 1.5708)*sin(th1(t))))) + 0.042427;
M25 = 0.13038*(0.02*sin(th5(t))*(cos(th4(t) - 3.1416)*(cos(th3(t) - 1.5708)*(3.5208e-12*cos(th2(t) - 1.5708) + 1.0*sin(th2(t) - 1.5708)) + sin(th3(t) - 1.5708)*(1.0*cos(th2(t) - 1.5708) - 3.5208e-12*sin(th2(t) - 1.5708))) - 1.0*sin(th4(t) - 3.1416)*(cos(th3(t) - 1.5708)*(1.0*cos(th2(t) - 1.5708) - 3.5208e-12*sin(th2(t) - 1.5708)) - 1.0*sin(th3(t) - 1.5708)*(3.5208e-12*cos(th2(t) - 1.5708) + 1.0*sin(th2(t) - 1.5708)))) - 0.02*cos(th5(t))*(sin(th4(t) - 3.1416)*(cos(th3(t) - 1.5708)*(3.5208e-12*cos(th2(t) - 1.5708) + 1.0*sin(th2(t) - 1.5708)) + sin(th3(t) - 1.5708)*(1.0*cos(th2(t) - 1.5708) - 3.5208e-12*sin(th2(t) - 1.5708))) + cos(th4(t) - 3.1416)*(cos(th3(t) - 1.5708)*(1.0*cos(th2(t) - 1.5708) - 3.5208e-12*sin(th2(t) - 1.5708)) - 1.0*sin(th3(t) - 1.5708)*(3.5208e-12*cos(th2(t) - 1.5708) + 1.0*sin(th2(t) - 1.5708)))))*(0.38*cos(th2(t)) - 1.3379e-12*sin(th2(t)) - 0.38*sin(th3(t))*(3.5208e-12*cos(th2(t) - 1.5708) + 1.0*sin(th2(t) - 1.5708)) + 0.02*sin(th5(t))*(cos(th4(t) - 3.1416)*(cos(th3(t) - 1.5708)*(3.5208e-12*cos(th2(t) - 1.5708) + 1.0*sin(th2(t) - 1.5708)) + sin(th3(t) - 1.5708)*(1.0*cos(th2(t) - 1.5708) - 3.5208e-12*sin(th2(t) - 1.5708))) - 1.0*sin(th4(t) - 3.1416)*(cos(th3(t) - 1.5708)*(1.0*cos(th2(t) - 1.5708) - 3.5208e-12*sin(th2(t) - 1.5708)) - 1.0*sin(th3(t) - 1.5708)*(3.5208e-12*cos(th2(t) - 1.5708) + 1.0*sin(th2(t) - 1.5708)))) - 0.38*sin(th4(t))*(cos(th3(t) - 1.5708)*(3.5208e-12*cos(th2(t) - 1.5708) + 1.0*sin(th2(t) - 1.5708)) + sin(th3(t) - 1.5708)*(1.0*cos(th2(t) - 1.5708) - 3.5208e-12*sin(th2(t) - 1.5708))) + 0.38*cos(th4(t))*(cos(th3(t) - 1.5708)*(1.0*cos(th2(t) - 1.5708) - 3.5208e-12*sin(th2(t) - 1.5708)) - 1.0*sin(th3(t) - 1.5708)*(3.5208e-12*cos(th2(t) - 1.5708) + 1.0*sin(th2(t) - 1.5708))) + 0.38*cos(th3(t))*(1.0*cos(th2(t) - 1.5708) - 3.5208e-12*sin(th2(t) - 1.5708)) - 0.02*cos(th5(t))*(sin(th4(t) - 3.1416)*(cos(th3(t) - 1.5708)*(3.5208e-12*cos(th2(t) - 1.5708) + 1.0*sin(th2(t) - 1.5708)) + sin(th3(t) - 1.5708)*(1.0*cos(th2(t) - 1.5708) - 3.5208e-12*sin(th2(t) - 1.5708))) + cos(th4(t) - 3.1416)*(cos(th3(t) - 1.5708)*(1.0*cos(th2(t) - 1.5708) - 3.5208e-12*sin(th2(t) - 1.5708)) - 1.0*sin(th3(t) - 1.5708)*(3.5208e-12*cos(th2(t) - 1.5708) + 1.0*sin(th2(t) - 1.5708))))) - 0.13038*(0.02*sin(th5(t))*(sin(th4(t) - 3.1416)*(cos(th3(t) - 1.5708)*(sin(th2(t) - 1.5708)*(1.0*cos(th1(t)) - 2.6536e-6*sin(th1(t))) - 1.3268e-6*cos(th2(t) - 1.5708)*sin(th1(t))) + sin(th3(t) - 1.5708)*(cos(th2(t) - 1.5708)*(1.0*cos(th1(t)) - 2.6536e-6*sin(th1(t))) + 1.3268e-6*sin(th2(t) - 1.5708)*sin(th1(t)))) + cos(th4(t) - 3.1416)*(cos(th3(t) - 1.5708)*(cos(th2(t) - 1.5708)*(1.0*cos(th1(t)) - 2.6536e-6*sin(th1(t))) + 1.3268e-6*sin(th2(t) - 1.5708)*sin(th1(t))) - 1.0*sin(th3(t) - 1.5708)*(sin(th2(t) - 1.5708)*(1.0*cos(th1(t)) - 2.6536e-6*sin(th1(t))) - 1.3268e-6*cos(th2(t) - 1.5708)*sin(th1(t))))) + 0.02*cos(th5(t))*(cos(th4(t) - 3.1416)*(cos(th3(t) - 1.5708)*(sin(th2(t) - 1.5708)*(1.0*cos(th1(t)) - 2.6536e-6*sin(th1(t))) - 1.3268e-6*cos(th2(t) - 1.5708)*sin(th1(t))) + sin(th3(t) - 1.5708)*(cos(th2(t) - 1.5708)*(1.0*cos(th1(t)) - 2.6536e-6*sin(th1(t))) + 1.3268e-6*sin(th2(t) - 1.5708)*sin(th1(t)))) - 1.0*sin(th4(t) - 3.1416)*(cos(th3(t) - 1.5708)*(cos(th2(t) - 1.5708)*(1.0*cos(th1(t)) - 2.6536e-6*sin(th1(t))) + 1.3268e-6*sin(th2(t) - 1.5708)*sin(th1(t))) - 1.0*sin(th3(t) - 1.5708)*(sin(th2(t) - 1.5708)*(1.0*cos(th1(t)) - 2.6536e-6*sin(th1(t))) - 1.3268e-6*cos(th2(t) - 1.5708)*sin(th1(t))))))*(0.38*cos(th4(t))*(cos(th3(t) - 1.5708)*(sin(th2(t) - 1.5708)*(1.0*cos(th1(t)) - 2.6536e-6*sin(th1(t))) - 1.3268e-6*cos(th2(t) - 1.5708)*sin(th1(t))) + sin(th3(t) - 1.5708)*(cos(th2(t) - 1.5708)*(1.0*cos(th1(t)) - 2.6536e-6*sin(th1(t))) + 1.3268e-6*sin(th2(t) - 1.5708)*sin(th1(t)))) - 5.0418e-7*cos(th2(t))*sin(th1(t)) + 0.38*cos(th3(t))*(sin(th2(t) - 1.5708)*(1.0*cos(th1(t)) - 2.6536e-6*sin(th1(t))) - 1.3268e-6*cos(th2(t) - 1.5708)*sin(th1(t))) + 0.38*sin(th2(t))*(1.0*cos(th1(t)) - 2.6536e-6*sin(th1(t))) + 0.38*sin(th3(t))*(cos(th2(t) - 1.5708)*(1.0*cos(th1(t)) - 2.6536e-6*sin(th1(t))) + 1.3268e-6*sin(th2(t) - 1.5708)*sin(th1(t))) - 0.02*sin(th5(t))*(sin(th4(t) - 3.1416)*(cos(th3(t) - 1.5708)*(sin(th2(t) - 1.5708)*(1.0*cos(th1(t)) - 2.6536e-6*sin(th1(t))) - 1.3268e-6*cos(th2(t) - 1.5708)*sin(th1(t))) + sin(th3(t) - 1.5708)*(cos(th2(t) - 1.5708)*(1.0*cos(th1(t)) - 2.6536e-6*sin(th1(t))) + 1.3268e-6*sin(th2(t) - 1.5708)*sin(th1(t)))) + cos(th4(t) - 3.1416)*(cos(th3(t) - 1.5708)*(cos(th2(t) - 1.5708)*(1.0*cos(th1(t)) - 2.6536e-6*sin(th1(t))) + 1.3268e-6*sin(th2(t) - 1.5708)*sin(th1(t))) - 1.0*sin(th3(t) - 1.5708)*(sin(th2(t) - 1.5708)*(1.0*cos(th1(t)) - 2.6536e-6*sin(th1(t))) - 1.3268e-6*cos(th2(t) - 1.5708)*sin(th1(t))))) + 0.38*sin(th4(t))*(cos(th3(t) - 1.5708)*(cos(th2(t) - 1.5708)*(1.0*cos(th1(t)) - 2.6536e-6*sin(th1(t))) + 1.3268e-6*sin(th2(t) - 1.5708)*sin(th1(t))) - 1.0*sin(th3(t) - 1.5708)*(sin(th2(t) - 1.5708)*(1.0*cos(th1(t)) - 2.6536e-6*sin(th1(t))) - 1.3268e-6*cos(th2(t) - 1.5708)*sin(th1(t)))) - 0.02*cos(th5(t))*(cos(th4(t) - 3.1416)*(cos(th3(t) - 1.5708)*(sin(th2(t) - 1.5708)*(1.0*cos(th1(t)) - 2.6536e-6*sin(th1(t))) - 1.3268e-6*cos(th2(t) - 1.5708)*sin(th1(t))) + sin(th3(t) - 1.5708)*(cos(th2(t) - 1.5708)*(1.0*cos(th1(t)) - 2.6536e-6*sin(th1(t))) + 1.3268e-6*sin(th2(t) - 1.5708)*sin(th1(t)))) - 1.0*sin(th4(t) - 3.1416)*(cos(th3(t) - 1.5708)*(cos(th2(t) - 1.5708)*(1.0*cos(th1(t)) - 2.6536e-6*sin(th1(t))) + 1.3268e-6*sin(th2(t) - 1.5708)*sin(th1(t))) - 1.0*sin(th3(t) - 1.5708)*(sin(th2(t) - 1.5708)*(1.0*cos(th1(t)) - 2.6536e-6*sin(th1(t))) - 1.3268e-6*cos(th2(t) - 1.5708)*sin(th1(t)))))) - 0.13038*(0.02*cos(th5(t))*(sin(th4(t) - 3.1416)*(sin(th3(t) - 1.5708)*(sin(th2(t) - 1.5708)*(2.6536e-6*cos(th1(t)) + 1.0*sin(th1(t))) + 1.3268e-6*cos(th2(t) - 1.5708)*cos(th1(t))) - cos(th3(t) - 1.5708)*(1.0*cos(th2(t) - 1.5708)*(2.6536e-6*cos(th1(t)) + 1.0*sin(th1(t))) - 1.3268e-6*sin(th2(t) - 1.5708)*cos(th1(t)))) + cos(th4(t) - 3.1416)*(cos(th3(t) - 1.5708)*(sin(th2(t) - 1.5708)*(2.6536e-6*cos(th1(t)) + 1.0*sin(th1(t))) + 1.3268e-6*cos(th2(t) - 1.5708)*cos(th1(t))) + 1.0*sin(th3(t) - 1.5708)*(1.0*cos(th2(t) - 1.5708)*(2.6536e-6*cos(th1(t)) + 1.0*sin(th1(t))) - 1.3268e-6*sin(th2(t) - 1.5708)*cos(th1(t))))) - 0.02*sin(th5(t))*(cos(th4(t) - 3.1416)*(sin(th3(t) - 1.5708)*(sin(th2(t) - 1.5708)*(2.6536e-6*cos(th1(t)) + 1.0*sin(th1(t))) + 1.3268e-6*cos(th2(t) - 1.5708)*cos(th1(t))) - cos(th3(t) - 1.5708)*(1.0*cos(th2(t) - 1.5708)*(2.6536e-6*cos(th1(t)) + 1.0*sin(th1(t))) - 1.3268e-6*sin(th2(t) - 1.5708)*cos(th1(t)))) - 1.0*sin(th4(t) - 3.1416)*(cos(th3(t) - 1.5708)*(sin(th2(t) - 1.5708)*(2.6536e-6*cos(th1(t)) + 1.0*sin(th1(t))) + 1.3268e-6*cos(th2(t) - 1.5708)*cos(th1(t))) + 1.0*sin(th3(t) - 1.5708)*(1.0*cos(th2(t) - 1.5708)*(2.6536e-6*cos(th1(t)) + 1.0*sin(th1(t))) - 1.3268e-6*sin(th2(t) - 1.5708)*cos(th1(t))))))*(0.38*cos(th3(t))*(sin(th2(t) - 1.5708)*(2.6536e-6*cos(th1(t)) + 1.0*sin(th1(t))) + 1.3268e-6*cos(th2(t) - 1.5708)*cos(th1(t))) + 0.38*sin(th2(t))*(2.6536e-6*cos(th1(t)) + 1.0*sin(th1(t))) - 0.38*sin(th4(t))*(sin(th3(t) - 1.5708)*(sin(th2(t) - 1.5708)*(2.6536e-6*cos(th1(t)) + 1.0*sin(th1(t))) + 1.3268e-6*cos(th2(t) - 1.5708)*cos(th1(t))) - cos(th3(t) - 1.5708)*(1.0*cos(th2(t) - 1.5708)*(2.6536e-6*cos(th1(t)) + 1.0*sin(th1(t))) - 1.3268e-6*sin(th2(t) - 1.5708)*cos(th1(t)))) + 0.38*sin(th3(t))*(1.0*cos(th2(t) - 1.5708)*(2.6536e-6*cos(th1(t)) + 1.0*sin(th1(t))) - 1.3268e-6*sin(th2(t) - 1.5708)*cos(th1(t))) - 0.02*cos(th5(t))*(sin(th4(t) - 3.1416)*(sin(th3(t) - 1.5708)*(sin(th2(t) - 1.5708)*(2.6536e-6*cos(th1(t)) + 1.0*sin(th1(t))) + 1.3268e-6*cos(th2(t) - 1.5708)*cos(th1(t))) - cos(th3(t) - 1.5708)*(1.0*cos(th2(t) - 1.5708)*(2.6536e-6*cos(th1(t)) + 1.0*sin(th1(t))) - 1.3268e-6*sin(th2(t) - 1.5708)*cos(th1(t)))) + cos(th4(t) - 3.1416)*(cos(th3(t) - 1.5708)*(sin(th2(t) - 1.5708)*(2.6536e-6*cos(th1(t)) + 1.0*sin(th1(t))) + 1.3268e-6*cos(th2(t) - 1.5708)*cos(th1(t))) + 1.0*sin(th3(t) - 1.5708)*(1.0*cos(th2(t) - 1.5708)*(2.6536e-6*cos(th1(t)) + 1.0*sin(th1(t))) - 1.3268e-6*sin(th2(t) - 1.5708)*cos(th1(t))))) + 0.38*cos(th4(t))*(cos(th3(t) - 1.5708)*(sin(th2(t) - 1.5708)*(2.6536e-6*cos(th1(t)) + 1.0*sin(th1(t))) + 1.3268e-6*cos(th2(t) - 1.5708)*cos(th1(t))) + 1.0*sin(th3(t) - 1.5708)*(1.0*cos(th2(t) - 1.5708)*(2.6536e-6*cos(th1(t)) + 1.0*sin(th1(t))) - 1.3268e-6*sin(th2(t) - 1.5708)*cos(th1(t)))) + 0.02*sin(th5(t))*(cos(th4(t) - 3.1416)*(sin(th3(t) - 1.5708)*(sin(th2(t) - 1.5708)*(2.6536e-6*cos(th1(t)) + 1.0*sin(th1(t))) + 1.3268e-6*cos(th2(t) - 1.5708)*cos(th1(t))) - cos(th3(t) - 1.5708)*(1.0*cos(th2(t) - 1.5708)*(2.6536e-6*cos(th1(t)) + 1.0*sin(th1(t))) - 1.3268e-6*sin(th2(t) - 1.5708)*cos(th1(t)))) - 1.0*sin(th4(t) - 3.1416)*(cos(th3(t) - 1.5708)*(sin(th2(t) - 1.5708)*(2.6536e-6*cos(th1(t)) + 1.0*sin(th1(t))) + 1.3268e-6*cos(th2(t) - 1.5708)*cos(th1(t))) + 1.0*sin(th3(t) - 1.5708)*(1.0*cos(th2(t) - 1.5708)*(2.6536e-6*cos(th1(t)) + 1.0*sin(th1(t))) - 1.3268e-6*sin(th2(t) - 1.5708)*cos(th1(t))))) + 5.0418e-7*cos(th1(t))*cos(th2(t))) + 0.00018665;

M31 = 0.051004 - 1.3806*(0.38*cos(th3(t))*(sin(th2(t) - 1.5708)*(2.6536e-6*cos(th1(t)) + 1.0*sin(th1(t))) + 1.3268e-6*cos(th2(t) - 1.5708)*cos(th1(t))) - 0.19*sin(th4(t))*(sin(th3(t) - 1.5708)*(sin(th2(t) - 1.5708)*(2.6536e-6*cos(th1(t)) + 1.0*sin(th1(t))) + 1.3268e-6*cos(th2(t) - 1.5708)*cos(th1(t))) - cos(th3(t) - 1.5708)*(1.0*cos(th2(t) - 1.5708)*(2.6536e-6*cos(th1(t)) + 1.0*sin(th1(t))) - 1.3268e-6*sin(th2(t) - 1.5708)*cos(th1(t)))) + 0.38*sin(th3(t))*(1.0*cos(th2(t) - 1.5708)*(2.6536e-6*cos(th1(t)) + 1.0*sin(th1(t))) - 1.3268e-6*sin(th2(t) - 1.5708)*cos(th1(t))) + 0.19*cos(th4(t))*(cos(th3(t) - 1.5708)*(sin(th2(t) - 1.5708)*(2.6536e-6*cos(th1(t)) + 1.0*sin(th1(t))) + 1.3268e-6*cos(th2(t) - 1.5708)*cos(th1(t))) + 1.0*sin(th3(t) - 1.5708)*(1.0*cos(th2(t) - 1.5708)*(2.6536e-6*cos(th1(t)) + 1.0*sin(th1(t))) - 1.3268e-6*sin(th2(t) - 1.5708)*cos(th1(t)))))*(5.0418e-7*sin(th1(t))*sin(th2(t)) + 0.38*cos(th2(t))*(1.0*cos(th1(t)) - 2.6536e-6*sin(th1(t))) + 0.38*cos(th3(t))*(cos(th2(t) - 1.5708)*(1.0*cos(th1(t)) - 2.6536e-6*sin(th1(t))) + 1.3268e-6*sin(th2(t) - 1.5708)*sin(th1(t))) + 0.19*cos(th4(t))*(cos(th3(t) - 1.5708)*(cos(th2(t) - 1.5708)*(1.0*cos(th1(t)) - 2.6536e-6*sin(th1(t))) + 1.3268e-6*sin(th2(t) - 1.5708)*sin(th1(t))) - sin(th3(t) - 1.5708)*(1.0*sin(th2(t) - 1.5708)*(1.0*cos(th1(t)) - 2.6536e-6*sin(th1(t))) - 1.3268e-6*cos(th2(t) - 1.5708)*sin(th1(t)))) - 0.38*sin(th3(t))*(1.0*sin(th2(t) - 1.5708)*(1.0*cos(th1(t)) - 2.6536e-6*sin(th1(t))) - 1.3268e-6*cos(th2(t) - 1.5708)*sin(th1(t))) - 0.19*sin(th4(t))*(1.0*sin(th3(t) - 1.5708)*(cos(th2(t) - 1.5708)*(1.0*cos(th1(t)) - 2.6536e-6*sin(th1(t))) + 1.3268e-6*sin(th2(t) - 1.5708)*sin(th1(t))) + cos(th3(t) - 1.5708)*(1.0*sin(th2(t) - 1.5708)*(1.0*cos(th1(t)) - 2.6536e-6*sin(th1(t))) - 1.3268e-6*cos(th2(t) - 1.5708)*sin(th1(t))))) - 0.49277*(0.19*cos(th3(t))*(sin(th2(t) - 1.5708)*(2.6536e-6*cos(th1(t)) + 1.0*sin(th1(t))) + 1.3268e-6*cos(th2(t) - 1.5708)*cos(th1(t))) + 0.19*sin(th3(t))*(1.0*cos(th2(t) - 1.5708)*(2.6536e-6*cos(th1(t)) + 1.0*sin(th1(t))) - 1.3268e-6*sin(th2(t) - 1.5708)*cos(th1(t))))*(5.0418e-7*sin(th1(t))*sin(th2(t)) + 0.38*cos(th2(t))*(1.0*cos(th1(t)) - 2.6536e-6*sin(th1(t))) + 0.19*cos(th3(t))*(cos(th2(t) - 1.5708)*(1.0*cos(th1(t)) - 2.6536e-6*sin(th1(t))) + 1.3268e-6*sin(th2(t) - 1.5708)*sin(th1(t))) - 0.19*sin(th3(t))*(1.0*sin(th2(t) - 1.5708)*(1.0*cos(th1(t)) - 2.6536e-6*sin(th1(t))) - 1.3268e-6*cos(th2(t) - 1.5708)*sin(th1(t)))) - 0.13038*(0.38*cos(th4(t))*(cos(th3(t) - 1.5708)*(sin(th2(t) - 1.5708)*(1.0*cos(th1(t)) - 2.6536e-6*sin(th1(t))) - 1.3268e-6*cos(th2(t) - 1.5708)*sin(th1(t))) + sin(th3(t) - 1.5708)*(cos(th2(t) - 1.5708)*(1.0*cos(th1(t)) - 2.6536e-6*sin(th1(t))) + 1.3268e-6*sin(th2(t) - 1.5708)*sin(th1(t)))) + 0.38*cos(th3(t))*(sin(th2(t) - 1.5708)*(1.0*cos(th1(t)) - 2.6536e-6*sin(th1(t))) - 1.3268e-6*cos(th2(t) - 1.5708)*sin(th1(t))) + 0.38*sin(th3(t))*(cos(th2(t) - 1.5708)*(1.0*cos(th1(t)) - 2.6536e-6*sin(th1(t))) + 1.3268e-6*sin(th2(t) - 1.5708)*sin(th1(t))) - 0.02*sin(th5(t))*(sin(th4(t) - 3.1416)*(cos(th3(t) - 1.5708)*(sin(th2(t) - 1.5708)*(1.0*cos(th1(t)) - 2.6536e-6*sin(th1(t))) - 1.3268e-6*cos(th2(t) - 1.5708)*sin(th1(t))) + sin(th3(t) - 1.5708)*(cos(th2(t) - 1.5708)*(1.0*cos(th1(t)) - 2.6536e-6*sin(th1(t))) + 1.3268e-6*sin(th2(t) - 1.5708)*sin(th1(t)))) + cos(th4(t) - 3.1416)*(cos(th3(t) - 1.5708)*(cos(th2(t) - 1.5708)*(1.0*cos(th1(t)) - 2.6536e-6*sin(th1(t))) + 1.3268e-6*sin(th2(t) - 1.5708)*sin(th1(t))) - 1.0*sin(th3(t) - 1.5708)*(sin(th2(t) - 1.5708)*(1.0*cos(th1(t)) - 2.6536e-6*sin(th1(t))) - 1.3268e-6*cos(th2(t) - 1.5708)*sin(th1(t))))) + 0.38*sin(th4(t))*(cos(th3(t) - 1.5708)*(cos(th2(t) - 1.5708)*(1.0*cos(th1(t)) - 2.6536e-6*sin(th1(t))) + 1.3268e-6*sin(th2(t) - 1.5708)*sin(th1(t))) - 1.0*sin(th3(t) - 1.5708)*(sin(th2(t) - 1.5708)*(1.0*cos(th1(t)) - 2.6536e-6*sin(th1(t))) - 1.3268e-6*cos(th2(t) - 1.5708)*sin(th1(t)))) - 0.02*cos(th5(t))*(cos(th4(t) - 3.1416)*(cos(th3(t) - 1.5708)*(sin(th2(t) - 1.5708)*(1.0*cos(th1(t)) - 2.6536e-6*sin(th1(t))) - 1.3268e-6*cos(th2(t) - 1.5708)*sin(th1(t))) + sin(th3(t) - 1.5708)*(cos(th2(t) - 1.5708)*(1.0*cos(th1(t)) - 2.6536e-6*sin(th1(t))) + 1.3268e-6*sin(th2(t) - 1.5708)*sin(th1(t)))) - 1.0*sin(th4(t) - 3.1416)*(cos(th3(t) - 1.5708)*(cos(th2(t) - 1.5708)*(1.0*cos(th1(t)) - 2.6536e-6*sin(th1(t))) + 1.3268e-6*sin(th2(t) - 1.5708)*sin(th1(t))) - 1.0*sin(th3(t) - 1.5708)*(sin(th2(t) - 1.5708)*(1.0*cos(th1(t)) - 2.6536e-6*sin(th1(t))) - 1.3268e-6*cos(th2(t) - 1.5708)*sin(th1(t))))))*(5.0418e-7*cos(th1(t))*sin(th2(t)) + 0.02*cos(th5(t))*(cos(th4(t) - 3.1416)*(cos(th3(t) - 1.5708)*(cos(th2(t) - 1.5708)*(2.6536e-6*cos(th1(t)) + 1.0*sin(th1(t))) - 1.3268e-6*sin(th2(t) - 1.5708)*cos(th1(t))) - 1.0*sin(th3(t) - 1.5708)*(sin(th2(t) - 1.5708)*(2.6536e-6*cos(th1(t)) + 1.0*sin(th1(t))) + 1.3268e-6*cos(th2(t) - 1.5708)*cos(th1(t)))) + sin(th4(t) - 3.1416)*(cos(th3(t) - 1.5708)*(sin(th2(t) - 1.5708)*(2.6536e-6*cos(th1(t)) + 1.0*sin(th1(t))) + 1.3268e-6*cos(th2(t) - 1.5708)*cos(th1(t))) + sin(th3(t) - 1.5708)*(cos(th2(t) - 1.5708)*(2.6536e-6*cos(th1(t)) + 1.0*sin(th1(t))) - 1.3268e-6*sin(th2(t) - 1.5708)*cos(th1(t))))) + 0.38*sin(th4(t))*(cos(th3(t) - 1.5708)*(sin(th2(t) - 1.5708)*(2.6536e-6*cos(th1(t)) + 1.0*sin(th1(t))) + 1.3268e-6*cos(th2(t) - 1.5708)*cos(th1(t))) + sin(th3(t) - 1.5708)*(cos(th2(t) - 1.5708)*(2.6536e-6*cos(th1(t)) + 1.0*sin(th1(t))) - 1.3268e-6*sin(th2(t) - 1.5708)*cos(th1(t)))) - 0.38*cos(th3(t))*(cos(th2(t) - 1.5708)*(2.6536e-6*cos(th1(t)) + 1.0*sin(th1(t))) - 1.3268e-6*sin(th2(t) - 1.5708)*cos(th1(t))) - 0.38*cos(th2(t))*(2.6536e-6*cos(th1(t)) + 1.0*sin(th1(t))) + 0.38*sin(th3(t))*(sin(th2(t) - 1.5708)*(2.6536e-6*cos(th1(t)) + 1.0*sin(th1(t))) + 1.3268e-6*cos(th2(t) - 1.5708)*cos(th1(t))) - 0.38*cos(th4(t))*(cos(th3(t) - 1.5708)*(cos(th2(t) - 1.5708)*(2.6536e-6*cos(th1(t)) + 1.0*sin(th1(t))) - 1.3268e-6*sin(th2(t) - 1.5708)*cos(th1(t))) - 1.0*sin(th3(t) - 1.5708)*(sin(th2(t) - 1.5708)*(2.6536e-6*cos(th1(t)) + 1.0*sin(th1(t))) + 1.3268e-6*cos(th2(t) - 1.5708)*cos(th1(t)))) + 0.02*sin(th5(t))*(1.0*sin(th4(t) - 3.1416)*(cos(th3(t) - 1.5708)*(cos(th2(t) - 1.5708)*(2.6536e-6*cos(th1(t)) + 1.0*sin(th1(t))) - 1.3268e-6*sin(th2(t) - 1.5708)*cos(th1(t))) - 1.0*sin(th3(t) - 1.5708)*(sin(th2(t) - 1.5708)*(2.6536e-6*cos(th1(t)) + 1.0*sin(th1(t))) + 1.3268e-6*cos(th2(t) - 1.5708)*cos(th1(t)))) - cos(th4(t) - 3.1416)*(cos(th3(t) - 1.5708)*(sin(th2(t) - 1.5708)*(2.6536e-6*cos(th1(t)) + 1.0*sin(th1(t))) + 1.3268e-6*cos(th2(t) - 1.5708)*cos(th1(t))) + sin(th3(t) - 1.5708)*(cos(th2(t) - 1.5708)*(2.6536e-6*cos(th1(t)) + 1.0*sin(th1(t))) - 1.3268e-6*sin(th2(t) - 1.5708)*cos(th1(t)))))) - 1.3806*(0.19*cos(th4(t))*(cos(th3(t) - 1.5708)*(sin(th2(t) - 1.5708)*(1.0*cos(th1(t)) - 2.6536e-6*sin(th1(t))) - 1.3268e-6*cos(th2(t) - 1.5708)*sin(th1(t))) + sin(th3(t) - 1.5708)*(cos(th2(t) - 1.5708)*(1.0*cos(th1(t)) - 2.6536e-6*sin(th1(t))) + 1.3268e-6*sin(th2(t) - 1.5708)*sin(th1(t)))) + 0.38*cos(th3(t))*(sin(th2(t) - 1.5708)*(1.0*cos(th1(t)) - 2.6536e-6*sin(th1(t))) - 1.3268e-6*cos(th2(t) - 1.5708)*sin(th1(t))) + 0.38*sin(th3(t))*(cos(th2(t) - 1.5708)*(1.0*cos(th1(t)) - 2.6536e-6*sin(th1(t))) + 1.3268e-6*sin(th2(t) - 1.5708)*sin(th1(t))) + 0.19*sin(th4(t))*(cos(th3(t) - 1.5708)*(cos(th2(t) - 1.5708)*(1.0*cos(th1(t)) - 2.6536e-6*sin(th1(t))) + 1.3268e-6*sin(th2(t) - 1.5708)*sin(th1(t))) - 1.0*sin(th3(t) - 1.5708)*(sin(th2(t) - 1.5708)*(1.0*cos(th1(t)) - 2.6536e-6*sin(th1(t))) - 1.3268e-6*cos(th2(t) - 1.5708)*sin(th1(t)))))*(5.0418e-7*cos(th1(t))*sin(th2(t)) + 0.19*sin(th4(t))*(cos(th3(t) - 1.5708)*(sin(th2(t) - 1.5708)*(2.6536e-6*cos(th1(t)) + 1.0*sin(th1(t))) + 1.3268e-6*cos(th2(t) - 1.5708)*cos(th1(t))) + sin(th3(t) - 1.5708)*(cos(th2(t) - 1.5708)*(2.6536e-6*cos(th1(t)) + 1.0*sin(th1(t))) - 1.3268e-6*sin(th2(t) - 1.5708)*cos(th1(t)))) - 0.38*cos(th3(t))*(cos(th2(t) - 1.5708)*(2.6536e-6*cos(th1(t)) + 1.0*sin(th1(t))) - 1.3268e-6*sin(th2(t) - 1.5708)*cos(th1(t))) - 0.38*cos(th2(t))*(2.6536e-6*cos(th1(t)) + 1.0*sin(th1(t))) + 0.38*sin(th3(t))*(sin(th2(t) - 1.5708)*(2.6536e-6*cos(th1(t)) + 1.0*sin(th1(t))) + 1.3268e-6*cos(th2(t) - 1.5708)*cos(th1(t))) - 0.19*cos(th4(t))*(cos(th3(t) - 1.5708)*(cos(th2(t) - 1.5708)*(2.6536e-6*cos(th1(t)) + 1.0*sin(th1(t))) - 1.3268e-6*sin(th2(t) - 1.5708)*cos(th1(t))) - 1.0*sin(th3(t) - 1.5708)*(sin(th2(t) - 1.5708)*(2.6536e-6*cos(th1(t)) + 1.0*sin(th1(t))) + 1.3268e-6*cos(th2(t) - 1.5708)*cos(th1(t))))) - 0.49277*(0.19*cos(th3(t))*(sin(th2(t) - 1.5708)*(1.0*cos(th1(t)) - 2.6536e-6*sin(th1(t))) - 1.3268e-6*cos(th2(t) - 1.5708)*sin(th1(t))) + 0.19*sin(th3(t))*(cos(th2(t) - 1.5708)*(1.0*cos(th1(t)) - 2.6536e-6*sin(th1(t))) + 1.3268e-6*sin(th2(t) - 1.5708)*sin(th1(t))))*(5.0418e-7*cos(th1(t))*sin(th2(t)) - 0.19*cos(th3(t))*(cos(th2(t) - 1.5708)*(2.6536e-6*cos(th1(t)) + 1.0*sin(th1(t))) - 1.3268e-6*sin(th2(t) - 1.5708)*cos(th1(t))) - 0.38*cos(th2(t))*(2.6536e-6*cos(th1(t)) + 1.0*sin(th1(t))) + 0.19*sin(th3(t))*(sin(th2(t) - 1.5708)*(2.6536e-6*cos(th1(t)) + 1.0*sin(th1(t))) + 1.3268e-6*cos(th2(t) - 1.5708)*cos(th1(t)))) - 0.13038*(0.38*cos(th3(t))*(sin(th2(t) - 1.5708)*(2.6536e-6*cos(th1(t)) + 1.0*sin(th1(t))) + 1.3268e-6*cos(th2(t) - 1.5708)*cos(th1(t))) - 0.38*sin(th4(t))*(sin(th3(t) - 1.5708)*(sin(th2(t) - 1.5708)*(2.6536e-6*cos(th1(t)) + 1.0*sin(th1(t))) + 1.3268e-6*cos(th2(t) - 1.5708)*cos(th1(t))) - cos(th3(t) - 1.5708)*(1.0*cos(th2(t) - 1.5708)*(2.6536e-6*cos(th1(t)) + 1.0*sin(th1(t))) - 1.3268e-6*sin(th2(t) - 1.5708)*cos(th1(t)))) + 0.38*sin(th3(t))*(1.0*cos(th2(t) - 1.5708)*(2.6536e-6*cos(th1(t)) + 1.0*sin(th1(t))) - 1.3268e-6*sin(th2(t) - 1.5708)*cos(th1(t))) - 0.02*cos(th5(t))*(sin(th4(t) - 3.1416)*(sin(th3(t) - 1.5708)*(sin(th2(t) - 1.5708)*(2.6536e-6*cos(th1(t)) + 1.0*sin(th1(t))) + 1.3268e-6*cos(th2(t) - 1.5708)*cos(th1(t))) - cos(th3(t) - 1.5708)*(1.0*cos(th2(t) - 1.5708)*(2.6536e-6*cos(th1(t)) + 1.0*sin(th1(t))) - 1.3268e-6*sin(th2(t) - 1.5708)*cos(th1(t)))) + cos(th4(t) - 3.1416)*(cos(th3(t) - 1.5708)*(sin(th2(t) - 1.5708)*(2.6536e-6*cos(th1(t)) + 1.0*sin(th1(t))) + 1.3268e-6*cos(th2(t) - 1.5708)*cos(th1(t))) + 1.0*sin(th3(t) - 1.5708)*(1.0*cos(th2(t) - 1.5708)*(2.6536e-6*cos(th1(t)) + 1.0*sin(th1(t))) - 1.3268e-6*sin(th2(t) - 1.5708)*cos(th1(t))))) + 0.38*cos(th4(t))*(cos(th3(t) - 1.5708)*(sin(th2(t) - 1.5708)*(2.6536e-6*cos(th1(t)) + 1.0*sin(th1(t))) + 1.3268e-6*cos(th2(t) - 1.5708)*cos(th1(t))) + 1.0*sin(th3(t) - 1.5708)*(1.0*cos(th2(t) - 1.5708)*(2.6536e-6*cos(th1(t)) + 1.0*sin(th1(t))) - 1.3268e-6*sin(th2(t) - 1.5708)*cos(th1(t)))) + 0.02*sin(th5(t))*(cos(th4(t) - 3.1416)*(sin(th3(t) - 1.5708)*(sin(th2(t) - 1.5708)*(2.6536e-6*cos(th1(t)) + 1.0*sin(th1(t))) + 1.3268e-6*cos(th2(t) - 1.5708)*cos(th1(t))) - cos(th3(t) - 1.5708)*(1.0*cos(th2(t) - 1.5708)*(2.6536e-6*cos(th1(t)) + 1.0*sin(th1(t))) - 1.3268e-6*sin(th2(t) - 1.5708)*cos(th1(t)))) - 1.0*sin(th4(t) - 3.1416)*(cos(th3(t) - 1.5708)*(sin(th2(t) - 1.5708)*(2.6536e-6*cos(th1(t)) + 1.0*sin(th1(t))) + 1.3268e-6*cos(th2(t) - 1.5708)*cos(th1(t))) + 1.0*sin(th3(t) - 1.5708)*(1.0*cos(th2(t) - 1.5708)*(2.6536e-6*cos(th1(t)) + 1.0*sin(th1(t))) - 1.3268e-6*sin(th2(t) - 1.5708)*cos(th1(t))))))*(5.0418e-7*sin(th1(t))*sin(th2(t)) - 0.02*cos(th5(t))*(cos(th4(t) - 3.1416)*(cos(th3(t) - 1.5708)*(cos(th2(t) - 1.5708)*(1.0*cos(th1(t)) - 2.6536e-6*sin(th1(t))) + 1.3268e-6*sin(th2(t) - 1.5708)*sin(th1(t))) - sin(th3(t) - 1.5708)*(1.0*sin(th2(t) - 1.5708)*(1.0*cos(th1(t)) - 2.6536e-6*sin(th1(t))) - 1.3268e-6*cos(th2(t) - 1.5708)*sin(th1(t)))) + 1.0*sin(th4(t) - 3.1416)*(1.0*sin(th3(t) - 1.5708)*(cos(th2(t) - 1.5708)*(1.0*cos(th1(t)) - 2.6536e-6*sin(th1(t))) + 1.3268e-6*sin(th2(t) - 1.5708)*sin(th1(t))) + cos(th3(t) - 1.5708)*(1.0*sin(th2(t) - 1.5708)*(1.0*cos(th1(t)) - 2.6536e-6*sin(th1(t))) - 1.3268e-6*cos(th2(t) - 1.5708)*sin(th1(t))))) + 0.38*cos(th2(t))*(1.0*cos(th1(t)) - 2.6536e-6*sin(th1(t))) + 0.38*cos(th3(t))*(cos(th2(t) - 1.5708)*(1.0*cos(th1(t)) - 2.6536e-6*sin(th1(t))) + 1.3268e-6*sin(th2(t) - 1.5708)*sin(th1(t))) + 0.38*cos(th4(t))*(cos(th3(t) - 1.5708)*(cos(th2(t) - 1.5708)*(1.0*cos(th1(t)) - 2.6536e-6*sin(th1(t))) + 1.3268e-6*sin(th2(t) - 1.5708)*sin(th1(t))) - sin(th3(t) - 1.5708)*(1.0*sin(th2(t) - 1.5708)*(1.0*cos(th1(t)) - 2.6536e-6*sin(th1(t))) - 1.3268e-6*cos(th2(t) - 1.5708)*sin(th1(t)))) - 0.38*sin(th3(t))*(1.0*sin(th2(t) - 1.5708)*(1.0*cos(th1(t)) - 2.6536e-6*sin(th1(t))) - 1.3268e-6*cos(th2(t) - 1.5708)*sin(th1(t))) - 0.38*sin(th4(t))*(1.0*sin(th3(t) - 1.5708)*(cos(th2(t) - 1.5708)*(1.0*cos(th1(t)) - 2.6536e-6*sin(th1(t))) + 1.3268e-6*sin(th2(t) - 1.5708)*sin(th1(t))) + cos(th3(t) - 1.5708)*(1.0*sin(th2(t) - 1.5708)*(1.0*cos(th1(t)) - 2.6536e-6*sin(th1(t))) - 1.3268e-6*cos(th2(t) - 1.5708)*sin(th1(t)))) - 0.02*sin(th5(t))*(sin(th4(t) - 3.1416)*(cos(th3(t) - 1.5708)*(cos(th2(t) - 1.5708)*(1.0*cos(th1(t)) - 2.6536e-6*sin(th1(t))) + 1.3268e-6*sin(th2(t) - 1.5708)*sin(th1(t))) - sin(th3(t) - 1.5708)*(1.0*sin(th2(t) - 1.5708)*(1.0*cos(th1(t)) - 2.6536e-6*sin(th1(t))) - 1.3268e-6*cos(th2(t) - 1.5708)*sin(th1(t)))) - cos(th4(t) - 3.1416)*(1.0*sin(th3(t) - 1.5708)*(cos(th2(t) - 1.5708)*(1.0*cos(th1(t)) - 2.6536e-6*sin(th1(t))) + 1.3268e-6*sin(th2(t) - 1.5708)*sin(th1(t))) + cos(th3(t) - 1.5708)*(1.0*sin(th2(t) - 1.5708)*(1.0*cos(th1(t)) - 2.6536e-6*sin(th1(t))) - 1.3268e-6*cos(th2(t) - 1.5708)*sin(th1(t))))));
